simulink model "simulator_prototype_remade_v1"  (R2021b)
(part 7 of 14)

t3709 = ct{1850};
t371 = ct{1851};
t3713 = ct{1852};
t3715 = ct{1853};
t3716 = ct{1854};
t3717 = ct{1855};
t372 = ct{1856};
t3720 = ct{1857};
t3721 = ct{1858};
t3723 = ct{1859};
t3724 = ct{1860};
t3725 = ct{1861};
t3726 = ct{1862};
t3728 = ct{1863};
t3729 = ct{1864};
t373 = ct{1865};
t3730 = ct{1866};
t3732 = ct{1867};
t3733 = ct{1868};
t3734 = ct{1869};
t3735 = ct{1870};
t3736 = ct{1871};
t3737 = ct{1872};
t3738 = ct{1873};
t374 = ct{1874};
t3743 = ct{1875};
t3744 = ct{1876};
t3745 = ct{1877};
t3746 = ct{1878};
t3747 = ct{1879};
t3750 = ct{1880};
t3752 = ct{1881};
t3756 = ct{1882};
t3757 = ct{1883};
t3758 = ct{1884};
t3766 = ct{1885};
t3768 = ct{1886};
t3769 = ct{1887};
t377 = ct{1888};
t3774 = ct{1889};
t3776 = ct{1890};
t3778 = ct{1891};
t378 = ct{1892};
t3780 = ct{1893};
t3783 = ct{1894};
t3784 = ct{1895};
t3785 = ct{1896};
t3786 = ct{1897};
t3787 = ct{1898};
t3789 = ct{1899};
t379 = ct{1900};
t3792 = ct{1901};
t3795 = ct{1902};
t3798 = ct{1903};
t380 = ct{1904};
t3800 = ct{1905};
t3803 = ct{1906};
t3804 = ct{1907};
t3805 = ct{1908};
t3806 = ct{1909};
t3810 = ct{1910};
t3811 = ct{1911};
t3813 = ct{1912};
t3814 = ct{1913};
t3815 = ct{1914};
t3816 = ct{1915};
t3817 = ct{1916};
t3819 = ct{1917};
t382 = ct{1918};
t3820 = ct{1919};
t3821 = ct{1920};
t3822 = ct{1921};
t3823 = ct{1922};
t3824 = ct{1923};
t3825 = ct{1924};
t3826 = ct{1925};
t3827 = ct{1926};
t3831 = ct{1927};
t3834 = ct{1928};
t3835 = ct{1929};
t3839 = ct{1930};
t384 = ct{1931};
t3843 = ct{1932};
t3849 = ct{1933};
t3850 = ct{1934};
t3851 = ct{1935};
t3852 = ct{1936};
t3853 = ct{1937};
t3855 = ct{1938};
t3857 = ct{1939};
t3858 = ct{1940};
t386 = ct{1941};
t3866 = ct{1942};
t3867 = ct{1943};
t3869 = ct{1944};
t387 = ct{1945};
t3870 = ct{1946};
t3877 = ct{1947};
t388 = ct{1948};
t3885 = ct{1949};
t3889 = ct{1950};
t3890 = ct{1951};
t3891 = ct{1952};
t3892 = ct{1953};
t3899 = ct{1954};
t391 = ct{1955};
t3912 = ct{1956};
t3913 = ct{1957};
t3915 = ct{1958};
t3917 = ct{1959};
t392 = ct{1960};
t3929 = ct{1961};
t3930 = ct{1962};
t3941 = ct{1963};
t3946 = ct{1964};
t3949 = ct{1965};
t395 = ct{1966};
t3950 = ct{1967};
t3951 = ct{1968};
t3952 = ct{1969};
t3953 = ct{1970};
t3958 = ct{1971};
t3959 = ct{1972};
t396 = ct{1973};
t3966 = ct{1974};
t3970 = ct{1975};
t3980 = ct{1976};
t3981 = ct{1977};
t3982 = ct{1978};
t3984 = ct{1979};
t3990 = ct{1980};
t4 = ct{1981};
t400 = ct{1982};
t4004 = ct{1983};
t4005 = ct{1984};
t4006 = ct{1985};
t401 = ct{1986};
t4010 = ct{1987};
t4011 = ct{1988};
t4014 = ct{1989};
t4015 = ct{1990};
t4016 = ct{1991};
t4017 = ct{1992};
t4018 = ct{1993};
t4019 = ct{1994};
t402 = ct{1995};
t4020 = ct{1996};
t4021 = ct{1997};
t4022 = ct{1998};
t4023 = ct{1999};
t4024 = ct{2000};
t4025 = ct{2001};
t4026 = ct{2002};
t4027 = ct{2003};
t4028 = ct{2004};
t4029 = ct{2005};
t403 = ct{2006};
t4036 = ct{2007};
t4039 = ct{2008};
t4040 = ct{2009};
t4041 = ct{2010};
t4042 = ct{2011};
t4045 = ct{2012};
t4046 = ct{2013};
t4047 = ct{2014};
t4048 = ct{2015};
t4051 = ct{2016};
t4053 = ct{2017};
t4054 = ct{2018};
t406 = ct{2019};
t4062 = ct{2020};
t4063 = ct{2021};
t4064 = ct{2022};
t4065 = ct{2023};
t4068 = ct{2024};
t4069 = ct{2025};
t4070 = ct{2026};
t4071 = ct{2027};
t4073 = ct{2028};
t4074 = ct{2029};
t4075 = ct{2030};
t4089 = ct{2031};
t4099 = ct{2032};
t410 = ct{2033};
t4103 = ct{2034};
t4105 = ct{2035};
t411 = ct{2036};
t4113 = ct{2037};
t4114 = ct{2038};
t4116 = ct{2039};
t4118 = ct{2040};
t4119 = ct{2041};
t412 = ct{2042};
t4123 = ct{2043};
t4124 = ct{2044};
t4125 = ct{2045};
t413 = ct{2046};
t4132 = ct{2047};
t414 = ct{2048};
t4140 = ct{2049};
t4142 = ct{2050};
t4143 = ct{2051};
t4144 = ct{2052};
t4145 = ct{2053};
t415 = ct{2054};
t4150 = ct{2055};
t4152 = ct{2056};
t4153 = ct{2057};
t416 = ct{2058};
t4162 = ct{2059};
t4164 = ct{2060};
t4165 = ct{2061};
t4166 = ct{2062};
t4169 = ct{2063};
t417 = ct{2064};
t4171 = ct{2065};
t4173 = ct{2066};
t4174 = ct{2067};
t4177 = ct{2068};
t4178 = ct{2069};
t4179 = ct{2070};
t418 = ct{2071};
t4180 = ct{2072};
t4181 = ct{2073};
t4183 = ct{2074};
t4184 = ct{2075};
t4185 = ct{2076};
t4186 = ct{2077};
t4188 = ct{2078};
t4190 = ct{2079};
t4195 = ct{2080};
t4196 = ct{2081};
t4197 = ct{2082};
t420 = ct{2083};
t4201 = ct{2084};
t4202 = ct{2085};
t4205 = ct{2086};
t4206 = ct{2087};
t4207 = ct{2088};
t4208 = ct{2089};
t4209 = ct{2090};
t4210 = ct{2091};
t4211 = ct{2092};
t4215 = ct{2093};
t4217 = ct{2094};
t4218 = ct{2095};
t4219 = ct{2096};
t422 = ct{2097};
t4220 = ct{2098};
t4221 = ct{2099};
t4223 = ct{2100};
t4224 = ct{2101};
t4225 = ct{2102};
t4226 = ct{2103};
t4228 = ct{2104};
t4229 = ct{2105};
t423 = ct{2106};
t4230 = ct{2107};
t4231 = ct{2108};
t4232 = ct{2109};
t4233 = ct{2110};
t4234 = ct{2111};
t4235 = ct{2112};
t424 = ct{2113};
t4241 = ct{2114};
t4242 = ct{2115};
t4243 = ct{2116};
t4244 = ct{2117};
t4245 = ct{2118};
t4246 = ct{2119};
t4247 = ct{2120};
t4248 = ct{2121};
t4249 = ct{2122};
t425 = ct{2123};
t4250 = ct{2124};
t4251 = ct{2125};
t4253 = ct{2126};
t4254 = ct{2127};
t4255 = ct{2128};
t4256 = ct{2129};
t4257 = ct{2130};
t4258 = ct{2131};
t4259 = ct{2132};
t4260 = ct{2133};
t4261 = ct{2134};
t4262 = ct{2135};
t4263 = ct{2136};
t427 = ct{2137};
t4273 = ct{2138};
t4274 = ct{2139};
t4275 = ct{2140};
t4276 = ct{2141};
t4278 = ct{2142};
t4279 = ct{2143};
t428 = ct{2144};
t4280 = ct{2145};
t4281 = ct{2146};
t4282 = ct{2147};
t4283 = ct{2148};
t4284 = ct{2149};
t4285 = ct{2150};
t4286 = ct{2151};
t4287 = ct{2152};
t4289 = ct{2153};
t429 = ct{2154};
t4290 = ct{2155};
t4291 = ct{2156};
t4292 = ct{2157};
t4293 = ct{2158};
t4295 = ct{2159};
t4296 = ct{2160};
t4297 = ct{2161};
t4298 = ct{2162};
t4299 = ct{2163};
t4300 = ct{2164};
t4301 = ct{2165};
t4302 = ct{2166};
t4303 = ct{2167};
t4304 = ct{2168};
t4305 = ct{2169};
t4306 = ct{2170};
t4308 = ct{2171};
t431 = ct{2172};
t4310 = ct{2173};
t4315 = ct{2174};
t4316 = ct{2175};
t4317 = ct{2176};
t4318 = ct{2177};
t432 = ct{2178};
t4321 = ct{2179};
t4323 = ct{2180};
t4324 = ct{2181};
t4325 = ct{2182};
t4326 = ct{2183};
t4327 = ct{2184};
t4328 = ct{2185};
t4329 = ct{2186};
t433 = ct{2187};
t4330 = ct{2188};
t4331 = ct{2189};
t4332 = ct{2190};
t4333 = ct{2191};
t4334 = ct{2192};
t4335 = ct{2193};
t4336 = ct{2194};
t4337 = ct{2195};
t4338 = ct{2196};
t4339 = ct{2197};
t434 = ct{2198};
t4340 = ct{2199};
t4342 = ct{2200};
t4344 = ct{2201};
t4345 = ct{2202};
t4346 = ct{2203};
t4347 = ct{2204};
t4348 = ct{2205};
t4349 = ct{2206};
t435 = ct{2207};
t4350 = ct{2208};
t4354 = ct{2209};
t4356 = ct{2210};
t4357 = ct{2211};
t436 = ct{2212};
t4362 = ct{2213};
t4363 = ct{2214};
t4365 = ct{2215};
t4366 = ct{2216};
t4368 = ct{2217};
t4369 = ct{2218};
t437 = ct{2219};
t4370 = ct{2220};
t4371 = ct{2221};
t4372 = ct{2222};
t4373 = ct{2223};
t4374 = ct{2224};
t4375 = ct{2225};
t4376 = ct{2226};
t4377 = ct{2227};
t4379 = ct{2228};
t438 = ct{2229};
t4380 = ct{2230};
t4382 = ct{2231};
t4383 = ct{2232};
t4384 = ct{2233};
t4385 = ct{2234};
t4386 = ct{2235};
t4387 = ct{2236};
t4388 = ct{2237};
t4389 = ct{2238};
t439 = ct{2239};
t4391 = ct{2240};
t4392 = ct{2241};
t4394 = ct{2242};
t4395 = ct{2243};
t4396 = ct{2244};
t4397 = ct{2245};
t4398 = ct{2246};
t4399 = ct{2247};
t44 = ct{2248};
t440 = ct{2249};
t4400 = ct{2250};
t4401 = ct{2251};
t4402 = ct{2252};
t4403 = ct{2253};
t4404 = ct{2254};
t4405 = ct{2255};
t4406 = ct{2256};
t4407 = ct{2257};
t4408 = ct{2258};
t4409 = ct{2259};
t441 = ct{2260};
t4410 = ct{2261};
t4411 = ct{2262};
t4412 = ct{2263};
t4413 = ct{2264};
t4414 = ct{2265};
t4415 = ct{2266};
t4416 = ct{2267};
t4417 = ct{2268};
t4418 = ct{2269};
t4419 = ct{2270};
t442 = ct{2271};
t4420 = ct{2272};
t4421 = ct{2273};
t4422 = ct{2274};
t4423 = ct{2275};
t4424 = ct{2276};
t4425 = ct{2277};
t4426 = ct{2278};
t4427 = ct{2279};
t4428 = ct{2280};
t4429 = ct{2281};
t4430 = ct{2282};
t4431 = ct{2283};
t4432 = ct{2284};
t4433 = ct{2285};
t4434 = ct{2286};
t4435 = ct{2287};
t4436 = ct{2288};
t4437 = ct{2289};
t4438 = ct{2290};
t4439 = ct{2291};
t444 = ct{2292};
t4440 = ct{2293};
t4442 = ct{2294};
t4444 = ct{2295};
t4445 = ct{2296};
t4446 = ct{2297};
t4447 = ct{2298};
t4448 = ct{2299};
t4449 = ct{2300};
t445 = ct{2301};
t4450 = ct{2302};
t4451 = ct{2303};
t4453 = ct{2304};
t4454 = ct{2305};
t4455 = ct{2306};
t4460 = ct{2307};
t4461 = ct{2308};
t4462 = ct{2309};
t4463 = ct{2310};
t4464 = ct{2311};
t4465 = ct{2312};
t4466 = ct{2313};
t4467 = ct{2314};
t4468 = ct{2315};
t4469 = ct{2316};
t4470 = ct{2317};
t4471 = ct{2318};
t4473 = ct{2319};
t4474 = ct{2320};
t4475 = ct{2321};
t4476 = ct{2322};
t4477 = ct{2323};
t4478 = ct{2324};
t4479 = ct{2325};
t448 = ct{2326};
t4481 = ct{2327};
t4482 = ct{2328};
t4483 = ct{2329};
t4484 = ct{2330};
t4485 = ct{2331};
t4486 = ct{2332};
t4487 = ct{2333};
t4488 = ct{2334};
t4489 = ct{2335};
t449 = ct{2336};
t4490 = ct{2337};
t4493 = ct{2338};
t4494 = ct{2339};
t4495 = ct{2340};
t4496 = ct{2341};
t4497 = ct{2342};
t4498 = ct{2343};
t4499 = ct{2344};
t45 = ct{2345};
t450 = ct{2346};
t4500 = ct{2347};
t4501 = ct{2348};
t4502 = ct{2349};
t4503 = ct{2350};
t4504 = ct{2351};
t4505 = ct{2352};
t4506 = ct{2353};
t4507 = ct{2354};
t4508 = ct{2355};
t4509 = ct{2356};
t4510 = ct{2357};
t4512 = ct{2358};
t4513 = ct{2359};
t4514 = ct{2360};
t4515 = ct{2361};
t4516 = ct{2362};
t4518 = ct{2363};
t4519 = ct{2364};
t452 = ct{2365};
t4520 = ct{2366};
t4521 = ct{2367};
t4522 = ct{2368};
t4523 = ct{2369};
t4524 = ct{2370};
t4525 = ct{2371};
t4526 = ct{2372};
t4527 = ct{2373};
t4529 = ct{2374};
t453 = ct{2375};
t4530 = ct{2376};
t4531 = ct{2377};
t4532 = ct{2378};
t4534 = ct{2379};
t4535 = ct{2380};
t4537 = ct{2381};
t4538 = ct{2382};
t4539 = ct{2383};
t454 = ct{2384};
t4541 = ct{2385};
t4543 = ct{2386};
t4544 = ct{2387};
t4545 = ct{2388};
t4546 = ct{2389};
t4547 = ct{2390};
t4549 = ct{2391};
t4550 = ct{2392};
t4551 = ct{2393};
t4552 = ct{2394};
t4553 = ct{2395};
t4554 = ct{2396};
t4556 = ct{2397};
t4557 = ct{2398};
t4558 = ct{2399};
t4559 = ct{2400};
t4560 = ct{2401};
t4564 = ct{2402};
t4565 = ct{2403};
t4566 = ct{2404};
t4567 = ct{2405};
t4568 = ct{2406};
t4569 = ct{2407};
t457 = ct{2408};
t4570 = ct{2409};
t4572 = ct{2410};
t4573 = ct{2411};
t4575 = ct{2412};
t4576 = ct{2413};
t4577 = ct{2414};
t4578 = ct{2415};
t458 = ct{2416};
t4580 = ct{2417};
t4581 = ct{2418};
t4582 = ct{2419};
t4584 = ct{2420};
t4586 = ct{2421};
t4587 = ct{2422};
t4588 = ct{2423};
t4589 = ct{2424};
t459 = ct{2425};
t4590 = ct{2426};
t4591 = ct{2427};
t4592 = ct{2428};
t4593 = ct{2429};
t4594 = ct{2430};
t4595 = ct{2431};
t4596 = ct{2432};
t4597 = ct{2433};
t4598 = ct{2434};
t4599 = ct{2435};
t46 = ct{2436};
t460 = ct{2437};
t4600 = ct{2438};
t4601 = ct{2439};
t4602 = ct{2440};
t4603 = ct{2441};
t4604 = ct{2442};
t4605 = ct{2443};
t4606 = ct{2444};
t4607 = ct{2445};
t4608 = ct{2446};
t4609 = ct{2447};
t461 = ct{2448};
t4610 = ct{2449};
t4612 = ct{2450};
t4613 = ct{2451};
t4614 = ct{2452};
t4615 = ct{2453};
t4616 = ct{2454};
t4617 = ct{2455};
t4618 = ct{2456};
t4619 = ct{2457};
t462 = ct{2458};
t4620 = ct{2459};
t4621 = ct{2460};
t4622 = ct{2461};
t4623 = ct{2462};
t4624 = ct{2463};
t4625 = ct{2464};
t4626 = ct{2465};
t4627 = ct{2466};
t4629 = ct{2467};
t463 = ct{2468};
t4631 = ct{2469};
t4632 = ct{2470};
t4633 = ct{2471};
t4634 = ct{2472};
t4635 = ct{2473};
t4636 = ct{2474};
t4637 = ct{2475};
t4638 = ct{2476};
t4639 = ct{2477};
t464 = ct{2478};
t4640 = ct{2479};
t4643 = ct{2480};
t4644 = ct{2481};
t4645 = ct{2482};
t4646 = ct{2483};
t4647 = ct{2484};
t4649 = ct{2485};
t465 = ct{2486};
t4650 = ct{2487};
t4652 = ct{2488};
t4653 = ct{2489};
t4654 = ct{2490};
t4655 = ct{2491};
t4656 = ct{2492};
t4657 = ct{2493};
t4659 = ct{2494};
t466 = ct{2495};
t4660 = ct{2496};
t4661 = ct{2497};
t4662 = ct{2498};
t4663 = ct{2499};
t4664 = ct{2500};
t4665 = ct{2501};
t4666 = ct{2502};
t4667 = ct{2503};
t4668 = ct{2504};
t4669 = ct{2505};
t4670 = ct{2506};
t4671 = ct{2507};
t4672 = ct{2508};
t4673 = ct{2509};
t4674 = ct{2510};
t4675 = ct{2511};
t4676 = ct{2512};
t4677 = ct{2513};
t4678 = ct{2514};
t4679 = ct{2515};
t468 = ct{2516};
t4680 = ct{2517};
t4681 = ct{2518};
t4682 = ct{2519};
t4683 = ct{2520};
t4684 = ct{2521};
t4685 = ct{2522};
t4686 = ct{2523};
t4687 = ct{2524};
t4689 = ct{2525};
t469 = ct{2526};
t4692 = ct{2527};
t4693 = ct{2528};
t4694 = ct{2529};
t4695 = ct{2530};
t4696 = ct{2531};
t4697 = ct{2532};
t4698 = ct{2533};
t4699 = ct{2534};
t47 = ct{2535};
t470 = ct{2536};
t4700 = ct{2537};
t4702 = ct{2538};
t4703 = ct{2539};
t4704 = ct{2540};
t4707 = ct{2541};
t4708 = ct{2542};
t4709 = ct{2543};
t471 = ct{2544};
t4710 = ct{2545};
t4711 = ct{2546};
t4712 = ct{2547};
t4713 = ct{2548};
t4714 = ct{2549};
t4715 = ct{2550};
t4716 = ct{2551};
t4717 = ct{2552};
t4718 = ct{2553};
t4719 = ct{2554};
t472 = ct{2555};
t4720 = ct{2556};
t4721 = ct{2557};
t4722 = ct{2558};
t4723 = ct{2559};
t4724 = ct{2560};
t4725 = ct{2561};
t4726 = ct{2562};
t4727 = ct{2563};
t4728 = ct{2564};
t4729 = ct{2565};
t4730 = ct{2566};
t4731 = ct{2567};
t4732 = ct{2568};
t4733 = ct{2569};
t4734 = ct{2570};
t4736 = ct{2571};
t4737 = ct{2572};
t4738 = ct{2573};
t4739 = ct{2574};
t4740 = ct{2575};
t4742 = ct{2576};
t4745 = ct{2577};
t4746 = ct{2578};
t4747 = ct{2579};
t4748 = ct{2580};
t475 = ct{2581};
t4750 = ct{2582};
t4751 = ct{2583};
t4753 = ct{2584};
t4754 = ct{2585};
t4755 = ct{2586};
t4756 = ct{2587};
t4757 = ct{2588};
t4762 = ct{2589};
t4763 = ct{2590};
t4765 = ct{2591};
t4768 = ct{2592};
t477 = ct{2593};
t4771 = ct{2594};
t4772 = ct{2595};
t4773 = ct{2596};
t4774 = ct{2597};
t4775 = ct{2598};
t4776 = ct{2599};
t4779 = ct{2600};
t4780 = ct{2601};
t4781 = ct{2602};
t4782 = ct{2603};
t4783 = ct{2604};
t4784 = ct{2605};
t4785 = ct{2606};
t4786 = ct{2607};
t4787 = ct{2608};
t4788 = ct{2609};
t4789 = ct{2610};
t479 = ct{2611};
t4790 = ct{2612};
t4791 = ct{2613};
t4792 = ct{2614};
t4793 = ct{2615};
t4794 = ct{2616};
t4795 = ct{2617};
t4797 = ct{2618};
t4799 = ct{2619};
t480 = ct{2620};
t4800 = ct{2621};
t4801 = ct{2622};
t4802 = ct{2623};
t4803 = ct{2624};
t4805 = ct{2625};
t4806 = ct{2626};
t4809 = ct{2627};
t481 = ct{2628};
t4810 = ct{2629};
t4811 = ct{2630};
t4812 = ct{2631};
t4813 = ct{2632};
t4814 = ct{2633};
t4818 = ct{2634};
t4819 = ct{2635};
t482 = ct{2636};
t4820 = ct{2637};
t4821 = ct{2638};
t4824 = ct{2639};
t4825 = ct{2640};
t4826 = ct{2641};
t4827 = ct{2642};
t4829 = ct{2643};
t483 = ct{2644};
t4831 = ct{2645};
t4833 = ct{2646};
t4834 = ct{2647};
t4835 = ct{2648};
t4837 = ct{2649};
t484 = ct{2650};
t4840 = ct{2651};
t4841 = ct{2652};
t4842 = ct{2653};
t4845 = ct{2654};
t4846 = ct{2655};
t4847 = ct{2656};
t4848 = ct{2657};
t485 = ct{2658};
t4851 = ct{2659};
t4853 = ct{2660};
t4856 = ct{2661};
t4857 = ct{2662};
t486 = ct{2663};
t4862 = ct{2664};
t4863 = ct{2665};
t4864 = ct{2666};
t4865 = ct{2667};
t4866 = ct{2668};
t4867 = ct{2669};
t4868 = ct{2670};
t4869 = ct{2671};
t4870 = ct{2672};
t4872 = ct{2673};
t4873 = ct{2674};
t4874 = ct{2675};
t4875 = ct{2676};
t4876 = ct{2677};
t4877 = ct{2678};
t488 = ct{2679};
t4880 = ct{2680};
t4884 = ct{2681};
t4888 = ct{2682};
t489 = ct{2683};
t4893 = ct{2684};
t4895 = ct{2685};
t4903 = ct{2686};
t4904 = ct{2687};
t4907 = ct{2688};
t4908 = ct{2689};
t491 = ct{2690};
t4911 = ct{2691};
t4913 = ct{2692};
t4914 = ct{2693};
t4919 = ct{2694};
t492 = ct{2695};
t4920 = ct{2696};
t4922 = ct{2697};
t4924 = ct{2698};
t4925 = ct{2699};
t4927 = ct{2700};
t4928 = ct{2701};
t4929 = ct{2702};
t493 = ct{2703};
t4931 = ct{2704};
t4933 = ct{2705};
t4934 = ct{2706};
t4935 = ct{2707};
t4936 = ct{2708};
t494 = ct{2709};
t4942 = ct{2710};
t4943 = ct{2711};
t4944 = ct{2712};
t4946 = ct{2713};
t4948 = ct{2714};
t4949 = ct{2715};
t4950 = ct{2716};
t4951 = ct{2717};
t4952 = ct{2718};
t4953 = ct{2719};
t4957 = ct{2720};
t496 = ct{2721};
t4963 = ct{2722};
t4964 = ct{2723};
t4969 = ct{2724};
t497 = ct{2725};
t4970 = ct{2726};
t4973 = ct{2727};
t4974 = ct{2728};
t4975 = ct{2729};
t4976 = ct{2730};
t4978 = ct{2731};
t4979 = ct{2732};
t498 = ct{2733};
t4981 = ct{2734};
t4982 = ct{2735};
t4983 = ct{2736};
t4987 = ct{2737};
t4988 = ct{2738};
t4989 = ct{2739};
t499 = ct{2740};
t4990 = ct{2741};
t4991 = ct{2742};
t4992 = ct{2743};
t4993 = ct{2744};
t4994 = ct{2745};
t4995 = ct{2746};
t4996 = ct{2747};
t5 = ct{2748};
t50 = ct{2749};
t500 = ct{2750};
t5000 = ct{2751};
t5001 = ct{2752};
t5002 = ct{2753};
t5003 = ct{2754};
t5005 = ct{2755};
t5006 = ct{2756};
t5007 = ct{2757};
t5008 = ct{2758};
t5009 = ct{2759};
t501 = ct{2760};
t5010 = ct{2761};
t5014 = ct{2762};
t5015 = ct{2763};
t5016 = ct{2764};
t5017 = ct{2765};
t5018 = ct{2766};
t5019 = ct{2767};
t502 = ct{2768};
t5020 = ct{2769};
t5021 = ct{2770};
t5022 = ct{2771};
t5023 = ct{2772};
t5024 = ct{2773};
t5026 = ct{2774};
t5027 = ct{2775};
t5029 = ct{2776};
t503 = ct{2777};
t5030 = ct{2778};
t5031 = ct{2779};
t5032 = ct{2780};
t5035 = ct{2781};
t5036 = ct{2782};
t5039 = ct{2783};
t504 = ct{2784};
t5041 = ct{2785};
t5045 = ct{2786};
t5048 = ct{2787};
t505 = ct{2788};
t5051 = ct{2789};
t5054 = ct{2790};
t5055 = ct{2791};
t5056 = ct{2792};
t5058 = ct{2793};
t5059 = ct{2794};
t506 = ct{2795};
t5061 = ct{2796};
t5063 = ct{2797};
t5064 = ct{2798};
t5065 = ct{2799};
t5066 = ct{2800};
t5067 = ct{2801};
t507 = ct{2802};
t5073 = ct{2803};
t5074 = ct{2804};
t5075 = ct{2805};
t5076 = ct{2806};
t5077 = ct{2807};
t5078 = ct{2808};
t508 = ct{2809};
t5080 = ct{2810};
t5081 = ct{2811};
t5083 = ct{2812};
t5084 = ct{2813};
t5085 = ct{2814};
t5088 = ct{2815};
t5089 = ct{2816};
t509 = ct{2817};
t5090 = ct{2818};
t5091 = ct{2819};
t5093 = ct{2820};
t5095 = ct{2821};
t5097 = ct{2822};
t5098 = ct{2823};
t5099 = ct{2824};
t510 = ct{2825};
t5100 = ct{2826};
t5101 = ct{2827};
t5102 = ct{2828};
t5107 = ct{2829};
t5109 = ct{2830};
t511 = ct{2831};
t5110 = ct{2832};
t5112 = ct{2833};
t5113 = ct{2834};
t5114 = ct{2835};
t5119 = ct{2836};
t512 = ct{2837};
t5120 = ct{2838};
t5121 = ct{2839};
t5123 = ct{2840};
t5125 = ct{2841};
t513 = ct{2842};
t5131 = ct{2843};
t5132 = ct{2844};
t5136 = ct{2845};
t5138 = ct{2846};
t5139 = ct{2847};
t514 = ct{2848};
t5140 = ct{2849};
t5143 = ct{2850};
t5146 = ct{2851};
t5147 = ct{2852};
t5148 = ct{2853};
t5150 = ct{2854};
t5151 = ct{2855};
t5152 = ct{2856};
t5153 = ct{2857};
t5154 = ct{2858};
t5157 = ct{2859};
t5158 = ct{2860};
t516 = ct{2861};
t5164 = ct{2862};
t5166 = ct{2863};
t517 = ct{2864};
t5171 = ct{2865};
t5172 = ct{2866};
t5174 = ct{2867};
t5175 = ct{2868};
t518 = ct{2869};
t5180 = ct{2870};
t5181 = ct{2871};
t5183 = ct{2872};
t5184 = ct{2873};
t5185 = ct{2874};
t5187 = ct{2875};
t5189 = ct{2876};
t5191 = ct{2877};
t5195 = ct{2878};
t5199 = ct{2879};
t520 = ct{2880};
t5200 = ct{2881};
t5201 = ct{2882};
t5202 = ct{2883};
t5203 = ct{2884};
t5204 = ct{2885};
t5205 = ct{2886};
t5206 = ct{2887};
t5207 = ct{2888};
t5209 = ct{2889};
t521 = ct{2890};
t5210 = ct{2891};
t5211 = ct{2892};
t5215 = ct{2893};
t5216 = ct{2894};
t5217 = ct{2895};
t5218 = ct{2896};
t5219 = ct{2897};
t522 = ct{2898};
t5222 = ct{2899};
t5223 = ct{2900};
t5224 = ct{2901};
t5227 = ct{2902};
t5229 = ct{2903};
t523 = ct{2904};
t5233 = ct{2905};
t5236 = ct{2906};
t5237 = ct{2907};
t5238 = ct{2908};
t5239 = ct{2909};
t524 = ct{2910};
t5240 = ct{2911};
t5242 = ct{2912};
t5244 = ct{2913};
t5247 = ct{2914};
t5248 = ct{2915};
t5249 = ct{2916};
t525 = ct{2917};
t5251 = ct{2918};
t5252 = ct{2919};
t5255 = ct{2920};
t5257 = ct{2921};
t5258 = ct{2922};
t526 = ct{2923};
t5261 = ct{2924};
t5262 = ct{2925};
t5265 = ct{2926};
t5268 = ct{2927};
t5269 = ct{2928};
t527 = ct{2929};
t5270 = ct{2930};
t5272 = ct{2931};
t5279 = ct{2932};
t528 = ct{2933};
t5280 = ct{2934};
t5285 = ct{2935};
t5288 = ct{2936};
t529 = ct{2937};
t5292 = ct{2938};
t5293 = ct{2939};
t5294 = ct{2940};
t5295 = ct{2941};
t5297 = ct{2942};
t53 = ct{2943};
t530 = ct{2944};
t5302 = ct{2945};
t5306 = ct{2946};
t531 = ct{2947};
t5318 = ct{2948};
t532 = ct{2949};
t5320 = ct{2950};
t5321 = ct{2951};
t5324 = ct{2952};
t5327 = ct{2953};
t533 = ct{2954};
t5331 = ct{2955};
t5332 = ct{2956};
t5339 = ct{2957};
t534 = ct{2958};
t5344 = ct{2959};
t5346 = ct{2960};
t5347 = ct{2961};
t5348 = ct{2962};
t5349 = ct{2963};
t535 = ct{2964};
t5351 = ct{2965};
t5355 = ct{2966};
t5356 = ct{2967};
t5358 = ct{2968};
t536 = ct{2969};
t5361 = ct{2970};
t5364 = ct{2971};
t5365 = ct{2972};
t5367 = ct{2973};
t5368 = ct{2974};
t537 = ct{2975};
t5372 = ct{2976};
t5373 = ct{2977};
t5375 = ct{2978};
t5378 = ct{2979};
t538 = ct{2980};
t5383 = ct{2981};
t5387 = ct{2982};
t5389 = ct{2983};
t539 = ct{2984};
t5390 = ct{2985};
t5391 = ct{2986};
t5392 = ct{2987};
t5393 = ct{2988};
t5394 = ct{2989};
t5395 = ct{2990};
t540 = ct{2991};
t5402 = ct{2992};
t5404 = ct{2993};
t5409 = ct{2994};
t5416 = ct{2995};
t5420 = ct{2996};
t543 = ct{2997};
t5433 = ct{2998};
t5435 = ct{2999};
t5436 = ct{3000};
t544 = ct{3001};
t5440 = ct{3002};
t5441 = ct{3003};
t5442 = ct{3004};
t5443 = ct{3005};
t5444 = ct{3006};
t5445 = ct{3007};
t5446 = ct{3008};
t5448 = ct{3009};
t545 = ct{3010};
t5450 = ct{3011};
t5451 = ct{3012};
t5453 = ct{3013};
t5454 = ct{3014};
t5457 = ct{3015};
t5459 = ct{3016};
t546 = ct{3017};
t5463 = ct{3018};
t5464 = ct{3019};
t5465 = ct{3020};
t5466 = ct{3021};
t547 = ct{3022};
t5473 = ct{3023};
t5475 = ct{3024};
t5479 = ct{3025};
t548 = ct{3026};
t5480 = ct{3027};
t5481 = ct{3028};
t5482 = ct{3029};
t5483 = ct{3030};
t5484 = ct{3031};
t5485 = ct{3032};
t5486 = ct{3033};
t5487 = ct{3034};
t5488 = ct{3035};
t5489 = ct{3036};
t549 = ct{3037};
t5490 = ct{3038};
t5491 = ct{3039};
t5492 = ct{3040};
t5493 = ct{3041};
t5494 = ct{3042};
t5496 = ct{3043};
t5498 = ct{3044};
t5499 = ct{3045};
t5501 = ct{3046};
t5507 = ct{3047};
t551 = ct{3048};
t5512 = ct{3049};
t5516 = ct{3050};
t5517 = ct{3051};
t5519 = ct{3052};
t552 = ct{3053};
t5521 = ct{3054};
t5522 = ct{3055};
t5526 = ct{3056};
t5527 = ct{3057};
t553 = ct{3058};
t5534 = ct{3059};
t554 = ct{3060};
t5540 = ct{3061};
t5546 = ct{3062};
t5549 = ct{3063};
t555 = ct{3064};
t5552 = ct{3065};
t5555 = ct{3066};
t5559 = ct{3067};
t556 = ct{3068};
t5561 = ct{3069};
t5562 = ct{3070};
t5563 = ct{3071};
t5565 = ct{3072};
t5566 = ct{3073};
t5569 = ct{3074};
t557 = ct{3075};
t5573 = ct{3076};
t5578 = ct{3077};
t558 = ct{3078};
t5580 = ct{3079};
t5581 = ct{3080};
t5583 = ct{3081};
t5584 = ct{3082};
t5589 = ct{3083};
t559 = ct{3084};
t5590 = ct{3085};
t5593 = ct{3086};
t5594 = ct{3087};
t5596 = ct{3088};
t5597 = ct{3089};
t560 = ct{3090};
t5600 = ct{3091};
t5603 = ct{3092};
t5604 = ct{3093};
t5606 = ct{3094};
t5607 = ct{3095};
t561 = ct{3096};
t5611 = ct{3097};
t5612 = ct{3098};
t5618 = ct{3099};
t562 = ct{3100};
t5629 = ct{3101};
t563 = ct{3102};
t5633 = ct{3103};
t5634 = ct{3104};
t5635 = ct{3105};
t564 = ct{3106};
t5656 = ct{3107};
t5660 = ct{3108};
t5667 = ct{3109};
t5668 = ct{3110};
t567 = ct{3111};
t5673 = ct{3112};
t5678 = ct{3113};
t568 = ct{3114};
t5688 = ct{3115};
t569 = ct{3116};
t57 = ct{3117};
t570 = ct{3118};
t571 = ct{3119};
t572 = ct{3120};
t573 = ct{3121};
t574 = ct{3122};
t5741 = ct{3123};
t5743 = ct{3124};
t576 = ct{3125};
t577 = ct{3126};
t5777 = ct{3127};
t5779 = ct{3128};
t578 = ct{3129};
t5780 = ct{3130};
t5782 = ct{3131};
t579 = ct{3132};
t58 = ct{3133};
t580 = ct{3134};
t581 = ct{3135};
t5818 = ct{3136};
t5819 = ct{3137};
t582 = ct{3138};
t5823 = ct{3139};
t5826 = ct{3140};
t583 = ct{3141};
t584 = ct{3142};
t586 = ct{3143};
t587 = ct{3144};
t5886 = ct{3145};
t5887 = ct{3146};
t589 = ct{3147};
t5894 = ct{3148};
t59 = ct{3149};
t590 = ct{3150};
t591 = ct{3151};
t592 = ct{3152};
t593 = ct{3153};
t594 = ct{3154};
t595 = ct{3155};
t596 = ct{3156};
t597 = ct{3157};
t6 = ct{3158};
t60 = ct{3159};
t600 = ct{3160};
t602 = ct{3161};
t603 = ct{3162};
t604 = ct{3163};
t605 = ct{3164};
t609 = ct{3165};
t610 = ct{3166};
t611 = ct{3167};
t612 = ct{3168};
t613 = ct{3169};
t614 = ct{3170};
t615 = ct{3171};
t616 = ct{3172};
t618 = ct{3173};
t619 = ct{3174};
t620 = ct{3175};
t621 = ct{3176};
t622 = ct{3177};
t623 = ct{3178};
t624 = ct{3179};
t625 = ct{3180};
t626 = ct{3181};
t627 = ct{3182};
t628 = ct{3183};
t629 = ct{3184};
t63 = ct{3185};
t630 = ct{3186};
t631 = ct{3187};
t632 = ct{3188};
t633 = ct{3189};
t634 = ct{3190};
t635 = ct{3191};
t636 = ct{3192};
t637 = ct{3193};
t638 = ct{3194};
t639 = ct{3195};
t640 = ct{3196};
t641 = ct{3197};
t642 = ct{3198};
t643 = ct{3199};
t645 = ct{3200};
t646 = ct{3201};
t647 = ct{3202};
t648 = ct{3203};
t649 = ct{3204};
t650 = ct{3205};
t653 = ct{3206};
t654 = ct{3207};
t655 = ct{3208};
t656 = ct{3209};
t657 = ct{3210};
t658 = ct{3211};
t660 = ct{3212};
t662 = ct{3213};
t663 = ct{3214};
t664 = ct{3215};
t665 = ct{3216};
t667 = ct{3217};
t668 = ct{3218};
t669 = ct{3219};
t673 = ct{3220};
t674 = ct{3221};
t675 = ct{3222};
t676 = ct{3223};
t679 = ct{3224};
t680 = ct{3225};
t681 = ct{3226};
t682 = ct{3227};
t683 = ct{3228};
t684 = ct{3229};
t685 = ct{3230};
t686 = ct{3231};
t687 = ct{3232};
t688 = ct{3233};
t689 = ct{3234};
t691 = ct{3235};
t692 = ct{3236};
t693 = ct{3237};
t694 = ct{3238};
t695 = ct{3239};
t696 = ct{3240};
t697 = ct{3241};
t698 = ct{3242};
t7 = ct{3243};
t700 = ct{3244};
t702 = ct{3245};
t703 = ct{3246};
t704 = ct{3247};
t705 = ct{3248};
t706 = ct{3249};
t708 = ct{3250};
t71 = ct{3251};
t710 = ct{3252};
t711 = ct{3253};
t712 = ct{3254};
t713 = ct{3255};
t7148 = ct{3256};
t715 = ct{3257};
t716 = ct{3258};
t72 = ct{3259};
t724 = ct{3260};
t728 = ct{3261};
t73 = ct{3262};
t731 = ct{3263};
t733 = ct{3264};
t734 = ct{3265};
t735 = ct{3266};
t736 = ct{3267};
t738 = ct{3268};
t739 = ct{3269};
t74 = ct{3270};
t740 = ct{3271};
t741 = ct{3272};
t742 = ct{3273};
t743 = ct{3274};
t744 = ct{3275};
t746 = ct{3276};
t747 = ct{3277};
t748 = ct{3278};
t749 = ct{3279};
t75 = ct{3280};
t750 = ct{3281};
t751 = ct{3282};
t752 = ct{3283};
t753 = ct{3284};
t754 = ct{3285};
t755 = ct{3286};
t756 = ct{3287};
t757 = ct{3288};
t758 = ct{3289};
t759 = ct{3290};
t76 = ct{3291};
t760 = ct{3292};
t762 = ct{3293};
t763 = ct{3294};
t764 = ct{3295};
t765 = ct{3296};
t766 = ct{3297};
t767 = ct{3298};
t768 = ct{3299};
t769 = ct{3300};
t77 = ct{3301};
t772 = ct{3302};
t773 = ct{3303};
t774 = ct{3304};
t775 = ct{3305};
t776 = ct{3306};
t777 = ct{3307};
t778 = ct{3308};
t779 = ct{3309};
t780 = ct{3310};
t781 = ct{3311};
t782 = ct{3312};
t784 = ct{3313};
t785 = ct{3314};
t786 = ct{3315};
t792 = ct{3316};
t794 = ct{3317};
t795 = ct{3318};
t796 = ct{3319};
t797 = ct{3320};
t798 = ct{3321};
t799 = ct{3322};
t8 = ct{3323};
t80 = ct{3324};
t801 = ct{3325};
t802 = ct{3326};
t804 = ct{3327};
t805 = ct{3328};
t806 = ct{3329};
t808 = ct{3330};
t81 = ct{3331};
t814 = ct{3332};
t815 = ct{3333};
t817 = ct{3334};
t82 = ct{3335};
t820 = ct{3336};
t822 = ct{3337};
t823 = ct{3338};
t824 = ct{3339};
t825 = ct{3340};
t826 = ct{3341};
t827 = ct{3342};
t829 = ct{3343};
t83 = ct{3344};
t830 = ct{3345};
t831 = ct{3346};
t832 = ct{3347};
t833 = ct{3348};
t834 = ct{3349};
t835 = ct{3350};
t836 = ct{3351};
t837 = ct{3352};
t838 = ct{3353};
t84 = ct{3354};
t840 = ct{3355};
t841 = ct{3356};
t842 = ct{3357};
t843 = ct{3358};
t844 = ct{3359};
t845 = ct{3360};
t846 = ct{3361};
t847 = ct{3362};
t852 = ct{3363};
t853 = ct{3364};
t856 = ct{3365};
t858 = ct{3366};
t859 = ct{3367};
t86 = ct{3368};
t861 = ct{3369};
t863 = ct{3370};
t865 = ct{3371};
t866 = ct{3372};
t867 = ct{3373};
t868 = ct{3374};
t869 = ct{3375};
t870 = ct{3376};
t874 = ct{3377};
t875 = ct{3378};
t876 = ct{3379};
t877 = ct{3380};
t878 = ct{3381};
t880 = ct{3382};
t881 = ct{3383};
t882 = ct{3384};
t884 = ct{3385};
t885 = ct{3386};
t888 = ct{3387};
t891 = ct{3388};
t895 = ct{3389};
t899 = ct{3390};
t9 = ct{3391};
t90 = ct{3392};
t900 = ct{3393};
t902 = ct{3394};
t903 = ct{3395};
t906 = ct{3396};
t909 = ct{3397};
t91 = ct{3398};
t910 = ct{3399};
t911 = ct{3400};
t914 = ct{3401};
t916 = ct{3402};
t917 = ct{3403};
t920 = ct{3404};
t921 = ct{3405};
t922 = ct{3406};
t923 = ct{3407};
t925 = ct{3408};
t926 = ct{3409};
t927 = ct{3410};
t928 = ct{3411};
t929 = ct{3412};
t930 = ct{3413};
t934 = ct{3414};
t935 = ct{3415};
t937 = ct{3416};
t940 = ct{3417};
t941 = ct{3418};
t942 = ct{3419};
t943 = ct{3420};
t944 = ct{3421};
t945 = ct{3422};
t946 = ct{3423};
t947 = ct{3424};
t949 = ct{3425};
t95 = ct{3426};
t950 = ct{3427};
t951 = ct{3428};
t952 = ct{3429};
t953 = ct{3430};
t954 = ct{3431};
t955 = ct{3432};
t957 = ct{3433};
t958 = ct{3434};
t961 = ct{3435};
t962 = ct{3436};
t963 = ct{3437};
t964 = ct{3438};
t965 = ct{3439};
t968 = ct{3440};
t97 = ct{3441};
t970 = ct{3442};
t971 = ct{3443};
t972 = ct{3444};
t973 = ct{3445};
t974 = ct{3446};
t975 = ct{3447};
t976 = ct{3448};
t977 = ct{3449};
t982 = ct{3450};
t983 = ct{3451};
t984 = ct{3452};
t986 = ct{3453};
t987 = ct{3454};
t988 = ct{3455};
t989 = ct{3456};
t99 = ct{3457};
t991 = ct{3458};
t993 = ct{3459};
t994 = ct{3460};
t995 = ct{3461};
t999 = ct{3462};
t1723 = -t1649;
t1741 = -t1665;
t1747 = t202.*6.45106415957158e-10;
t1753 = t7.*t199.*3.023531158253378e-8;
t1754 = t5.*t9.*t199.*4.188279553614573e-7;
t1765 = t5.*t199.*(-2.227142959217101e-7);
t1766 = t5.*t199.*(-1.11357147960855e-7);
t1768 = t8.*t9.*t201.*4.454285918434201e-7;
t1777 = t5.*t9.*t201.*1.274380648825446e-6;
t1781 = -t1706;
t1790 = t8.*t19.*t201.*8.376559107229145e-7;
t1794 = t7.*t9.*t200.*1.378434177095879e-6;
t1805 = t7.*t8.*t199.*1.435017073119793e-6;
t1815 = -t1719;
t1845 = t19.*t199.*6.371903244127231e-7;
t1846 = t19.*t199.*1.274380648825446e-6;
t1848 = t18.*t1551;
t1853 = -t1743;
t1856 = t17.*t1557;
t1861 = t19.*t202.*6.371903244127231e-7;
t1885 = -t1773;
t1886 = -t1775;
t1891 = -t1782;
t1900 = -t1792;
t1902 = t5.*t7.*t9.*t200.*2.817872251232979e-6;
t1905 = -t1802;
t1917 = t199.*3.179500557904044e-7;
t1918 = t199.*6.359001115808088e-7;
t1927 = t5.*t200.*1.608000198040319e-13;
t1928 = -t1825;
t1934 = t202.*3.179500557904044e-7;
t1942 = t199.*3.173049493744472e-7;
t1947 = t18.*t1590;
t1951 = -t1854;
t1952 = t7.*t200.*4.340272528010248e-9;
t1953 = -t1862;
t1954 = t23.*t1590;
t1975 = t18.*t1665;
t1982 = t18.*t1671;
t1983 = t7.*t19.*t200.*4.287013106293682e-6;
t1985 = t18.*t1673;
t1986 = t5.*t7.*t8.*t199.*1.378434177095879e-6;
t1987 = -t1880;
t1989 = t9.*t201.*t306;
t1991 = t18.*t1615;
t2011 = -t1904;
t2015 = t17.*t1624;
t2018 = t18.*t1627;
t2026 = t5.*t200.*8.040000990201593e-14;
t2027 = t5.*t201.*8.040000990201593e-14;
t2035 = t18.*t1630;
t2043 = t8.*t24.*t199.*6.371903244127231e-7;
t2045 = t23.*t1630;
t2049 = t9.*t202.*8.040000990201593e-14;
t2050 = t18.*t1642;
t2075 = t5.*t7.*t200.*7.492102979241942e-7;
t2090 = -t1973;
t2123 = t8.*t9.*t199.*3.216000396080637e-13;
t2127 = -t2021;
t2134 = t8.*t19.*t199.*(-6.371903244127231e-7);
t2137 = -t2041;
t2138 = -t2044;
t2143 = -t2047;
t2146 = -t2055;
t2152 = -t2080;
t2160 = t8.*t201.*1.508157382287566e-7;
t2161 = t8.*t201.*3.016314764575132e-7;
t2164 = t7.*t200.*2.139166280618831e-6;
t2165 = t18.*t1759;
t2181 = t5.*t7.*t8.*t9.*t199.*2.143506553146841e-6;
t2193 = t5.*t7.*t199.*5.4093083807222e-13;
t2197 = -t2139;
t2198 = -t2141;
t2199 = -t2140;
t2202 = t7.*t8.*t19.*t199.*1.408936125616489e-6;
t2211 = t18.*t1822;
t2213 = t7.*t8.*t9.*t199.*7.492102979241942e-7;
t2215 = t18.*t1825;
t2216 = t22.*t1823;
t2222 = t18.*t1837;
t2224 = -t2150;
t2230 = -t2088;
t2238 = -t2162;
t2241 = -t2163;
t2247 = -t2167;
t2248 = -t2168;
t2253 = -t2177;
t2258 = -t2192;
t2259 = t9.*t200.*1.054342951111095e-13;
t2260 = t9.*t200.*2.10868590222219e-13;
t2261 = t9.*t201.*1.054342951111095e-13;
t2262 = t5.*t202.*1.054342951111095e-13;
t2263 = -t2195;
t2268 = -t2210;
t2288 = -t2250;
t2289 = t5.*t8.*t199.*4.217371804444381e-13;
t2290 = -t2252;
t2293 = t5.*t201.*4.300660646822946e-14;
t2296 = t9.*t201.*4.300660646822946e-14;
t2301 = t8.*t201.*5.773966567786041e-7;
t2303 = t7.*t8.*t199.*5.073437414621283e-7;
t2313 = t17.*t2147;
t2315 = t22.*t2147;
t2319 = -t2287;
t2320 = t7.*t9.*t199.*7.093613755211269e-13;
t2326 = t199.*t544;
t2327 = -t2292;
t2345 = -t2309;
t2346 = -t2314;
t2367 = -t2335;
t2383 = t199.*t572;
t2386 = -t2351;
t2393 = t17.*t2255;
t2398 = t22.*t2255;
t2404 = -t2368;
t2408 = -t2381;
t2416 = t199.*t595;
t2420 = -t2390;
t2424 = -t2395;
t2426 = -t2397;
t2448 = -t2423;
t2465 = t8.*t199.*7.452372645815517e-7;
t2479 = -t2471;
t2490 = -t2480;
t2494 = -t2482;
t2534 = -t2509;
t2542 = -t2524;
t2547 = -t2532;
t2594 = -t2580;
t2613 = t6.*t202.*5.463144604697158e-2;
t2614 = t9.*t2582;
t2620 = t2.*t199.*1.324388487819695e-2;
t2621 = t5.*t2585;
t2622 = t2.*t200.*1.324388487819695e-2;
t2623 = t2.*t201.*1.324388487819695e-2;
t2624 = t9.*t2585;
t2625 = t5.*t2586;
t2626 = t5.*t2587;
t2628 = t2.*t202.*1.324388487819695e-2;
t2629 = t6.*t201.*1.324388487819695e-2;
t2630 = t9.*t2586;
t2631 = t9.*t2587;
t2632 = t6.*t202.*1.324388487819695e-2;
t2642 = t5.*t2580;
t2643 = t2.*t201.*5.463144604697158e-2;
t2644 = t6.*t199.*5.463144604697158e-2;
t2645 = t9.*t2580;
t2646 = t5.*t2581;
t2647 = t2.*t202.*5.463144604697158e-2;
t2648 = t6.*t200.*5.463144604697158e-2;
t2649 = t6.*t201.*5.463144604697158e-2;
t2650 = t9.*t2581;
t2651 = t5.*t2582;
t2657 = t199.*8.76226105503051e-2;
t2658 = t5.*t2600;
t2660 = t200.*8.76226105503051e-2;
t2661 = t201.*8.76226105503051e-2;
t2662 = t9.*t2600;
t2663 = t5.*t2601;
t2664 = t202.*8.76226105503051e-2;
t2665 = t9.*t2601;
t2689 = t2.*t199.*3.46332667728404e-6;
t2729 = t2.*t5.*t200.*(-1.324388487819695e-2);
t2736 = -t2703;
t2737 = -t2702;
t2738 = t6.*t9.*t202.*(-1.324388487819695e-2);
t2740 = t199.*1.182954431201322e-5;
t2745 = t5.*t200.*4.081996247155408e-7;
t2746 = t2.*t5.*t202.*(-5.463144604697158e-2);
t2747 = t5.*t6.*t200.*(-5.463144604697158e-2);
t2750 = t6.*t199.*1.428633261714363e-5;
t2753 = t2.*t9.*t200.*1.73166333864202e-6;
t2754 = t2.*t9.*t200.*3.46332667728404e-6;
t2755 = t2.*t5.*t202.*1.73166333864202e-6;
t2756 = t2.*t5.*t202.*3.46332667728404e-6;
t2757 = t5.*t6.*t200.*1.73166333864202e-6;
t2758 = t5.*t6.*t200.*3.46332667728404e-6;
t2763 = t5.*t200.*(-8.76226105503051e-2);
t2765 = -t2733;
t2766 = -t2734;
t2767 = -t2739;
t2772 = t199.*6.433028743309294e-4;
t2778 = t2.*t5.*t199.*1.73166333864202e-6;
t2780 = t2.*t199.*1.882396747564322e-6;
t2785 = t6.*t199.*7.764946411068142e-6;
t2790 = t9.*t200.*2.218657717048192e-7;
t2793 = t5.*t199.*5.914772156006612e-6;
t2795 = t200.*6.003953432070899e-6;
t2796 = t200.*1.20079068641418e-5;
t2797 = t200.*4.200697734379648e-9;
t2798 = t200.*8.401395468759295e-9;
t2799 = -t2768;
t2800 = t9.*t200.*5.914772156006612e-6;
t2801 = t9.*t200.*1.182954431201322e-5;
t2802 = t5.*t202.*5.914772156006612e-6;
t2803 = t5.*t202.*1.182954431201322e-5;
t2805 = -t2773;
t2807 = t199.*6.429626140715183e-6;
t2809 = -t2776;
t2810 = t2.*t5.*t200.*7.143166308571814e-6;
t2811 = t2.*t5.*t200.*1.428633261714363e-5;
t2812 = t5.*t6.*t199.*7.143166308571814e-6;
t2814 = t199.*5.475413853010983e-6;
t2816 = t6.*t9.*t200.*7.143166308571814e-6;
t2817 = t6.*t9.*t200.*1.428633261714363e-5;
t2818 = t5.*t6.*t202.*7.143166308571814e-6;
t2819 = t5.*t6.*t202.*1.428633261714363e-5;
t2822 = t2.*t5.*t199.*(-3.46332667728404e-6);
t2823 = -t2782;
t2824 = -t2781;
t2825 = t2.*t9.*t202.*9.41198373782161e-7;
t2826 = t2.*t9.*t202.*1.882396747564322e-6;
t2827 = t6.*t9.*t200.*9.41198373782161e-7;
t2828 = t6.*t9.*t200.*1.882396747564322e-6;
t2832 = -t2787;
t2833 = -t2786;
t2834 = -t2789;
t2835 = -t2788;
t2837 = t7.*t199.*7.725649335384969e-9;
t2838 = t7.*t199.*1.545129867076994e-8;
t2839 = t5.*t199.*(-1.182954431201322e-5);
t2841 = t5.*t200.*6.433028743309294e-4;
t2843 = t9.*t200.*6.433028743309294e-4;
t2846 = -t2808;
t2852 = t5.*t6.*t199.*(-1.428633261714363e-5);
t2857 = t2.*t9.*t199.*9.41198373782161e-7;
t2859 = t2.*t5.*t200.*9.41198373782161e-7;
t2860 = t2.*t5.*t200.*1.882396747564322e-6;
t2865 = t200.*3.221288775573066e-7;
t2867 = -t2821;
t2870 = t2.*t9.*t200.*3.882473205534071e-6;
t2871 = t2.*t9.*t200.*7.764946411068142e-6;
t2872 = t6.*t9.*t199.*3.882473205534071e-6;
t2874 = t5.*t6.*t200.*3.882473205534071e-6;
t2875 = t5.*t6.*t200.*7.764946411068142e-6;
t2876 = t2.*t199.*2.733068497907686e-6;
t2877 = t6.*t9.*t202.*3.882473205534071e-6;
t2878 = t6.*t9.*t202.*7.764946411068142e-6;
t2882 = t2.*t202.*2.733068497907686e-6;
t2883 = t6.*t200.*2.733068497907686e-6;
t2885 = -t2840;
t2891 = t5.*t200.*6.429626140715183e-6;
t2893 = -t2847;
t2894 = t9.*t202.*6.429626140715183e-6;
t2895 = -t2848;
t2896 = -t2849;
t2897 = -t2853;
t2904 = t2.*t9.*t199.*(-1.882396747564322e-6);
t2907 = -t2862;
t2910 = -t2866;
t2911 = -t2868;
t2914 = t6.*t9.*t199.*(-7.764946411068142e-6);
t2918 = t2.*t199.*1.366534248953843e-6;
t2919 = -t2879;
t2921 = t2.*t202.*1.366534248953843e-6;
t2922 = t6.*t200.*1.366534248953843e-6;
t2931 = t9.*t199.*(-6.429626140715183e-6);
t2932 = t9.*t199.*3.214813070357591e-6;
t2934 = t5.*t200.*3.214813070357591e-6;
t2941 = t9.*t202.*3.214813070357591e-6;
t2942 = -t2898;
t2944 = -t2899;
t2946 = -t2901;
t2947 = -t2902;
t2954 = t2.*t200.*5.636997208875202e-6;
t2955 = t2.*t200.*1.12739944177504e-5;
t2956 = t6.*t199.*5.636997208875202e-6;
t2957 = t6.*t199.*1.12739944177504e-5;
t2958 = t6.*t202.*5.636997208875202e-6;
t2959 = t6.*t202.*1.12739944177504e-5;
t2965 = t202.*7.405322476003771e-6;
t2972 = -t2926;
t2973 = t199.*4.66761554949828e-6;
t2974 = t199.*9.33523109899656e-6;
t2977 = t202.*4.66761554949828e-6;
t2978 = t202.*9.33523109899656e-6;
t2994 = -t2943;
t2995 = -t2948;
t3001 = -t2960;
t3002 = -t2961;
t3005 = -t2963;
t3008 = -t2964;
t3009 = t8.*t2926;
t3018 = -t2976;
t3022 = -t2982;
t3037 = t18.*t2898;
t3040 = t8.*t17.*t2820;
t3041 = t8.*t2962;
t3042 = t8.*t2963;
t3044 = t8.*t22.*t2820;
t3048 = -t3003;
t3049 = -t3004;
t3050 = t8.*t2968;
t3054 = t8.*t2975;
t3059 = t3.*t4.*t7.*t2820;
t3064 = -t3023;
t3067 = -t3027;
t3068 = -t3028;
t3074 = -t3038;
t3076 = -t3039;
t3081 = -t3045;
t3084 = t8.*t3024;
t3086 = -t3062;
t3088 = -t3063;
t3089 = t18.*t2926;
t3096 = -t3075;
t3097 = -t3078;
t3100 = t17.*t18.*t2820;
t3101 = t17.*t18.*t2821;
t3102 = t2.*t5.*t200.*3.634948345122482e-13;
t3106 = t17.*t18.*t2784;
t3107 = t2.*t9.*t200.*3.634948345122482e-13;
t3110 = -t3087;
t3114 = -t3091;
t3117 = -t3093;
t3118 = -t3094;
t3121 = -t3099;
t3122 = t18.*t3004;
t3128 = -t3105;
t3134 = t2151./8.112963841460668e+31;
t3135 = t5.*t6.*t200.*1.499427745155113e-12;
t3136 = t2088./8.112963841460668e+31;
t3137 = t18.*t3024;
t3138 = t6.*t9.*t200.*1.499427745155113e-12;
t3141 = t5.*t200.*1.241574547458694e-12;
t3144 = t9.*t200.*1.241574547458694e-12;
t3153 = -t3123;
t3154 = -t3130;
t3169 = -t3145;
t3175 = -t3151;
t3176 = -t3152;
t3179 = t8.*t3132;
t3185 = -t3165;
t3188 = -t3173;
t3189 = t199.*4.143543013549434e-7;
t3192 = -t3177;
t3193 = -t3178;
t3195 = t8.*t3160;
t3196 = -t3186;
t3198 = -t3190;
t3200 = t2.*t200.*1.7577726911557e-6;
t3201 = t2.*t200.*3.5155453823114e-6;
t3202 = t2.*t201.*1.7577726911557e-6;
t3203 = t2.*t201.*3.5155453823114e-6;
t3204 = t6.*t199.*1.7577726911557e-6;
t3205 = t6.*t199.*3.5155453823114e-6;
t3209 = t2.*t199.*7.250868217512499e-6;
t3210 = t2.*t199.*1.4501736435025e-5;
t3213 = t6.*t200.*7.250868217512499e-6;
t3214 = t6.*t200.*1.4501736435025e-5;
t3215 = t6.*t201.*7.250868217512499e-6;
t3216 = t6.*t201.*1.4501736435025e-5;
t3217 = -t3197;
t3226 = t200.*1.200790562256725e-5;
t3227 = t201.*1.200790562256725e-5;
t3229 = -t3206;
t3232 = -t3207;
t3233 = t8.*t3197;
t3235 = t201.*1.200790624335452e-5;
t3247 = t200.*6.003952811283625e-6;
t3249 = t201.*6.003952811283625e-6;
t3267 = -t3241;
t3269 = -t3250;
t3270 = -t3253;
t3271 = -t3254;
t3322 = -t3291;
t3323 = -t3292;
t3332 = t5.*t3277;
t3336 = t9.*t3277;
t3337 = t8.*t3278;
t3340 = t9.*t3280;
t3341 = t5.*t3260;
t3344 = t9.*t3260;
t3349 = t5.*t3296;
t3351 = t9.*t3296;
t3352 = t8.*t3298;
t3353 = t9.*t3299;
t3354 = t8.*t3303;
t3355 = t9.*t3304;
t3356 = t5.*t3307;
t3357 = t9.*t3307;
t3358 = t8.*t3308;
t3359 = t9.*t3310;
t3360 = t8.*t3313;
t3361 = t9.*t3315;
t3385 = t4.*t3339;
t3386 = t8.*t3338;
t3388 = t8.*t3339;
t3428 = t18.*t3339;
t3429 = t23.*t3339;
t3448 = t8.*t3387;
t3460 = -t3423;
t3461 = -t3427;
t3478 = t8.*t3406;
t3482 = t4.*t3412;
t3484 = t8.*t3412;
t3526 = t8.*t3480;
t3537 = t18.*t3412;
t3540 = t23.*t3412;
t3561 = t2.*t201.*1.769880715106441e-6;
t3565 = t2.*t202.*1.769880715106441e-6;
t3566 = t6.*t201.*1.769880715106441e-6;
t3570 = -t3545;
t3588 = t2.*t199.*1.769880715106441e-6;
t3594 = t5.*t200.*2.086042441322004e-7;
t3595 = t5.*t201.*2.086042441322004e-7;
t3598 = -t3567;
t3600 = t9.*t202.*2.086042441322004e-7;
t3623 = t2.*t201.*7.30081420113316e-6;
t3624 = t6.*t199.*7.30081420113316e-6;
t3626 = t6.*t9.*t202.*1.769880715106441e-6;
t3632 = t6.*t201.*7.30081420113316e-6;
t3640 = t6.*t202.*7.30081420113316e-6;
t3664 = -t3608;
t3669 = -t3614;
t3670 = -t3615;
t3671 = t2.*t9.*t200.*1.769880715106441e-6;
t3674 = t5.*t6.*t200.*1.769880715106441e-6;
t3677 = -t3620;
t3678 = -t3619;
t3679 = t2.*t9.*t202.*(-1.769880715106441e-6);
t3685 = t6.*t9.*t202.*8.849403575532204e-7;
t3692 = t199.*6.367841787827598e-4;
t3698 = t201.*6.367841787827598e-4;
t3703 = t202.*6.367841787827598e-4;
t3711 = t25.*t3527;
t3712 = t25.*t3528;
t3718 = t26.*t3527;
t3719 = t26.*t3528;
t3727 = t199.*1.170967356229242e-5;
t3731 = t201.*1.170967356229242e-5;
t3739 = t9.*t200.*1.133811468776912e-7;
t3740 = t9.*t201.*1.133811468776912e-7;
t3741 = t5.*t202.*1.133811468776912e-7;
t3742 = t202.*1.170967356229242e-5;
t3753 = t2.*t9.*t200.*8.849403575532204e-7;
t3754 = t2.*t9.*t201.*(-1.769880715106441e-6);
t3755 = t2.*t9.*t201.*8.849403575532204e-7;
t3759 = t2.*t9.*t202.*3.65040710056658e-6;
t3760 = t2.*t9.*t202.*7.30081420113316e-6;
t3761 = t6.*t9.*t200.*3.65040710056658e-6;
t3762 = t6.*t9.*t200.*7.30081420113316e-6;
t3763 = t6.*t9.*t201.*3.65040710056658e-6;
t3772 = -t3688;
t3775 = t2.*t199.*9.619703863182361e-7;
t3777 = -t3693;
t3779 = t2.*t201.*9.619703863182361e-7;
t3781 = t2.*t202.*9.619703863182361e-7;
t3782 = t6.*t201.*9.619703863182361e-7;
t3788 = t25.*t3550;
t3790 = t199.*5.419930569269819e-6;
t3791 = t26.*t3550;
t3793 = t201.*5.419930569269819e-6;
t3794 = -t3721;
t3796 = -t3723;
t3797 = t202.*5.419930569269819e-6;
t3801 = t2.*t201.*3.96815841743287e-6;
t3802 = t6.*t199.*3.96815841743287e-6;
t3812 = t6.*t201.*3.96815841743287e-6;
t3818 = t6.*t202.*3.96815841743287e-6;
t3828 = t2.*t5.*t200.*7.30081420113316e-6;
t3833 = t6.*t9.*t201.*(-7.30081420113316e-6);
t3836 = t6.*t9.*t202.*(-7.30081420113316e-6);
t3837 = t5.*t200.*6.367841787827598e-4;
t3840 = t9.*t200.*6.367841787827598e-4;
t3845 = -t3776;
t3854 = t8.*t3721;
t3856 = t199.*6.364473664374288e-6;
t3860 = t200.*1.646190906295504e-7;
t3861 = t201.*1.646190906295504e-7;
t3862 = t8.*t3724;
t3863 = t5.*t199.*5.85483678114621e-6;
t3865 = t201.*6.364473664374288e-6;
t3868 = t202.*6.364473664374288e-6;
t3871 = t9.*t200.*5.85483678114621e-6;
t3872 = t9.*t200.*1.170967356229242e-5;
t3873 = t9.*t201.*5.85483678114621e-6;
t3875 = t5.*t202.*5.85483678114621e-6;
t3881 = -t3804;
t3882 = -t3803;
t3883 = -t3805;
t3884 = -t3806;
t3886 = t200.*1.18862287368685e-5;
t3887 = t201.*1.18862287368685e-5;
t3888 = -t3817;
t3893 = t202.*1.18862287368685e-5;
t3894 = -t3826;
t3895 = -t3827;
t3897 = t2.*t5.*t201.*(-7.30081420113316e-6);
t3901 = t2.*t5.*t200.*4.809851931591181e-7;
t3902 = t2.*t5.*t200.*9.619703863182361e-7;
t3903 = t2.*t5.*t201.*4.809851931591181e-7;
t3908 = t6.*t9.*t200.*9.619703863182361e-7;
t3910 = t5.*t6.*t202.*4.809851931591181e-7;
t3911 = t5.*t6.*t202.*9.619703863182361e-7;
t3914 = t9.*t202.*(-6.367841787827598e-4);
t3916 = t2.*t199.*1.396693317797299e-6;
t3918 = -t3855;
t3921 = -t3858;
t3922 = -t3857;
C_dq = ft_10({dq1,dq2,dq3,dq4,dq5,dq6,t1004,t1006,t1008,t101,t1013,t1016,t1017,t1019,t102,t1020,t1021,t1023,t1024,t1025,t1026,t1028,t1030,t1032,t1034,t1036,t1038,t1039,t1040,t1042,t1043,t1044,t1045,t1046,t1047,t1048,t1049,t1050,t1051,t1054,t1055,t1056,t1057,t1059,t1061,t1065,t1066,t1068,t1069,t1070,t1072,t1073,t1075,t1076,t1077,t1081,t1083,t1084,t1085,t1087,t1089,t1091,t1092,t1093,t1095,t1098,t1099,t110,t1101,t1102,t1105,t1106,t1107,t1108,t1109,t111,t1113,t1115,t1116,t1119,t112,t1122,t1125,t1126,t1127,t1128,t113,t1130,t1131,t1133,t1134,t1135,t1138,t1139,t114,t1141,t1144,t1145,t1146,t1147,t1148,t1149,t115,t1150,t1152,t1153,t1155,t1158,t1159,t116,t1162,t1163,t1165,t1167,t1169,t1170,t1171,t1173,t1174,t1175,t1177,t1178,t1179,t1180,t1181,t1182,t1183,t1184,t1185,t1186,t1188,t1189,t1190,t1191,t1192,t1193,t1194,t1196,t1197,t1198,t1199,t120,t1200,t1202,t1203,t1204,t1205,t1206,t1207,t121,t1210,t1211,t1215,t1219,t1221,t1222,t1224,t1225,t1227,t1228,t1233,t1235,t1236,t1237,t1239,t124,t1240,t1241,t1244,t1245,t125,t1250,t1251,t1253,t1254,t1256,t1257,t1258,t1259,t126,t1261,t1262,t1263,t1264,t1265,t1266,t1267,t1268,t1269,t1271,t1272,t1273,t1274,t1277,t1278,t128,t1280,t1282,t1285,t1286,t1288,t129,t1290,t1293,t1294,t1295,t1296,t1298,t1300,t1301,t1302,t1306,t1307,t1308,t1309,t131,t1311,t1312,t1313,t1315,t1316,t1317,t1318,t1319,t132,t1322,t1323,t1324,t1325,t1326,t1328,t1329,t133,t1330,t1331,t1333,t1334,t1337,t1338,t1340,t1341,t1342,t1343,t1344,t1345,t1346,t1348,t1351,t1352,t1353,t1354,t1355,t1356,t1360,t1362,t1365,t1366,t1367,t1369,t1370,t1371,t1372,t1374,t1375,t1377,t1378,t1379,t1380,t1383,t1384,t1385,t1386,t1388,t1389,t139,t1391,t1392,t1393,t1394,t1397,t1398,t140,t1401,t1402,t1403,t1404,t1406,t1407,t1408,t1409,t141,t1410,t1411,t1413,t1414,t1415,t1416,t1417,t1419,t142,t1422,t1423,t1426,t1427,t1428,t1429,t1430,t1431,t1432,t1433,t1436,t144,t1440,t1441,t1442,t1443,t1445,t1446,t1447,t1448,t1449,t1451,t1452,t1453,t1454,t1455,t1456,t1457,t1458,t1459,t1460,t1463,t1464,t1465,t1467,t1470,t1471,t1474,t1476,t1478,t1479,t148,t1480,t1481,t1482,t1483,t1486,t1487,t1488,t1489,t1490,t1491,t1492,t1493,t1494,t1495,t1496,t1498,t1499,t15,t150,t1500,t1501,t1503,t1505,t1506,t1507,t1508,t1509,t151,t1510,t1511,t1512,t1513,t1515,t1517,t1520,t1521,t1522,t1523,t1524,t1526,t1527,t1529,t153,t1530,t1531,t1532,t1533,t1534,t1535,t1536,t1537,t1538,t1539,t154,t1540,t1541,t1542,t1548,t1549,t1550,t1551,t1553,t1558,t156,t1560,t1561,t1562,t1564,t1566,t1567,t1568,t157,t1570,t1571,t1572,t1574,t1575,t1576,t1577,t1578,t1579,t158,t1580,t1581,t1582,t1583,t1584,t1585,t1586,t1587,t1589,t1590,t1591,t1592,t1593,t1594,t1595,t1596,t1597,t1598,t1599,t16,t1601,t1602,t1605,t1606,t1607,t1609,t161,t1610,t1611,t1612,t1613,t1614,t1615,t1616,t1617,t1618,t1619,t1620,t1621,t1622,t1625,t1626,t1627,t163,t1630,t1631,t1632,t1633,t1635,t1636,t1637,t1638,t1639,t1641,t1642,t1643,t1644,t1645,t1646,t1647,t1648,t165,t1651,t1652,t1653,t1657,t1658,t1659,t166,t1660,t1661,t1662,t1663,t1666,t1667,t1669,t1670,t1671,t1672,t1673,t1674,t1675,t1676,t1681,t1682,t1683,t1686,t1687,t1689,t1691,t1692,t1696,t1697,t1698,t1699,t17,t170,t1700,t1701,t1702,t1703,t1704,t1705,t1706,t1709,t171,t1710,t1711,t1712,t1713,t1715,t1716,t1718,t1719,t1720,t1721,t1722,t1723,t1724,t1726,t1728,t1729,t1731,t1733,t1734,t1735,t1736,t1737,t1738,t1739,t1740,t1741,t1745,t1746,t1747,t1748,t1749,t1752,t1753,t1754,t1755,t1756,t1757,t1758,t1759,t1760,t1761,t1763,t1764,t1765,t1766,t1767,t1768,t1769,t177,t1770,t1771,t1772,t1774,t1775,t1776,t1777,t1779,t1780,t1781,t1783,t1784,t1785,t1786,t1787,t1788,t1789,t1790,t1791,t1792,t1793,t1794,t1795,t1797,t1798,t1799,t18,t1800,t1801,t1804,t1805,t1806,t1807,t1808,t1809,t1810,t1811,t1812,t1813,t1814,t1815,t1816,t1817,t1820,t1822,t1823,t1824,t1827,t1828,t1829,t183,t1830,t1831,t1832,t1833,t1834,t1835,t1836,t1837,t1838,t1839,t1844,t1845,t1846,t1847,t1848,t1849,t185,t1850,t1851,t1853,t1855,t1856,t1857,t1858,t1859,t1861,t1864,t1865,t1866,t1867,t1871,t1873,t1877,t1879,t1881,t1882,t1884,t1885,t1886,t1887,t1889,t1891,t1892,t1893,t1896,t19,t190,t1900,t1902,t1903,t1905,t1906,t1907,t1908,t1909,t191,t1910,t1911,t1912,t1913,t1914,t1915,t1916,t1917,t1918,t1919,t1920,t1921,t1925,t1926,t1927,t1928,t1930,t1934,t1935,t1936,t1937,t1938,t1939,t1942,t1943,t1944,t1946,t1947,t1950,t1951,t1952,t1953,t1954,t1955,t196,t1961,t1966,t1967,t1968,t1969,t197,t1970,t1971,t1975,t1976,t1977,t1978,t1979,t1980,t1981,t1983,t1984,t1985,t1986,t1987,t1988,t1989,t199,t1991,t1992,t1993,t1994,t1995,t1996,t1997,t1998,t1999,t2,t20,t200,t2000,t2001,t2002,t2003,t2004,t2005,t2006,t2008,t201,t2011,t2014,t2015,t2016,t2017,t2018,t2019,t202,t2020,t2023,t2024,t2026,t2027,t2028,t2029,t203,t2033,t2035,t2036,t2037,t2038,t204,t2040,t2042,t2043,t2045,t2047,t2049,t205,t2050,t2051,t2052,t2053,t2054,t2056,t2057,t2058,t2059,t206,t2060,t2061,t2062,t2065,t2066,t2067,t2068,t2069,t207,t2070,t2071,t2072,t2073,t2074,t2075,t2076,t2077,t2078,t2079,t208,t2081,t2082,t2083,t2084,t2085,t2086,t2087,t2088,t2089,t209,t2090,t2091,t2092,t2093,t2094,t2095,t2096,t2097,t2098,t2099,t21,t210,t2100,t2101,t2104,t2105,t2106,t2107,t2108,t2109,t211,t2110,t2111,t2113,t2114,t2115,t2116,t2117,t2118,t2119,t212,t2121,t2123,t2125,t2127,t2128,t2129,t213,t2130,t2131,t2132,t2133,t2134,t2135,t2136,t2137,t2138,t2142,t2143,t2144,t2146,t2148,t2149,t2150,t2151,t2152,t2154,t2155,t2156,t2157,t2158,t2159,t2160,t2161,t2164,t2165,t2166,t2169,t2170,t2171,t2172,t2174,t2175,t2176,t2177,t2178,t2180,t2181,t2182,t2184,t2185,t2186,t2187,t2189,t2190,t2191,t2192,t2193,t2194,t2196,t2197,t2198,t2199,t22,t2200,t2201,t2202,t2203,t2204,t2208,t2209,t2211,t2212,t2213,t2214,t2215,t2216,t2217,t2218,t2219,t2220,t2221,t2223,t2224,t2225,t2227,t2228,t2229,t2230,t2231,t2232,t2236,t2237,t2238,t2239,t224,t2240,t2241,t2243,t2246,t2247,t2248,t2249,t225,t2251,t2253,t2254,t2256,t2257,t2258,t2259,t2260,t2261,t2262,t2263,t2264,t2265,t2266,t2267,t2268,t2269,t227,t2270,t2271,t2272,t2273,t2274,t2276,t2277,t2278,t2279,t228,t2280,t2281,t2282,t2283,t2284,t2285,t2286,t2288,t2289,t2290,t2291,t2293,t2295,t2296,t23,t230,t2301,t2302,t2303,t2304,t2305,t2306,t2307,t2308,t231,t2310,t2311,t2312,t2313,t2314,t2315,t2316,t2317,t2318,t2319,t2320,t2321,t2322,t2323,t2324,t2326,t2327,t233,t2331,t2333,t2334,t2336,t2337,t2338,t2339,t234,t2340,t2341,t2342,t2344,t2345,t2346,t2347,t2348,t235,t2350,t2355,t2357,t2358,t2359,t236,t2361,t2362,t2363,t2364,t2365,t2366,t2367,t2369,t2370,t2371,t2372,t2373,t2374,t2375,t2376,t2377,t2378,t2379,t2382,t2383,t2384,t2385,t2386,t2387,t2388,t2389,t2390,t2391,t2392,t2393,t2394,t2395,t2396,t2397,t2398,t24,t240,t2400,t2401,t2402,t2403,t2404,t2405,t2406,t2407,t2408,t2410,t2416,t2417,t2420,t2421,t2422,t2424,t2425,t2426,t2427,t2428,t2429,t243,t2430,t2431,t2434,t2435,t2437,t2438,t2439,t244,t2440,t2441,t2443,t2444,t2445,t2446,t2448,t2449,t2452,t2453,t2454,t2455,t2456,t2457,t2458,t2459,t2460,t2461,t2463,t2464,t2465,t2466,t2467,t2469,t2470,t2472,t2474,t2477,t2478,t2479,t2481,t2483,t2484,t2485,t2486,t2487,t2489,t249,t2490,t2494,t2495,t2497,t2500,t2502,t2503,t2505,t2507,t2508,t2510,t2511,t2512,t2513,t2517,t2518,t2519,t2520,t2521,t2522,t2523,t2524,t2525,t2526,t2527,t2530,t2531,t2533,t2534,t2535,t2536,t2537,t2539,t2540,t2541,t2542,t2543,t2544,t2545,t2546,t2547,t2548,t2549,t2550,t2552,t2553,t2554,t2555,t2556,t2560,t2562,t2563,t2564,t2565,t2566,t2567,t2568,t2569,t257,t2570,t2571,t2574,t2575,t2576,t2577,t2578,t2579,t258,t2581,t2582,t2585,t2586,t2587,t2588,t2589,t2590,t2594,t2595,t2597,t2598,t2599,t2600,t2601,t2602,t2603,t2604,t2606,t2607,t2608,t2611,t2612,t2613,t2614,t2615,t2616,t2617,t2620,t2622,t2623,t2624,t2625,t2626,t2627,t2628,t2629,t263,t2630,t2631,t2632,t2633,t2634,t2636,t2639,t2640,t2641,t2643,t2644,t2647,t2648,t2649,t2650,t2651,t2654,t2655,t2656,t2657,t2659,t266,t2660,t2661,t2662,t2663,t2664,t2665,t2666,t2668,t2669,t2671,t2673,t2675,t2676,t2677,t2678,t2680,t2681,t2682,t2684,t2685,t2686,t2688,t2689,t2692,t2693,t2694,t2695,t2699,t270,t2705,t2706,t2707,t2708,t2719,t2720,t2721,t2722,t2723,t2724,t2725,t2726,t2729,t273,t2736,t2737,t2738,t274,t2740,t2741,t2742,t2743,t2744,t2745,t2746,t2747,t2748,t2749,t275,t2750,t2752,t2753,t2754,t2755,t2756,t2757,t2758,t2759,t276,t2760,t2761,t2762,t2763,t2764,t2765,t2766,t2767,t2769,t277,t2770,t2771,t2772,t2774,t2775,t2778,t278,t2780,t2783,t2784,t2785,t2790,t2791,t2792,t2793,t2795,t2796,t2797,t2798,t2799,t280,t2800,t2801,t2802,t2803,t2805,t2806,t2807,t2809,t2810,t2811,t2812,t2814,t2815,t2816,t2817,t2818,t2819,t2820,t2822,t2823,t2824,t2825,t2826,t2827,t2828,t2829,t2830,t2831,t2832,t2833,t2834,t2835,t2837,t2838,t2839,t284,t2841,t2842,t2843,t2844,t2845,t2846,t2852,t2854,t2857,t2859,t2860,t2861,t2863,t2864,t2865,t2867,t2868,t2869,t287,t2870,t2871,t2872,t2874,t2875,t2876,t2877,t2878,t2882,t2883,t2884,t2885,t2886,t2888,t2891,t2892,t2893,t2894,t2895,t2896,t2897,t29,t290,t2900,t2903,t2904,t2907,t2908,t291,t2910,t2911,t2914,t2918,t2919,t292,t2920,t2921,t2922,t2923,t2925,t2928,t2929,t2930,t2931,t2932,t2934,t2937,t294,t2940,t2941,t2942,t2944,t2945,t2946,t2947,t2949,t2950,t2951,t2952,t2954,t2955,t2956,t2957,t2958,t2959,t2962,t2965,t2966,t2967,t2968,t2969,t297,t2970,t2971,t2972,t2973,t2974,t2975,t2977,t2978,t2980,t2983,t2984,t2985,t2986,t2988,t2989,t299,t2991,t2992,t2993,t2994,t2995,t2996,t2997,t3,t30,t300,t3001,t3002,t3003,t3005,t3007,t3008,t3010,t3011,t3013,t3014,t3018,t3019,t302,t3020,t3021,t3022,t3024,t3025,t3027,t3029,t303,t3030,t3031,t3032,t3033,t3034,t3035,t3036,t3037,t3038,t304,t3041,t3043,t3044,t3046,t3047,t3048,t3049,t305,t3050,t3051,t3052,t3053,t3054,t3055,t3056,t3057,t3059,t306,t3060,t3061,t3062,t3064,t3065,t3066,t3067,t3068,t3069,t3070,t3071,t3072,t3073,t3074,t3076,t3077,t3079,t3080,t3081,t3082,t3083,t3084,t3085,t3086,t3088,t3089,t309,t3090,t3092,t3094,t3095,t3096,t3097,t3098,t3099,t310,t3100,t3102,t3103,t3104,t3105,t3106,t3107,t3108,t3109,t311,t3110,t3112,t3113,t3114,t3117,t3118,t3119,t3120,t3121,t3122,t3123,t3124,t3126,t3127,t3128,t313,t3130,t3131,t3132,t3133,t3134,t3135,t3136,t3138,t3139,t314,t3140,t3141,t3142,t3143,t3144,t3146,t3148,t3149,t315,t3150,t3152,t3153,t3154,t3156,t3157,t3158,t316,t3160,t3163,t3167,t3169,t3170,t3171,t3172,t3174,t3175,t3176,t3178,t3179,t318,t3180,t3182,t3183,t3184,t3185,t3186,t3187,t3188,t3189,t319,t3190,t3191,t3192,t3193,t3194,t3195,t3196,t3198,t3199,t320,t3200,t3201,t3202,t3203,t3204,t3205,t3207,t3208,t3209,t3210,t3213,t3214,t3215,t3216,t3217,t3219,t322,t3226,t3227,t3228,t3229,t3230,t3232,t3234,t3235,t3236,t324,t3240,t3242,t3243,t3245,t3247,t3249,t325,t3250,t3251,t3252,t3254,t3256,t3257,t3265,t3267,t3269,t3270,t3271,t3272,t3273,t3274,t3275,t3276,t3277,t3278,t3279,t328,t3280,t3282,t3283,t3284,t3285,t3286,t3287,t3288,t3289,t3290,t3291,t3292,t3293,t3295,t3296,t3297,t3298,t3299,t3301,t3302,t3303,t3306,t3307,t3308,t3309,t3310,t3312,t3313,t3314,t3317,t3318,t3320,t3321,t3322,t3323,t3324,t3325,t3326,t3327,t3328,t3329,t333,t3331,t3332,t3333,t3334,t3335,t3336,t3337,t3338,t3339,t3340,t3341,t3342,t3343,t3346,t3347,t3349,t3350,t3351,t3352,t3353,t3354,t3356,t3357,t3358,t3359,t336,t3360,t3362,t3363,t3364,t3365,t3366,t3367,t3368,t3369,t337,t3371,t3372,t3373,t3374,t3375,t3376,t3377,t3378,t3380,t3381,t3382,t3383,t3384,t3386,t3387,t3388,t3390,t3391,t3392,t3393,t3394,t3395,t3396,t3397,t3398,t3399,t34,t340,t3400,t3402,t3403,t3404,t3405,t3407,t3408,t3409,t3410,t3411,t3412,t3413,t3416,t3417,t3418,t3420,t3421,t3422,t3423,t3424,t3425,t3426,t3427,t3429,t3430,t3431,t3432,t3433,t3434,t3435,t3436,t3437,t3439,t344,t3440,t3441,t3442,t3443,t3444,t3445,t3446,t3447,t3448,t3449,t3450,t3453,t3454,t3455,t3456,t3457,t3458,t346,t3460,t3461,t3462,t3463,t3464,t3465,t3466,t3467,t3468,t3469,t347,t3470,t3471,t3472,t3473,t3474,t3475,t3476,t3479,t348,t3480,t3481,t3483,t3484,t3485,t3487,t3488,t3489,t349,t3490,t3491,t3492,t3493,t3494,t3496,t3497,t3498,t3499,t350,t3500,t3501,t3502,t3503,t3504,t3505,t3506,t3507,t3509,t3510,t3511,t3513,t3514,t3515,t3516,t3517,t3518,t352,t3521,t3522,t3523,t3526,t3529,t353,t3530,t3531,t3532,t3533,t3535,t3536,t3538,t3539,t3540,t3542,t3543,t3544,t3546,t3547,t3549,t3551,t3552,t3554,t3556,t3557,t3559,t356,t3560,t3561,t3562,t3563,t3564,t3565,t3566,t3568,t3569,t357,t3570,t3571,t3572,t3573,t3574,t3577,t3578,t358,t3582,t3583,t3584,t3585,t3586,t3587,t3588,t3589,t359,t3590,t3592,t3593,t3594,t3595,t3596,t3597,t3598,t3599,t3600,t3602,t3603,t3604,t3605,t3606,t3607,t3609,t361,t3610,t3611,t3612,t3616,t3617,t3618,t362,t3623,t3624,t3625,t3626,t3630,t3631,t3632,t3633,t3634,t3635,t3636,t3637,t3638,t3640,t3642,t3644,t3648,t365,t3652,t3653,t3654,t3655,t3656,t3657,t3658,t3659,t3660,t3662,t3663,t3664,t3666,t3667,t3668,t3669,t3670,t3671,t3674,t3676,t3677,t3678,t3679,t368,t3681,t3682,t3685,t3687,t369,t3690,t3691,t3692,t3693,t3694,t3695,t3696,t3697,t3698,t3699,t3700,t3701,t3702,t3703,t3704,t3705,t3706,t3707,t3708,t3709,t371,t3711,t3712,t3713,t3715,t3716,t3717,t3718,t3719,t372,t3720,t3724,t3725,t3726,t3727,t3728,t3729,t373,t3730,t3731,t3732,t3733,t3734,t3735,t3736,t3737,t3738,t3739,t374,t3740,t3741,t3742,t3743,t3744,t3745,t3746,t3747,t3750,t3752,t3753,t3754,t3755,t3756,t3757,t3758,t3759,t3760,t3761,t3762,t3763,t3766,t3768,t3769,t377,t3772,t3774,t3775,t3777,t3778,t3779,t378,t3780,t3781,t3782,t3783,t3784,t3785,t3786,t3787,t3788,t3789,t379,t3790,t3791,t3792,t3793,t3794,t3795,t3796,t3797,t3798,t380,t3800,t3801,t3802,t3810,t3811,t3812,t3813,t3814,t3815,t3816,t3817,t3818,t3819,t382,t3820,t3821,t3822,t3823,t3824,t3825,t3826,t3827,t3828,t3831,t3833,t3834,t3835,t3836,t3837,t3839,t384,t3840,t3843,t3845,t3849,t3850,t3851,t3852,t3853,t3855,t3856,t386,t3860,t3861,t3862,t3863,t3865,t3866,t3867,t3868,t3869,t387,t3870,t3871,t3872,t3873,t3875,t3877,t388,t3881,t3882,t3883,t3884,t3885,t3886,t3887,t3888,t3889,t3890,t3891,t3892,t3893,t3894,t3895,t3897,t3899,t3901,t3902,t3903,t3908,t391,t3910,t3911,t3912,t3913,t3914,t3915,t3916,t3917,t3918,t392,t3921,t3922,t3929,t3930,t3941,t3946,t3949,t395,t3950,t3951,t3952,t3953,t3958,t3959,t396,t3966,t3970,t3980,t3981,t3982,t3984,t3990,t4,t400,t4004,t4005,t4006,t401,t4010,t4011,t4014,t4015,t4016,t4017,t4018,t4019,t402,t4020,t4021,t4022,t4023,t4024,t4025,t4026,t4027,t4028,t4029,t403,t4036,t4039,t4040,t4041,t4042,t4045,t4046,t4047,t4048,t4051,t4053,t4054,t406,t4062,t4063,t4064,t4065,t4068,t4069,t4070,t4071,t4073,t4074,t4075,t4089,t4099,t410,t4103,t4105,t411,t4113,t4114,t4116,t4118,t4119,t412,t4123,t4124,t4125,t413,t4132,t414,t4140,t4142,t4143,t4144,t4145,t415,t4150,t4152,t4153,t416,t4162,t4164,t4165,t4166,t4169,t417,t4171,t4173,t4174,t4177,t4178,t4179,t418,t4180,t4181,t4183,t4184,t4185,t4186,t4188,t4190,t4195,t4196,t4197,t420,t4201,t4202,t4205,t4206,t4207,t4208,t4209,t4210,t4211,t4215,t4217,t4218,t4219,t422,t4220,t4221,t4223,t4224,t4225,t4226,t4228,t4229,t423,t4230,t4231,t4232,t4233,t4234,t4235,t424,t4241,t4242,t4243,t4244,t4245,t4246,t4247,t4248,t4249,t425,t4250,t4251,t4253,t4254,t4255,t4256,t4257,t4258,t4259,t4260,t4261,t4262,t4263,t427,t4273,t4274,t4275,t4276,t4278,t4279,t428,t4280,t4281,t4282,t4283,t4284,t4285,t4286,t4287,t4289,t429,t4290,t4291,t4292,t4293,t4295,t4296,t4297,t4298,t4299,t4300,t4301,t4302,t4303,t4304,t4305,t4306,t4308,t431,t4310,t4315,t4316,t4317,t4318,t432,t4321,t4323,t4324,t4325,t4326,t4327,t4328,t4329,t433,t4330,t4331,t4332,t4333,t4334,t4335,t4336,t4337,t4338,t4339,t434,t4340,t4342,t4344,t4345,t4346,t4347,t4348,t4349,t435,t4350,t4354,t4356,t4357,t436,t4362,t4363,t4365,t4366,t4368,t4369,t437,t4370,t4371,t4372,t4373,t4374,t4375,t4376,t4377,t4379,t438,t4380,t4382,t4383,t4384,t4385,t4386,t4387,t4388,t4389,t439,t4391,t4392,t4394,t4395,t4396,t4397,t4398,t4399,t44,t440,t4400,t4401,t4402,t4403,t4404,t4405,t4406,t4407,t4408,t4409,t441,t4410,t4411,t4412,t4413,t4414,t4415,t4416,t4417,t4418,t4419,t442,t4420,t4421,t4422,t4423,t4424,t4425,t4426,t4427,t4428,t4429,t4430,t4431,t4432,t4433,t4434,t4435,t4436,t4437,t4438,t4439,t444,t4440,t4442,t4444,t4445,t4446,t4447,t4448,t4449,t445,t4450,t4451,t4453,t4454,t4455,t4460,t4461,t4462,t4463,t4464,t4465,t4466,t4467,t4468,t4469,t4470,t4471,t4473,t4474,t4475,t4476,t4477,t4478,t4479,t448,t4481,t4482,t4483,t4484,t4485,t4486,t4487,t4488,t4489,t449,t4490,t4493,t4494,t4495,t4496,t4497,t4498,t4499,t45,t450,t4500,t4501,t4502,t4503,t4504,t4505,t4506,t4507,t4508,t4509,t4510,t4512,t4513,t4514,t4515,t4516,t4518,t4519,t452,t4520,t4521,t4522,t4523,t4524,t4525,t4526,t4527,t4529,t453,t4530,t4531,t4532,t4534,t4535,t4537,t4538,t4539,t454,t4541,t4543,t4544,t4545,t4546,t4547,t4549,t4550,t4551,t4552,t4553,t4554,t4556,t4557,t4558,t4559,t4560,t4564,t4565,t4566,t4567,t4568,t4569,t457,t4570,t4572,t4573,t4575,t4576,t4577,t4578,t458,t4580,t4581,t4582,t4584,t4586,t4587,t4588,t4589,t459,t4590,t4591,t4592,t4593,t4594,t4595,t4596,t4597,t4598,t4599,t46,t460,t4600,t4601,t4602,t4603,t4604,t4605,t4606,t4607,t4608,t4609,t461,t4610,t4612,t4613,t4614,t4615,t4616,t4617,t4618,t4619,t462,t4620,t4621,t4622,t4623,t4624,t4625,t4626,t4627,t4629,t463,t4631,t4632,t4633,t4634,t4635,t4636,t4637,t4638,t4639,t464,t4640,t4643,t4644,t4645,t4646,t4647,t4649,t465,t4650,t4652,t4653,t4654,t4655,t4656,t4657,t4659,t466,t4660,t4661,t4662,t4663,t4664,t4665,t4666,t4667,t4668,t4669,t4670,t4671,t4672,t4673,t4674,t4675,t4676,t4677,t4678,t4679,t468,t4680,t4681,t4682,t4683,t4684,t4685,t4686,t4687,t4689,t469,t4692,t4693,t4694,t4695,t4696,t4697,t4698,t4699,t47,t470,t4700,t4702,t4703,t4704,t4707,t4708,t4709,t471,t4710,t4711,t4712,t4713,t4714,t4715,t4716,t4717,t4718,t4719,t472,t4720,t4721,t4722,t4723,t4724,t4725,t4726,t4727,t4728,t4729,t4730,t4731,t4732,t4733,t4734,t4736,t4737,t4738,t4739,t4740,t4742,t4745,t4746,t4747,t4748,t475,t4750,t4751,t4753,t4754,t4755,t4756,t4757,t4762,t4763,t4765,t4768,t477,t4771,t4772,t4773,t4774,t4775,t4776,t4779,t4780,t4781,t4782,t4783,t4784,t4785,t4786,t4787,t4788,t4789,t479,t4790,t4791,t4792,t4793,t4794,t4795,t4797,t4799,t480,t4800,t4801,t4802,t4803,t4805,t4806,t4809,t481,t4810,t4811,t4812,t4813,t4814,t4818,t4819,t482,t4820,t4821,t4824,t4825,t4826,t4827,t4829,t483,t4831,t4833,t4834,t4835,t4837,t484,t4840,t4841,t4842,t4845,t4846,t4847,t4848,t485,t4851,t4853,t4856,t4857,t486,t4862,t4863,t4864,t4865,t4866,t4867,t4868,t4869,t4870,t4872,t4873,t4874,t4875,t4876,t4877,t488,t4880,t4884,t4888,t489,t4893,t4895,t4903,t4904,t4907,t4908,t491,t4911,t4913,t4914,t4919,t492,t4920,t4922,t4924,t4925,t4927,t4928,t4929,t493,t4931,t4933,t4934,t4935,t4936,t494,t4942,t4943,t4944,t4946,t4948,t4949,t4950,t4951,t4952,t4953,t4957,t496,t4963,t4964,t4969,t497,t4970,t4973,t4974,t4975,t4976,t4978,t4979,t498,t4981,t4982,t4983,t4987,t4988,t4989,t499,t4990,t4991,t4992,t4993,t4994,t4995,t4996,t5,t50,t500,t5000,t5001,t5002,t5003,t5005,t5006,t5007,t5008,t5009,t501,t5010,t5014,t5015,t5016,t5017,t5018,t5019,t502,t5020,t5021,t5022,t5023,t5024,t5026,t5027,t5029,t503,t5030,t5031,t5032,t5035,t5036,t5039,t504,t5041,t5045,t5048,t505,t5051,t5054,t5055,t5056,t5058,t5059,t506,t5061,t5063,t5064,t5065,t5066,t5067,t507,t5073,t5074,t5075,t5076,t5077,t5078,t508,t5080,t5081,t5083,t5084,t5085,t5088,t5089,t509,t5090,t5091,t5093,t5095,t5097,t5098,t5099,t510,t5100,t5101,t5102,t5107,t5109,t511,t5110,t5112,t5113,t5114,t5119,t512,t5120,t5121,t5123,t5125,t513,t5131,t5132,t5136,t5138,t5139,t514,t5140,t5143,t5146,t5147,t5148,t5150,t5151,t5152,t5153,t5154,t5157,t5158,t516,t5164,t5166,t517,t5171,t5172,t5174,t5175,t518,t5180,t5181,t5183,t5184,t5185,t5187,t5189,t5191,t5195,t5199,t520,t5200,t5201,t5202,t5203,t5204,t5205,t5206,t5207,t5209,t521,t5210,t5211,t5215,t5216,t5217,t5218,t5219,t522,t5222,t5223,t5224,t5227,t5229,t523,t5233,t5236,t5237,t5238,t5239,t524,t5240,t5242,t5244,t5247,t5248,t5249,t525,t5251,t5252,t5255,t5257,t5258,t526,t5261,t5262,t5265,t5268,t5269,t527,t5270,t5272,t5279,t528,t5280,t5285,t5288,t529,t5292,t5293,t5294,t5295,t5297,t53,t530,t5302,t5306,t531,t5318,t532,t5320,t5321,t5324,t5327,t533,t5331,t5332,t5339,t534,t5344,t5346,t5347,t5348,t5349,t535,t5351,t5355,t5356,t5358,t536,t5361,t5364,t5365,t5367,t5368,t537,t5372,t5373,t5375,t5378,t538,t5383,t5387,t5389,t539,t5390,t5391,t5392,t5393,t5394,t5395,t540,t5402,t5404,t5409,t5416,t5420,t543,t5433,t5435,t5436,t544,t5440,t5441,t5442,t5443,t5444,t5445,t5446,t5448,t545,t5450,t5451,t5453,t5454,t5457,t5459,t546,t5463,t5464,t5465,t5466,t547,t5473,t5475,t5479,t548,t5480,t5481,t5482,t5483,t5484,t5485,t5486,t5487,t5488,t5489,t549,t5490,t5491,t5492,t5493,t5494,t5496,t5498,t5499,t5501,t5507,t551,t5512,t5516,t5517,t5519,t552,t5521,t5522,t5526,t5527,t553,t5534,t554,t5540,t5546,t5549,t555,t5552,t5555,t5559,t556,t5561,t5562,t5563,t5565,t5566,t5569,t557,t5573,t5578,t558,t5580,t5581,t5583,t5584,t5589,t559,t5590,t5593,t5594,t5596,t5597,t560,t5600,t5603,t5604,t5606,t5607,t561,t5611,t5612,t5618,t562,t5629,t563,t5633,t5634,t5635,t564,t5656,t5660,t5667,t5668,t567,t5673,t5678,t568,t5688,t569,t57,t570,t571,t572,t573,t574,t5741,t5743,t576,t577,t5777,t5779,t578,t5780,t5782,t579,t58,t580,t581,t5818,t5819,t582,t5823,t5826,t583,t584,t586,t587,t5886,t5887,t589,t5894,t59,t590,t591,t592,t593,t594,t595,t596,t597,t6,t60,t600,t602,t603,t604,t605,t609,t610,t611,t612,t613,t614,t615,t616,t618,t619,t620,t621,t622,t623,t624,t625,t626,t627,t628,t629,t63,t630,t631,t632,t633,t634,t635,t636,t637,t638,t639,t640,t641,t642,t643,t645,t646,t647,t648,t649,t650,t653,t654,t655,t656,t657,t658,t660,t662,t663,t664,t665,t667,t668,t669,t673,t674,t675,t676,t679,t680,t681,t682,t683,t684,t685,t686,t687,t688,t689,t691,t692,t693,t694,t695,t696,t697,t698,t7,t700,t702,t703,t704,t705,t706,t708,t71,t710,t711,t712,t713,t7148,t715,t716,t72,t724,t728,t73,t731,t733,t734,t735,t736,t738,t739,t74,t740,t741,t742,t743,t744,t746,t747,t748,t749,t75,t750,t751,t752,t753,t754,t755,t756,t757,t758,t759,t76,t760,t762,t763,t764,t765,t766,t767,t768,t769,t77,t772,t773,t774,t775,t776,t777,t778,t779,t780,t781,t782,t784,t785,t786,t792,t794,t795,t796,t797,t798,t799,t8,t80,t801,t802,t804,t805,t806,t808,t81,t814,t815,t817,t82,t820,t822,t823,t824,t825,t826,t827,t829,t83,t830,t831,t832,t833,t834,t835,t836,t837,t838,t84,t840,t841,t842,t843,t844,t845,t846,t847,t852,t853,t856,t858,t859,t86,t861,t863,t865,t866,t867,t868,t869,t870,t874,t875,t876,t877,t878,t880,t881,t882,t884,t885,t888,t891,t895,t899,t9,t90,t900,t902,t903,t906,t909,t91,t910,t911,t914,t916,t917,t920,t921,t922,t923,t925,t926,t927,t928,t929,t930,t934,t935,t937,t940,t941,t942,t943,t944,t945,t946,t947,t949,t95,t950,t951,t952,t953,t954,t955,t957,t958,t961,t962,t963,t964,t965,t968,t97,t970,t971,t972,t973,t974,t975,t976,t977,t982,t983,t984,t986,t987,t988,t989,t99,t991,t993,t994,t995,t999});
end
function C_dq = ft_10(ct)
dq1 = ct{1};
dq2 = ct{2};
dq3 = ct{3};
dq4 = ct{4};
dq5 = ct{5};
dq6 = ct{6};
t1004 = ct{7};
t1006 = ct{8};
t1008 = ct{9};
t101 = ct{10};
t1013 = ct{11};
t1016 = ct{12};
t1017 = ct{13};
t1019 = ct{14};
t102 = ct{15};
t1020 = ct{16};
t1021 = ct{17};
t1023 = ct{18};
t1024 = ct{19};
t1025 = ct{20};
t1026 = ct{21};
t1028 = ct{22};
t1030 = ct{23};
t1032 = ct{24};
t1034 = ct{25};
t1036 = ct{26};
t1038 = ct{27};
t1039 = ct{28};
t1040 = ct{29};
t1042 = ct{30};
t1043 = ct{31};
t1044 = ct{32};
t1045 = ct{33};
t1046 = ct{34};
t1047 = ct{35};
t1048 = ct{36};
t1049 = ct{37};
t1050 = ct{38};
t1051 = ct{39};
t1054 = ct{40};
t1055 = ct{41};
t1056 = ct{42};
t1057 = ct{43};
t1059 = ct{44};
t1061 = ct{45};
t1065 = ct{46};
t1066 = ct{47};
t1068 = ct{48};
t1069 = ct{49};
t1070 = ct{50};
t1072 = ct{51};
t1073 = ct{52};
t1075 = ct{53};
t1076 = ct{54};
t1077 = ct{55};
t1081 = ct{56};
t1083 = ct{57};
t1084 = ct{58};
t1085 = ct{59};
t1087 = ct{60};
t1089 = ct{61};
t1091 = ct{62};
t1092 = ct{63};
t1093 = ct{64};
t1095 = ct{65};
t1098 = ct{66};
t1099 = ct{67};
t110 = ct{68};
t1101 = ct{69};
t1102 = ct{70};
t1105 = ct{71};
t1106 = ct{72};
t1107 = ct{73};
t1108 = ct{74};
t1109 = ct{75};
t111 = ct{76};
t1113 = ct{77};
t1115 = ct{78};
t1116 = ct{79};
t1119 = ct{80};
t112 = ct{81};
t1122 = ct{82};
t1125 = ct{83};
t1126 = ct{84};
t1127 = ct{85};
t1128 = ct{86};
t113 = ct{87};
t1130 = ct{88};
t1131 = ct{89};
t1133 = ct{90};
t1134 = ct{91};
t1135 = ct{92};
t1138 = ct{93};
t1139 = ct{94};
t114 = ct{95};
t1141 = ct{96};
t1144 = ct{97};
t1145 = ct{98};
t1146 = ct{99};
t1147 = ct{100};
t1148 = ct{101};
t1149 = ct{102};
t115 = ct{103};
t1150 = ct{104};
t1152 = ct{105};
t1153 = ct{106};
t1155 = ct{107};
t1158 = ct{108};
t1159 = ct{109};
t116 = ct{110};
t1162 = ct{111};
t1163 = ct{112};
t1165 = ct{113};
t1167 = ct{114};
t1169 = ct{115};
t1170 = ct{116};
t1171 = ct{117};
t1173 = ct{118};
t1174 = ct{119};
t1175 = ct{120};
t1177 = ct{121};
t1178 = ct{122};
t1179 = ct{123};
t1180 = ct{124};
t1181 = ct{125};
t1182 = ct{126};
t1183 = ct{127};
t1184 = ct{128};
t1185 = ct{129};
t1186 = ct{130};
t1188 = ct{131};
t1189 = ct{132};
t1190 = ct{133};
t1191 = ct{134};
t1192 = ct{135};
t1193 = ct{136};
t1194 = ct{137};
t1196 = ct{138};
t1197 = ct{139};
t1198 = ct{140};
t1199 = ct{141};
t120 = ct{142};
t1200 = ct{143};
t1202 = ct{144};
t1203 = ct{145};
t1204 = ct{146};
t1205 = ct{147};
t1206 = ct{148};
t1207 = ct{149};
t121 = ct{150};
t1210 = ct{151};
t1211 = ct{152};
t1215 = ct{153};
t1219 = ct{154};
t1221 = ct{155};
t1222 = ct{156};
t1224 = ct{157};
t1225 = ct{158};
t1227 = ct{159};
t1228 = ct{160};
t1233 = ct{161};
t1235 = ct{162};
t1236 = ct{163};
t1237 = ct{164};
t1239 = ct{165};
t124 = ct{166};
t1240 = ct{167};
t1241 = ct{168};
t1244 = ct{169};
t1245 = ct{170};
t125 = ct{171};
t1250 = ct{172};
t1251 = ct{173};
t1253 = ct{174};
t1254 = ct{175};
t1256 = ct{176};
t1257 = ct{177};
t1258 = ct{178};
t1259 = ct{179};
t126 = ct{180};
t1261 = ct{181};
t1262 = ct{182};
t1263 = ct{183};
t1264 = ct{184};
t1265 = ct{185};
t1266 = ct{186};
t1267 = ct{187};
t1268 = ct{188};
t1269 = ct{189};
t1271 = ct{190};
t1272 = ct{191};
t1273 = ct{192};
t1274 = ct{193};
t1277 = ct{194};
t1278 = ct{195};
t128 = ct{196};
t1280 = ct{197};
t1282 = ct{198};
t1285 = ct{199};
t1286 = ct{200};
t1288 = ct{201};
t129 = ct{202};
t1290 = ct{203};
t1293 = ct{204};
t1294 = ct{205};
t1295 = ct{206};
t1296 = ct{207};
t1298 = ct{208};
t1300 = ct{209};
t1301 = ct{210};
t1302 = ct{211};
t1306 = ct{212};
t1307 = ct{213};
t1308 = ct{214};
t1309 = ct{215};
t131 = ct{216};
t1311 = ct{217};
t1312 = ct{218};
t1313 = ct{219};
t1315 = ct{220};
t1316 = ct{221};
t1317 = ct{222};
t1318 = ct{223};
t1319 = ct{224};
t132 = ct{225};
t1322 = ct{226};
t1323 = ct{227};
t1324 = ct{228};
t1325 = ct{229};
t1326 = ct{230};
t1328 = ct{231};
t1329 = ct{232};
t133 = ct{233};
t1330 = ct{234};
t1331 = ct{235};
t1333 = ct{236};
t1334 = ct{237};
t1337 = ct{238};
t1338 = ct{239};
t1340 = ct{240};
t1341 = ct{241};
t1342 = ct{242};
t1343 = ct{243};
t1344 = ct{244};
t1345 = ct{245};
t1346 = ct{246};
t1348 = ct{247};
t1351 = ct{248};
t1352 = ct{249};
t1353 = ct{250};
t1354 = ct{251};
t1355 = ct{252};
t1356 = ct{253};
t1360 = ct{254};
t1362 = ct{255};
t1365 = ct{256};
t1366 = ct{257};
t1367 = ct{258};
t1369 = ct{259};
t1370 = ct{260};
t1371 = ct{261};
t1372 = ct{262};
t1374 = ct{263};
t1375 = ct{264};
t1377 = ct{265};
t1378 = ct{266};
t1379 = ct{267};
t1380 = ct{268};
t1383 = ct{269};
t1384 = ct{270};
t1385 = ct{271};
t1386 = ct{272};
t1388 = ct{273};
t1389 = ct{274};
t139 = ct{275};
t1391 = ct{276};
t1392 = ct{277};
t1393 = ct{278};
t1394 = ct{279};
t1397 = ct{280};
t1398 = ct{281};
t140 = ct{282};
t1401 = ct{283};
t1402 = ct{284};
t1403 = ct{285};
t1404 = ct{286};
t1406 = ct{287};
t1407 = ct{288};
t1408 = ct{289};
t1409 = ct{290};
t141 = ct{291};
t1410 = ct{292};
t1411 = ct{293};
t1413 = ct{294};
t1414 = ct{295};
t1415 = ct{296};
t1416 = ct{297};
t1417 = ct{298};
t1419 = ct{299};
t142 = ct{300};
t1422 = ct{301};
t1423 = ct{302};
t1426 = ct{303};
t1427 = ct{304};
t1428 = ct{305};
t1429 = ct{306};
t1430 = ct{307};
t1431 = ct{308};
t1432 = ct{309};
t1433 = ct{310};
t1436 = ct{311};
t144 = ct{312};
t1440 = ct{313};
t1441 = ct{314};
t1442 = ct{315};
t1443 = ct{316};
t1445 = ct{317};
t1446 = ct{318};
t1447 = ct{319};
t1448 = ct{320};
t1449 = ct{321};
t1451 = ct{322};
t1452 = ct{323};
t1453 = ct{324};
t1454 = ct{325};
t1455 = ct{326};
t1456 = ct{327};
t1457 = ct{328};
t1458 = ct{329};
t1459 = ct{330};
t1460 = ct{331};
t1463 = ct{332};
t1464 = ct{333};
t1465 = ct{334};
t1467 = ct{335};
t1470 = ct{336};
t1471 = ct{337};
t1474 = ct{338};
t1476 = ct{339};
t1478 = ct{340};
t1479 = ct{341};
t148 = ct{342};
t1480 = ct{343};
t1481 = ct{344};
t1482 = ct{345};
t1483 = ct{346};
t1486 = ct{347};
t1487 = ct{348};
t1488 = ct{349};
t1489 = ct{350};
t1490 = ct{351};
t1491 = ct{352};
t1492 = ct{353};
t1493 = ct{354};
t1494 = ct{355};
t1495 = ct{356};
t1496 = ct{357};
t1498 = ct{358};
t1499 = ct{359};
t15 = ct{360};
t150 = ct{361};
t1500 = ct{362};
t1501 = ct{363};
t1503 = ct{364};
t1505 = ct{365};
t1506 = ct{366};
t1507 = ct{367};
t1508 = ct{368};
t1509 = ct{369};
t151 = ct{370};
t1510 = ct{371};
t1511 = ct{372};
t1512 = ct{373};
t1513 = ct{374};
t1515 = ct{375};
t1517 = ct{376};
t1520 = ct{377};
t1521 = ct{378};
t1522 = ct{379};
t1523 = ct{380};
t1524 = ct{381};
t1526 = ct{382};
t1527 = ct{383};
t1529 = ct{384};
t153 = ct{385};
t1530 = ct{386};
t1531 = ct{387};
t1532 = ct{388};
t1533 = ct{389};
t1534 = ct{390};
t1535 = ct{391};
t1536 = ct{392};
t1537 = ct{393};
t1538 = ct{394};
t1539 = ct{395};
t154 = ct{396};
t1540 = ct{397};
t1541 = ct{398};
t1542 = ct{399};
t1548 = ct{400};
t1549 = ct{401};
t1550 = ct{402};
t1551 = ct{403};
t1553 = ct{404};
t1558 = ct{405};
t156 = ct{406};
t1560 = ct{407};
t1561 = ct{408};
t1562 = ct{409};
t1564 = ct{410};
t1566 = ct{411};
t1567 = ct{412};
t1568 = ct{413};
t157 = ct{414};
t1570 = ct{415};
t1571 = ct{416};
t1572 = ct{417};
t1574 = ct{418};
t1575 = ct{419};
t1576 = ct{420};
t1577 = ct{421};
t1578 = ct{422};
t1579 = ct{423};
t158 = ct{424};
t1580 = ct{425};
t1581 = ct{426};
t1582 = ct{427};
t1583 = ct{428};
t1584 = ct{429};
t1585 = ct{430};
t1586 = ct{431};
t1587 = ct{432};
t1589 = ct{433};
t1590 = ct{434};
t1591 = ct{435};
t1592 = ct{436};
t1593 = ct{437};
t1594 = ct{438};
t1595 = ct{439};
t1596 = ct{440};
t1597 = ct{441};
t1598 = ct{442};
t1599 = ct{443};
t16 = ct{444};
t1601 = ct{445};
t1602 = ct{446};
t1605 = ct{447};
t1606 = ct{448};
t1607 = ct{449};
t1609 = ct{450};
t161 = ct{451};
t1610 = ct{452};
t1611 = ct{453};
t1612 = ct{454};
t1613 = ct{455};
t1614 = ct{456};
t1615 = ct{457};
t1616 = ct{458};
t1617 = ct{459};
t1618 = ct{460};
t1619 = ct{461};
t1620 = ct{462};
t1621 = ct{463};
t1622 = ct{464};
t1625 = ct{465};
t1626 = ct{466};
t1627 = ct{467};
t163 = ct{468};
t1630 = ct{469};
t1631 = ct{470};
t1632 = ct{471};
t1633 = ct{472};
t1635 = ct{473};
t1636 = ct{474};
t1637 = ct{475};
t1638 = ct{476};
t1639 = ct{477};
t1641 = ct{478};
t1642 = ct{479};
t1643 = ct{480};
t1644 = ct{481};
t1645 = ct{482};
t1646 = ct{483};
t1647 = ct{484};
t1648 = ct{485};
t165 = ct{486};
t1651 = ct{487};
t1652 = ct{488};
t1653 = ct{489};
t1657 = ct{490};
t1658 = ct{491};
t1659 = ct{492};
t166 = ct{493};
t1660 = ct{494};
t1661 = ct{495};
t1662 = ct{496};
t1663 = ct{497};
t1666 = ct{498};
t1667 = ct{499};
t1669 = ct{500};
t1670 = ct{501};
t1671 = ct{502};
t1672 = ct{503};
t1673 = ct{504};
t1674 = ct{505};
t1675 = ct{506};
t1676 = ct{507};
t1681 = ct{508};
t1682 = ct{509};
t1683 = ct{510};
t1686 = ct{511};
t1687 = ct{512};
t1689 = ct{513};
t1691 = ct{514};
t1692 = ct{515};
t1696 = ct{516};
t1697 = ct{517};
t1698 = ct{518};
t1699 = ct{519};
t17 = ct{520};
t170 = ct{521};
t1700 = ct{522};
t1701 = ct{523};
t1702 = ct{524};
t1703 = ct{525};
t1704 = ct{526};
t1705 = ct{527};
t1706 = ct{528};
t1709 = ct{529};
t171 = ct{530};
t1710 = ct{531};
t1711 = ct{532};
t1712 = ct{533};
t1713 = ct{534};
t1715 = ct{535};
t1716 = ct{536};
t1718 = ct{537};
t1719 = ct{538};
t1720 = ct{539};
t1721 = ct{540};
t1722 = ct{541};
t1723 = ct{542};
t1724 = ct{543};
t1726 = ct{544};
t1728 = ct{545};
t1729 = ct{546};
t1731 = ct{547};
t1733 = ct{548};
t1734 = ct{549};
t1735 = ct{550};
t1736 = ct{551};
t1737 = ct{552};
t1738 = ct{553};
t1739 = ct{554};
t1740 = ct{555};
t1741 = ct{556};
t1745 = ct{557};
t1746 = ct{558};
t1747 = ct{559};
t1748 = ct{560};
t1749 = ct{561};
t1752 = ct{562};
t1753 = ct{563};
t1754 = ct{564};
t1755 = ct{565};
t1756 = ct{566};
t1757 = ct{567};
t1758 = ct{568};
t1759 = ct{569};
t1760 = ct{570};
t1761 = ct{571};
t1763 = ct{572};
t1764 = ct{573};
t1765 = ct{574};
t1766 = ct{575};
t1767 = ct{576};
t1768 = ct{577};
t1769 = ct{578};
t177 = ct{579};
t1770 = ct{580};
t1771 = ct{581};
t1772 = ct{582};
t1774 = ct{583};
t1775 = ct{584};
t1776 = ct{585};
t1777 = ct{586};
t1779 = ct{587};
t1780 = ct{588};
t1781 = ct{589};
t1783 = ct{590};
t1784 = ct{591};
t1785 = ct{592};
t1786 = ct{593};
t1787 = ct{594};
t1788 = ct{595};
t1789 = ct{596};
t1790 = ct{597};
t1791 = ct{598};
t1792 = ct{599};
t1793 = ct{600};
t1794 = ct{601};
t1795 = ct{602};
t1797 = ct{603};
t1798 = ct{604};
t1799 = ct{605};
t18 = ct{606};
t1800 = ct{607};
t1801 = ct{608};
t1804 = ct{609};
t1805 = ct{610};
t1806 = ct{611};
t1807 = ct{612};
t1808 = ct{613};
t1809 = ct{614};
t1810 = ct{615};
t1811 = ct{616};
t1812 = ct{617};
t1813 = ct{618};
t1814 = ct{619};
t1815 = ct{620};
t1816 = ct{621};
t1817 = ct{622};
t1820 = ct{623};
t1822 = ct{624};
t1823 = ct{625};
t1824 = ct{626};
t1827 = ct{627};
t1828 = ct{628};
t1829 = ct{629};
t183 = ct{630};
t1830 = ct{631};
t1831 = ct{632};
t1832 = ct{633};
t1833 = ct{634};
t1834 = ct{635};
t1835 = ct{636};
t1836 = ct{637};
t1837 = ct{638};
t1838 = ct{639};
t1839 = ct{640};
t1844 = ct{641};
t1845 = ct{642};
t1846 = ct{643};
t1847 = ct{644};
t1848 = ct{645};
t1849 = ct{646};
t185 = ct{647};
t1850 = ct{648};
t1851 = ct{649};
t1853 = ct{650};
t1855 = ct{651};
t1856 = ct{652};
t1857 = ct{653};
t1858 = ct{654};
t1859 = ct{655};
t1861 = ct{656};
t1864 = ct{657};
t1865 = ct{658};
t1866 = ct{659};
t1867 = ct{660};
t1871 = ct{661};
t1873 = ct{662};
t1877 = ct{663};
t1879 = ct{664};
t1881 = ct{665};
t1882 = ct{666};
t1884 = ct{667};
t1885 = ct{668};
t1886 = ct{669};
t1887 = ct{670};
t1889 = ct{671};
t1891 = ct{672};
t1892 = ct{673};
t1893 = ct{674};
t1896 = ct{675};
t19 = ct{676};
t190 = ct{677};
t1900 = ct{678};
t1902 = ct{679};
t1903 = ct{680};
t1905 = ct{681};
t1906 = ct{682};
t1907 = ct{683};
t1908 = ct{684};
t1909 = ct{685};
t191 = ct{686};
t1910 = ct{687};
t1911 = ct{688};
t1912 = ct{689};
t1913 = ct{690};
t1914 = ct{691};
t1915 = ct{692};
t1916 = ct{693};
t1917 = ct{694};
t1918 = ct{695};
t1919 = ct{696};
t1920 = ct{697};
t1921 = ct{698};
t1925 = ct{699};
t1926 = ct{700};
t1927 = ct{701};
t1928 = ct{702};
t1930 = ct{703};
t1934 = ct{704};
t1935 = ct{705};
t1936 = ct{706};
t1937 = ct{707};
t1938 = ct{708};
t1939 = ct{709};
t1942 = ct{710};
t1943 = ct{711};
t1944 = ct{712};
t1946 = ct{713};
t1947 = ct{714};
t1950 = ct{715};
t1951 = ct{716};
t1952 = ct{717};
t1953 = ct{718};
t1954 = ct{719};
t1955 = ct{720};
t196 = ct{721};
t1961 = ct{722};
t1966 = ct{723};
t1967 = ct{724};
t1968 = ct{725};
t1969 = ct{726};
t197 = ct{727};
t1970 = ct{728};
t1971 = ct{729};
t1975 = ct{730};
t1976 = ct{731};
t1977 = ct{732};
t1978 = ct{733};
t1979 = ct{734};
t1980 = ct{735};
t1981 = ct{736};
t1983 = ct{737};
t1984 = ct{738};
t1985 = ct{739};
t1986 = ct{740};
t1987 = ct{741};
t1988 = ct{742};
t1989 = ct{743};
t199 = ct{744};
t1991 = ct{745};
t1992 = ct{746};
t1993 = ct{747};
t1994 = ct{748};
t1995 = ct{749};
t1996 = ct{750};
t1997 = ct{751};
t1998 = ct{752};
t1999 = ct{753};
t2 = ct{754};
t20 = ct{755};
t200 = ct{756};
t2000 = ct{757};
t2001 = ct{758};
t2002 = ct{759};
t2003 = ct{760};
t2004 = ct{761};
t2005 = ct{762};
t2006 = ct{763};
t2008 = ct{764};
t201 = ct{765};
t2011 = ct{766};
t2014 = ct{767};
t2015 = ct{768};
t2016 = ct{769};
t2017 = ct{770};
t2018 = ct{771};
t2019 = ct{772};
t202 = ct{773};
t2020 = ct{774};
t2023 = ct{775};
t2024 = ct{776};
t2026 = ct{777};
t2027 = ct{778};
t2028 = ct{779};
t2029 = ct{780};
t203 = ct{781};
t2033 = ct{782};
t2035 = ct{783};
t2036 = ct{784};
t2037 = ct{785};
t2038 = ct{786};
t204 = ct{787};
t2040 = ct{788};
t2042 = ct{789};
t2043 = ct{790};
t2045 = ct{791};
t2047 = ct{792};
t2049 = ct{793};
t205 = ct{794};
t2050 = ct{795};
t2051 = ct{796};
t2052 = ct{797};
t2053 = ct{798};
t2054 = ct{799};
t2056 = ct{800};
t2057 = ct{801};
t2058 = ct{802};
t2059 = ct{803};
t206 = ct{804};
t2060 = ct{805};
t2061 = ct{806};
t2062 = ct{807};
t2065 = ct{808};
t2066 = ct{809};
t2067 = ct{810};
t2068 = ct{811};
t2069 = ct{812};
t207 = ct{813};
t2070 = ct{814};
t2071 = ct{815};
t2072 = ct{816};
t2073 = ct{817};
t2074 = ct{818};
t2075 = ct{819};
t2076 = ct{820};
t2077 = ct{821};
t2078 = ct{822};
t2079 = ct{823};
t208 = ct{824};
t2081 = ct{825};
t2082 = ct{826};
t2083 = ct{827};
t2084 = ct{828};
t2085 = ct{829};
t2086 = ct{830};
t2087 = ct{831};
t2088 = ct{832};
t2089 = ct{833};
t209 = ct{834};
t2090 = ct{835};
t2091 = ct{836};
t2092 = ct{837};
t2093 = ct{838};
t2094 = ct{839};
t2095 = ct{840};
t2096 = ct{841};
t2097 = ct{842};
t2098 = ct{843};
t2099 = ct{844};
t21 = ct{845};
t210 = ct{846};
t2100 = ct{847};
t2101 = ct{848};
t2104 = ct{849};
t2105 = ct{850};
t2106 = ct{851};
t2107 = ct{852};
t2108 = ct{853};
t2109 = ct{854};
t211 = ct{855};
t2110 = ct{856};
t2111 = ct{857};
t2113 = ct{858};
t2114 = ct{859};
t2115 = ct{860};
t2116 = ct{861};
t2117 = ct{862};
t2118 = ct{863};
t2119 = ct{864};
t212 = ct{865};
t2121 = ct{866};
t2123 = ct{867};
t2125 = ct{868};
t2127 = ct{869};
t2128 = ct{870};
t2129 = ct{871};
t213 = ct{872};
t2130 = ct{873};
t2131 = ct{874};
t2132 = ct{875};
t2133 = ct{876};
t2134 = ct{877};
t2135 = ct{878};
t2136 = ct{879};
t2137 = ct{880};
t2138 = ct{881};
t2142 = ct{882};
t2143 = ct{883};
t2144 = ct{884};
t2146 = ct{885};
t2148 = ct{886};
t2149 = ct{887};
t2150 = ct{888};
t2151 = ct{889};
t2152 = ct{890};
t2154 = ct{891};
t2155 = ct{892};
t2156 = ct{893};
t2157 = ct{894};
t2158 = ct{895};
t2159 = ct{896};
t2160 = ct{897};
t2161 = ct{898};
t2164 = ct{899};
t2165 = ct{900};
t2166 = ct{901};
t2169 = ct{902};
t2170 = ct{903};
t2171 = ct{904};
t2172 = ct{905};
t2174 = ct{906};
t2175 = ct{907};
t2176 = ct{908};
t2177 = ct{909};
t2178 = ct{910};
t2180 = ct{911};
t2181 = ct{912};
t2182 = ct{913};
t2184 = ct{914};
t2185 = ct{915};
t2186 = ct{916};
t2187 = ct{917};
t2189 = ct{918};
t2190 = ct{919};
t2191 = ct{920};
t2192 = ct{921};
t2193 = ct{922};
t2194 = ct{923};
t2196 = ct{924};
t2197 = ct{925};
t2198 = ct{926};
t2199 = ct{927};
t22 = ct{928};
t2200 = ct{929};
t2201 = ct{930};
t2202 = ct{931};
t2203 = ct{932};
t2204 = ct{933};
t2208 = ct{934};
t2209 = ct{935};
t2211 = ct{936};
t2212 = ct{937};
t2213 = ct{938};
t2214 = ct{939};
t2215 = ct{940};
t2216 = ct{941};
t2217 = ct{942};
t2218 = ct{943};
t2219 = ct{944};
t2220 = ct{945};
t2221 = ct{946};
t2223 = ct{947};
t2224 = ct{948};
t2225 = ct{949};
t2227 = ct{950};
t2228 = ct{951};
t2229 = ct{952};
t2230 = ct{953};
t2231 = ct{954};
t2232 = ct{955};
t2236 = ct{956};
t2237 = ct{957};
t2238 = ct{958};
t2239 = ct{959};
t224 = ct{960};
t2240 = ct{961};
t2241 = ct{962};
t2243 = ct{963};
t2246 = ct{964};
t2247 = ct{965};
t2248 = ct{966};
t2249 = ct{967};
t225 = ct{968};
t2251 = ct{969};
t2253 = ct{970};
t2254 = ct{971};
t2256 = ct{972};
t2257 = ct{973};
t2258 = ct{974};
t2259 = ct{975};
t2260 = ct{976};
t2261 = ct{977};
t2262 = ct{978};
t2263 = ct{979};
t2264 = ct{980};
t2265 = ct{981};
t2266 = ct{982};
t2267 = ct{983};
t2268 = ct{984};
t2269 = ct{985};
t227 = ct{986};
t2270 = ct{987};
t2271 = ct{988};
t2272 = ct{989};
t2273 = ct{990};
t2274 = ct{991};
t2276 = ct{992};
t2277 = ct{993};
t2278 = ct{994};
t2279 = ct{995};
t228 = ct{996};
t2280 = ct{997};
t2281 = ct{998};
t2282 = ct{999};
t2283 = ct{1000};
t2284 = ct{1001};
t2285 = ct{1002};
t2286 = ct{1003};
t2288 = ct{1004};
t2289 = ct{1005};
t2290 = ct{1006};
t2291 = ct{1007};
t2293 = ct{1008};
t2295 = ct{1009};
t2296 = ct{1010};
t23 = ct{1011};
t230 = ct{1012};
t2301 = ct{1013};
t2302 = ct{1014};
t2303 = ct{1015};
t2304 = ct{1016};
t2305 = ct{1017};
t2306 = ct{1018};
t2307 = ct{1019};
t2308 = ct{1020};
t231 = ct{1021};
t2310 = ct{1022};
t2311 = ct{1023};
t2312 = ct{1024};
t2313 = ct{1025};
t2314 = ct{1026};
t2315 = ct{1027};
t2316 = ct{1028};
t2317 = ct{1029};
t2318 = ct{1030};
t2319 = ct{1031};
t2320 = ct{1032};
t2321 = ct{1033};
t2322 = ct{1034};
t2323 = ct{1035};
t2324 = ct{1036};
t2326 = ct{1037};
t2327 = ct{1038};
t233 = ct{1039};
t2331 = ct{1040};
t2333 = ct{1041};
t2334 = ct{1042};
t2336 = ct{1043};
t2337 = ct{1044};
t2338 = ct{1045};
t2339 = ct{1046};
t234 = ct{1047};
t2340 = ct{1048};
t2341 = ct{1049};
t2342 = ct{1050};
t2344 = ct{1051};
t2345 = ct{1052};
t2346 = ct{1053};
t2347 = ct{1054};
t2348 = ct{1055};
t235 = ct{1056};
t2350 = ct{1057};
t2355 = ct{1058};
t2357 = ct{1059};
t2358 = ct{1060};
t2359 = ct{1061};
t236 = ct{1062};
t2361 = ct{1063};
t2362 = ct{1064};
t2363 = ct{1065};
t2364 = ct{1066};
t2365 = ct{1067};
t2366 = ct{1068};
t2367 = ct{1069};
t2369 = ct{1070};
t2370 = ct{1071};
t2371 = ct{1072};
t2372 = ct{1073};
t2373 = ct{1074};
t2374 = ct{1075};
t2375 = ct{1076};
t2376 = ct{1077};
t2377 = ct{1078};
t2378 = ct{1079};
t2379 = ct{1080};
t2382 = ct{1081};
t2383 = ct{1082};
t2384 = ct{1083};
t2385 = ct{1084};
t2386 = ct{1085};
t2387 = ct{1086};
t2388 = ct{1087};
t2389 = ct{1088};
t2390 = ct{1089};
t2391 = ct{1090};
t2392 = ct{1091};
t2393 = ct{1092};
t2394 = ct{1093};
t2395 = ct{1094};
t2396 = ct{1095};
t2397 = ct{1096};
t2398 = ct{1097};
t24 = ct{1098};
t240 = ct{1099};
t2400 = ct{1100};
t2401 = ct{1101};
t2402 = ct{1102};
t2403 = ct{1103};
t2404 = ct{1104};
t2405 = ct{1105};
t2406 = ct{1106};
t2407 = ct{1107};
t2408 = ct{1108};
t2410 = ct{1109};
t2416 = ct{1110};
t2417 = ct{1111};
t2420 = ct{1112};
t2421 = ct{1113};
t2422 = ct{1114};
t2424 = ct{1115};
t2425 = ct{1116};
t2426 = ct{1117};
t2427 = ct{1118};
t2428 = ct{1119};
t2429 = ct{1120};
t243 = ct{1121};
t2430 = ct{1122};
t2431 = ct{1123};
t2434 = ct{1124};
t2435 = ct{1125};
t2437 = ct{1126};
t2438 = ct{1127};
t2439 = ct{1128};
t244 = ct{1129};
t2440 = ct{1130};
t2441 = ct{1131};
t2443 = ct{1132};
t2444 = ct{1133};
t2445 = ct{1134};
t2446 = ct{1135};
t2448 = ct{1136};
t2449 = ct{1137};
t2452 = ct{1138};
t2453 = ct{1139};
t2454 = ct{1140};
t2455 = ct{1141};
t2456 = ct{1142};
t2457 = ct{1143};
t2458 = ct{1144};
t2459 = ct{1145};
t2460 = ct{1146};
t2461 = ct{1147};
t2463 = ct{1148};
t2464 = ct{1149};
t2465 = ct{1150};
t2466 = ct{1151};
t2467 = ct{1152};
t2469 = ct{1153};
t2470 = ct{1154};
t2472 = ct{1155};
t2474 = ct{1156};
t2477 = ct{1157};
t2478 = ct{1158};
t2479 = ct{1159};
t2481 = ct{1160};
t2483 = ct{1161};
t2484 = ct{1162};
t2485 = ct{1163};
t2486 = ct{1164};
t2487 = ct{1165};
t2489 = ct{1166};
t249 = ct{1167};
t2490 = ct{1168};
t2494 = ct{1169};
t2495 = ct{1170};
t2497 = ct{1171};
t2500 = ct{1172};
t2502 = ct{1173};
t2503 = ct{1174};
t2505 = ct{1175};
t2507 = ct{1176};
t2508 = ct{1177};
t2510 = ct{1178};
t2511 = ct{1179};
t2512 = ct{1180};
t2513 = ct{1181};
t2517 = ct{1182};
t2518 = ct{1183};
t2519 = ct{1184};
t2520 = ct{1185};
t2521 = ct{1186};
t2522 = ct{1187};
t2523 = ct{1188};
t2524 = ct{1189};
t2525 = ct{1190};
t2526 = ct{1191};
t2527 = ct{1192};
t2530 = ct{1193};
t2531 = ct{1194};
t2533 = ct{1195};
t2534 = ct{1196};
t2535 = ct{1197};
t2536 = ct{1198};
t2537 = ct{1199};
t2539 = ct{1200};
t2540 = ct{1201};
t2541 = ct{1202};
t2542 = ct{1203};
t2543 = ct{1204};
t2544 = ct{1205};
t2545 = ct{1206};
t2546 = ct{1207};
t2547 = ct{1208};
t2548 = ct{1209};
t2549 = ct{1210};
t2550 = ct{1211};
t2552 = ct{1212};
t2553 = ct{1213};
t2554 = ct{1214};
t2555 = ct{1215};
t2556 = ct{1216};
t2560 = ct{1217};
t2562 = ct{1218};
t2563 = ct{1219};
t2564 = ct{1220};
t2565 = ct{1221};
t2566 = ct{1222};
t2567 = ct{1223};
t2568 = ct{1224};
t2569 = ct{1225};
t257 = ct{1226};
t2570 = ct{1227};
t2571 = ct{1228};
t2574 = ct{1229};
t2575 = ct{1230};
t2576 = ct{1231};
t2577 = ct{1232};
t2578 = ct{1233};
t2579 = ct{1234};
t258 = ct{1235};
t2581 = ct{1236};
t2582 = ct{1237};
t2585 = ct{1238};
t2586 = ct{1239};
t2587 = ct{1240};
t2588 = ct{1241};
t2589 = ct{1242};
t2590 = ct{1243};
t2594 = ct{1244};
t2595 = ct{1245};
t2597 = ct{1246};
t2598 = ct{1247};
t2599 = ct{1248};
t2600 = ct{1249};
t2601 = ct{1250};
t2602 = ct{1251};
t2603 = ct{1252};
t2604 = ct{1253};
t2606 = ct{1254};
t2607 = ct{1255};
t2608 = ct{1256};
t2611 = ct{1257};
t2612 = ct{1258};
t2613 = ct{1259};
t2614 = ct{1260};
t2615 = ct{1261};
t2616 = ct{1262};
t2617 = ct{1263};
t2620 = ct{1264};
t2622 = ct{1265};
t2623 = ct{1266};
t2624 = ct{1267};
t2625 = ct{1268};
t2626 = ct{1269};
t2627 = ct{1270};
t2628 = ct{1271};
t2629 = ct{1272};
t263 = ct{1273};
t2630 = ct{1274};
t2631 = ct{1275};
t2632 = ct{1276};
t2633 = ct{1277};
t2634 = ct{1278};
t2636 = ct{1279};
t2639 = ct{1280};
t2640 = ct{1281};
t2641 = ct{1282};
t2643 = ct{1283};
t2644 = ct{1284};
t2647 = ct{1285};
t2648 = ct{1286};
t2649 = ct{1287};
t2650 = ct{1288};
t2651 = ct{1289};
t2654 = ct{1290};
t2655 = ct{1291};
t2656 = ct{1292};
t2657 = ct{1293};
t2659 = ct{1294};
t266 = ct{1295};
t2660 = ct{1296};
t2661 = ct{1297};
t2662 = ct{1298};
t2663 = ct{1299};
t2664 = ct{1300};
t2665 = ct{1301};
t2666 = ct{1302};
t2668 = ct{1303};
t2669 = ct{1304};
t2671 = ct{1305};
t2673 = ct{1306};
t2675 = ct{1307};
t2676 = ct{1308};
t2677 = ct{1309};
t2678 = ct{1310};
t2680 = ct{1311};
t2681 = ct{1312};
t2682 = ct{1313};
t2684 = ct{1314};
t2685 = ct{1315};
t2686 = ct{1316};
t2688 = ct{1317};
t2689 = ct{1318};
t2692 = ct{1319};
t2693 = ct{1320};
t2694 = ct{1321};
t2695 = ct{1322};
t2699 = ct{1323};
t270 = ct{1324};
t2705 = ct{1325};
t2706 = ct{1326};
t2707 = ct{1327};
t2708 = ct{1328};
t2719 = ct{1329};
t2720 = ct{1330};
t2721 = ct{1331};
t2722 = ct{1332};
t2723 = ct{1333};
t2724 = ct{1334};
t2725 = ct{1335};
t2726 = ct{1336};
t2729 = ct{1337};
t273 = ct{1338};
t2736 = ct{1339};
t2737 = ct{1340};
t2738 = ct{1341};
t274 = ct{1342};
t2740 = ct{1343};
t2741 = ct{1344};
t2742 = ct{1345};
t2743 = ct{1346};
t2744 = ct{1347};
t2745 = ct{1348};
t2746 = ct{1349};
t2747 = ct{1350};
t2748 = ct{1351};
t2749 = ct{1352};
t275 = ct{1353};
t2750 = ct{1354};
t2752 = ct{1355};
t2753 = ct{1356};
t2754 = ct{1357};
t2755 = ct{1358};
t2756 = ct{1359};
t2757 = ct{1360};
t2758 = ct{1361};
t2759 = ct{1362};
t276 = ct{1363};
t2760 = ct{1364};
t2761 = ct{1365};
t2762 = ct{1366};
t2763 = ct{1367};
t2764 = ct{1368};
t2765 = ct{1369};
t2766 = ct{1370};
t2767 = ct{1371};
t2769 = ct{1372};
t277 = ct{1373};
t2770 = ct{1374};
t2771 = ct{1375};
t2772 = ct{1376};
t2774 = ct{1377};
t2775 = ct{1378};
t2778 = ct{1379};
t278 = ct{1380};
t2780 = ct{1381};
t2783 = ct{1382};
t2784 = ct{1383};
t2785 = ct{1384};
t2790 = ct{1385};
t2791 = ct{1386};
t2792 = ct{1387};
t2793 = ct{1388};
t2795 = ct{1389};
t2796 = ct{1390};
t2797 = ct{1391};
t2798 = ct{1392};
t2799 = ct{1393};
t280 = ct{1394};
t2800 = ct{1395};
t2801 = ct{1396};
t2802 = ct{1397};
t2803 = ct{1398};
t2805 = ct{1399};
t2806 = ct{1400};
t2807 = ct{1401};
t2809 = ct{1402};
t2810 = ct{1403};
t2811 = ct{1404};
t2812 = ct{1405};
t2814 = ct{1406};
t2815 = ct{1407};
t2816 = ct{1408};
t2817 = ct{1409};
t2818 = ct{1410};
t2819 = ct{1411};
t2820 = ct{1412};
t2822 = ct{1413};
t2823 = ct{1414};
t2824 = ct{1415};
t2825 = ct{1416};
t2826 = ct{1417};
t2827 = ct{1418};
t2828 = ct{1419};
t2829 = ct{1420};
t2830 = ct{1421};
t2831 = ct{1422};
t2832 = ct{1423};
t2833 = ct{1424};
t2834 = ct{1425};
t2835 = ct{1426};
t2837 = ct{1427};
t2838 = ct{1428};
t2839 = ct{1429};
t284 = ct{1430};
t2841 = ct{1431};
t2842 = ct{1432};
t2843 = ct{1433};
t2844 = ct{1434};
t2845 = ct{1435};
t2846 = ct{1436};
t2852 = ct{1437};
t2854 = ct{1438};
t2857 = ct{1439};
t2859 = ct{1440};
t2860 = ct{1441};
t2861 = ct{1442};
t2863 = ct{1443};
t2864 = ct{1444};
t2865 = ct{1445};
t2867 = ct{1446};
t2868 = ct{1447};
t2869 = ct{1448};
t287 = ct{1449};
t2870 = ct{1450};
t2871 = ct{1451};
t2872 = ct{1452};
t2874 = ct{1453};
t2875 = ct{1454};
t2876 = ct{1455};
t2877 = ct{1456};
t2878 = ct{1457};
t2882 = ct{1458};
t2883 = ct{1459};
t2884 = ct{1460};
t2885 = ct{1461};
t2886 = ct{1462};
t2888 = ct{1463};
t2891 = ct{1464};
t2892 = ct{1465};
t2893 = ct{1466};
t2894 = ct{1467};
t2895 = ct{1468};
t2896 = ct{1469};
t2897 = ct{1470};
t29 = ct{1471};
t290 = ct{1472};
t2900 = ct{1473};
t2903 = ct{1474};
t2904 = ct{1475};
t2907 = ct{1476};
t2908 = ct{1477};
t291 = ct{1478};
t2910 = ct{1479};
t2911 = ct{1480};
t2914 = ct{1481};
t2918 = ct{1482};
t2919 = ct{1483};
t292 = ct{1484};
t2920 = ct{1485};
t2921 = ct{1486};
t2922 = ct{1487};
t2923 = ct{1488};
t2925 = ct{1489};
t2928 = ct{1490};
t2929 = ct{1491};
t2930 = ct{1492};
t2931 = ct{1493};
t2932 = ct{1494};
t2934 = ct{1495};
t2937 = ct{1496};
t294 = ct{1497};
t2940 = ct{1498};
t2941 = ct{1499};
t2942 = ct{1500};
t2944 = ct{1501};
t2945 = ct{1502};
t2946 = ct{1503};
t2947 = ct{1504};
t2949 = ct{1505};
t2950 = ct{1506};
t2951 = ct{1507};
t2952 = ct{1508};
t2954 = ct{1509};
t2955 = ct{1510};
t2956 = ct{1511};
t2957 = ct{1512};
t2958 = ct{1513};
t2959 = ct{1514};
t2962 = ct{1515};
t2965 = ct{1516};
t2966 = ct{1517};
t2967 = ct{1518};
t2968 = ct{1519};
t2969 = ct{1520};
t297 = ct{1521};
t2970 = ct{1522};
t2971 = ct{1523};
t2972 = ct{1524};
t2973 = ct{1525};
t2974 = ct{1526};
t2975 = ct{1527};
t2977 = ct{1528};
t2978 = ct{1529};
t2980 = ct{1530};
t2983 = ct{1531};
t2984 = ct{1532};
t2985 = ct{1533};
t2986 = ct{1534};
t2988 = ct{1535};
t2989 = ct{1536};
t299 = ct{1537};
t2991 = ct{1538};
t2992 = ct{1539};
t2993 = ct{1540};
t2994 = ct{1541};
t2995 = ct{1542};
t2996 = ct{1543};
t2997 = ct{1544};
t3 = ct{1545};
t30 = ct{1546};
t300 = ct{1547};
t3001 = ct{1548};
t3002 = ct{1549};
t3003 = ct{1550};
t3005 = ct{1551};
t3007 = ct{1552};
t3008 = ct{1553};
t3010 = ct{1554};
t3011 = ct{1555};
t3013 = ct{1556};
t3014 = ct{1557};
t3018 = ct{1558};
t3019 = ct{1559};
t302 = ct{1560};
t3020 = ct{1561};
t3021 = ct{1562};
t3022 = ct{1563};
t3024 = ct{1564};
t3025 = ct{1565};
t3027 = ct{1566};
t3029 = ct{1567};
t303 = ct{1568};
t3030 = ct{1569};
t3031 = ct{1570};
t3032 = ct{1571};
t3033 = ct{1572};
t3034 = ct{1573};
t3035 = ct{1574};
t3036 = ct{1575};
t3037 = ct{1576};
t3038 = ct{1577};
t304 = ct{1578};
t3041 = ct{1579};
t3043 = ct{1580};
t3044 = ct{1581};
t3046 = ct{1582};
t3047 = ct{1583};
t3048 = ct{1584};
t3049 = ct{1585};
t305 = ct{1586};
t3050 = ct{1587};
t3051 = ct{1588};
t3052 = ct{1589};
t3053 = ct{1590};
t3054 = ct{1591};
t3055 = ct{1592};
t3056 = ct{1593};
t3057 = ct{1594};
t3059 = ct{1595};
t306 = ct{1596};
t3060 = ct{1597};
t3061 = ct{1598};
t3062 = ct{1599};
t3064 = ct{1600};
t3065 = ct{1601};
t3066 = ct{1602};
t3067 = ct{1603};
t3068 = ct{1604};
t3069 = ct{1605};
t3070 = ct{1606};
t3071 = ct{1607};
t3072 = ct{1608};
t3073 = ct{1609};
t3074 = ct{1610};
t3076 = ct{1611};
t3077 = ct{1612};
t3079 = ct{1613};
t3080 = ct{1614};
t3081 = ct{1615};
t3082 = ct{1616};
t3083 = ct{1617};
t3084 = ct{1618};
t3085 = ct{1619};
t3086 = ct{1620};
t3088 = ct{1621};
t3089 = ct{1622};
t309 = ct{1623};
t3090 = ct{1624};
t3092 = ct{1625};
t3094 = ct{1626};
t3095 = ct{1627};
t3096 = ct{1628};
t3097 = ct{1629};
t3098 = ct{1630};
t3099 = ct{1631};
t310 = ct{1632};
t3100 = ct{1633};
t3102 = ct{1634};
t3103 = ct{1635};
t3104 = ct{1636};
t3105 = ct{1637};
t3106 = ct{1638};
t3107 = ct{1639};
t3108 = ct{1640};
t3109 = ct{1641};
t311 = ct{1642};
t3110 = ct{1643};
t3112 = ct{1644};
t3113 = ct{1645};
t3114 = ct{1646};
t3117 = ct{1647};
t3118 = ct{1648};
t3119 = ct{1649};
t3120 = ct{1650};
t3121 = ct{1651};
t3122 = ct{1652};
t3123 = ct{1653};
t3124 = ct{1654};
t3126 = ct{1655};
t3127 = ct{1656};
t3128 = ct{1657};
t313 = ct{1658};
t3130 = ct{1659};
t3131 = ct{1660};
t3132 = ct{1661};
t3133 = ct{1662};
t3134 = ct{1663};
t3135 = ct{1664};
t3136 = ct{1665};
t3138 = ct{1666};
t3139 = ct{1667};
t314 = ct{1668};
t3140 = ct{1669};
t3141 = ct{1670};
t3142 = ct{1671};
t3143 = ct{1672};
t3144 = ct{1673};
t3146 = ct{1674};
t3148 = ct{1675};
t3149 = ct{1676};
t315 = ct{1677};
t3150 = ct{1678};
t3152 = ct{1679};
t3153 = ct{1680};
t3154 = ct{1681};
t3156 = ct{1682};
t3157 = ct{1683};
t3158 = ct{1684};
t316 = ct{1685};
t3160 = ct{1686};
t3163 = ct{1687};
t3167 = ct{1688};
t3169 = ct{1689};
t3170 = ct{1690};
t3171 = ct{1691};
t3172 = ct{1692};
t3174 = ct{1693};
t3175 = ct{1694};
t3176 = ct{1695};
t3178 = ct{1696};
t3179 = ct{1697};
t318 = ct{1698};
t3180 = ct{1699};
t3182 = ct{1700};
t3183 = ct{1701};
t3184 = ct{1702};
t3185 = ct{1703};
t3186 = ct{1704};
t3187 = ct{1705};
t3188 = ct{1706};
t3189 = ct{1707};
t319 = ct{1708};
t3190 = ct{1709};
t3191 = ct{1710};
t3192 = ct{1711};
t3193 = ct{1712};
t3194 = ct{1713};
t3195 = ct{1714};
t3196 = ct{1715};
t3198 = ct{1716};
t3199 = ct{1717};
t320 = ct{1718};
t3200 = ct{1719};
t3201 = ct{1720};
t3202 = ct{1721};
t3203 = ct{1722};
t3204 = ct{1723};
t3205 = ct{1724};
t3207 = ct{1725};
t3208 = ct{1726};
t3209 = ct{1727};
t3210 = ct{1728};
t3213 = ct{1729};
t3214 = ct{1730};
t3215 = ct{1731};
t3216 = ct{1732};
t3217 = ct{1733};
t3219 = ct{1734};
t322 = ct{1735};
t3226 = ct{1736};
t3227 = ct{1737};
t3228 = ct{1738};
t3229 = ct{1739};
t3230 = ct{1740};
t3232 = ct{1741};
t3234 = ct{1742};
t3235 = ct{1743};
t3236 = ct{1744};
t324 = ct{1745};
t3240 = ct{1746};
t3242 = ct{1747};
t3243 = ct{1748};
t3245 = ct{1749};
t3247 = ct{1750};
t3249 = ct{1751};
t325 = ct{1752};
t3250 = ct{1753};
t3251 = ct{1754};
t3252 = ct{1755};
t3254 = ct{1756};
t3256 = ct{1757};
t3257 = ct{1758};
t3265 = ct{1759};
t3267 = ct{1760};
t3269 = ct{1761};
t3270 = ct{1762};
t3271 = ct{1763};
t3272 = ct{1764};
t3273 = ct{1765};
t3274 = ct{1766};
t3275 = ct{1767};
t3276 = ct{1768};
t3277 = ct{1769};
t3278 = ct{1770};
t3279 = ct{1771};
t328 = ct{1772};
t3280 = ct{1773};
t3282 = ct{1774};
t3283 = ct{1775};
t3284 = ct{1776};
t3285 = ct{1777};
t3286 = ct{1778};
t3287 = ct{1779};
t3288 = ct{1780};
t3289 = ct{1781};
t3290 = ct{1782};
t3291 = ct{1783};
t3292 = ct{1784};
t3293 = ct{1785};
t3295 = ct{1786};
t3296 = ct{1787};
t3297 = ct{1788};
t3298 = ct{1789};
t3299 = ct{1790};
t3301 = ct{1791};
t3302 = ct{1792};
t3303 = ct{1793};
t3306 = ct{1794};
t3307 = ct{1795};
t3308 = ct{1796};
t3309 = ct{1797};
t3310 = ct{1798};
t3312 = ct{1799};
t3313 = ct{1800};
t3314 = ct{1801};
t3317 = ct{1802};
t3318 = ct{1803};
t3320 = ct{1804};
t3321 = ct{1805};
t3322 = ct{1806};
t3323 = ct{1807};
t3324 = ct{1808};
t3325 = ct{1809};
t3326 = ct{1810};
t3327 = ct{1811};
t3328 = ct{1812};
t3329 = ct{1813};
t333 = ct{1814};
t3331 = ct{1815};
t3332 = ct{1816};
t3333 = ct{1817};
t3334 = ct{1818};
t3335 = ct{1819};
t3336 = ct{1820};
t3337 = ct{1821};
t3338 = ct{1822};
t3339 = ct{1823};
t3340 = ct{1824};
t3341 = ct{1825};
t3342 = ct{1826};
t3343 = ct{1827};
t3346 = ct{1828};
t3347 = ct{1829};
t3349 = ct{1830};
t3350 = ct{1831};
t3351 = ct{1832};
t3352 = ct{1833};
t3353 = ct{1834};
t3354 = ct{1835};
t3356 = ct{1836};
t3357 = ct{1837};
t3358 = ct{1838};
t3359 = ct{1839};
t336 = ct{1840};
t3360 = ct{1841};
t3362 = ct{1842};
t3363 = ct{1843};
t3364 = ct{1844};
t3365 = ct{1845};
t3366 = ct{1846};
t3367 = ct{1847};
t3368 = ct{1848};
t3369 = ct{1849};
t337 = ct{1850};
t3371 = ct{1851};
t3372 = ct{1852};
t3373 = ct{1853};
t3374 = ct{1854};
t3375 = ct{1855};
t3376 = ct{1856};
t3377 = ct{1857};
t3378 = ct{1858};
t3380 = ct{1859};
t3381 = ct{1860};
t3382 = ct{1861};
t3383 = ct{1862};
t3384 = ct{1863};
t3386 = ct{1864};
t3387 = ct{1865};
t3388 = ct{1866};
t3390 = ct{1867};
t3391 = ct{1868};
t3392 = ct{1869};
t3393 = ct{1870};
t3394 = ct{1871};
t3395 = ct{1872};
t3396 = ct{1873};
t3397 = ct{1874};
t3398 = ct{1875};
t3399 = ct{1876};
t34 = ct{1877};
t340 = ct{1878};
t3400 = ct{1879};
t3402 = ct{1880};
t3403 = ct{1881};
t3404 = ct{1882};
t3405 = ct{1883};
t3407 = ct{1884};
t3408 = ct{1885};
t3409 = ct{1886};
t3410 = ct{1887};
t3411 = ct{1888};
t3412 = ct{1889};
t3413 = ct{1890};
t3416 = ct{1891};
t3417 = ct{1892};
t3418 = ct{1893};
t3420 = ct{1894};
t3421 = ct{1895};
t3422 = ct{1896};
t3423 = ct{1897};
t3424 = ct{1898};
t3425 = ct{1899};
t3426 = ct{1900};
t3427 = ct{1901};
t3429 = ct{1902};
t3430 = ct{1903};
t3431 = ct{1904};
t3432 = ct{1905};
t3433 = ct{1906};
t3434 = ct{1907};
t3435 = ct{1908};
t3436 = ct{1909};
t3437 = ct{1910};
t3439 = ct{1911};
t344 = ct{1912};
t3440 = ct{1913};
t3441 = ct{1914};
t3442 = ct{1915};
t3443 = ct{1916};
t3444 = ct{1917};
t3445 = ct{1918};
t3446 = ct{1919};
t3447 = ct{1920};
t3448 = ct{1921};
t3449 = ct{1922};
t3450 = ct{1923};
t3453 = ct{1924};
t3454 = ct{1925};
t3455 = ct{1926};
t3456 = ct{1927};
t3457 = ct{1928};
t3458 = ct{1929};
t346 = ct{1930};
t3460 = ct{1931};
t3461 = ct{1932};
t3462 = ct{1933};
t3463 = ct{1934};
t3464 = ct{1935};
t3465 = ct{1936};
t3466 = ct{1937};
t3467 = ct{1938};
t3468 = ct{1939};
t3469 = ct{1940};
t347 = ct{1941};
t3470 = ct{1942};
t3471 = ct{1943};
t3472 = ct{1944};
t3473 = ct{1945};
t3474 = ct{1946};
t3475 = ct{1947};
t3476 = ct{1948};
t3479 = ct{1949};
t348 = ct{1950};
t3480 = ct{1951};
t3481 = ct{1952};
t3483 = ct{1953};
t3484 = ct{1954};
t3485 = ct{1955};
t3487 = ct{1956};
t3488 = ct{1957};
t3489 = ct{1958};
t349 = ct{1959};
t3490 = ct{1960};
t3491 = ct{1961};
t3492 = ct{1962};
t3493 = ct{1963};
t3494 = ct{1964};
t3496 = ct{1965};
t3497 = ct{1966};
t3498 = ct{1967};
t3499 = ct{1968};
t350 = ct{1969};
t3500 = ct{1970};
t3501 = ct{1971};
t3502 = ct{1972};
t3503 = ct{1973};
t3504 = ct{1974};
t3505 = ct{1975};
t3506 = ct{1976};
t3507 = ct{1977};
t3509 = ct{1978};
t3510 = ct{1979};
t3511 = ct{1980};
t3513 = ct{1981};
t3514 = ct{1982};
t3515 = ct{1983};
t3516 = ct{1984};
t3517 = ct{1985};
t3518 = ct{1986};
t352 = ct{1987};
t3521 = ct{1988};
t3522 = ct{1989};
t3523 = ct{1990};
t3526 = ct{1991};
t3529 = ct{1992};
t353 = ct{1993};
t3530 = ct{1994};
t3531 = ct{1995};
t3532 = ct{1996};
t3533 = ct{1997};
t3535 = ct{1998};
t3536 = ct{1999};
t3538 = ct{2000};
t3539 = ct{2001};
t3540 = ct{2002};
t3542 = ct{2003};
t3543 = ct{2004};
t3544 = ct{2005};
t3546 = ct{2006};
t3547 = ct{2007};
t3549 = ct{2008};
t3551 = ct{2009};
t3552 = ct{2010};
t3554 = ct{2011};
t3556 = ct{2012};
t3557 = ct{2013};
t3559 = ct{2014};
t356 = ct{2015};
t3560 = ct{2016};
t3561 = ct{2017};
t3562 = ct{2018};
t3563 = ct{2019};
t3564 = ct{2020};
t3565 = ct{2021};
t3566 = ct{2022};
t3568 = ct{2023};
t3569 = ct{2024};
t357 = ct{2025};
t3570 = ct{2026};
t3571 = ct{2027};
t3572 = ct{2028};
t3573 = ct{2029};
t3574 = ct{2030};
t3577 = ct{2031};
t3578 = ct{2032};
t358 = ct{2033};
t3582 = ct{2034};
t3583 = ct{2035};
t3584 = ct{2036};
t3585 = ct{2037};
t3586 = ct{2038};
t3587 = ct{2039};
t3588 = ct{2040};
t3589 = ct{2041};
t359 = ct{2042};
t3590 = ct{2043};
t3592 = ct{2044};
t3593 = ct{2045};
t3594 = ct{2046};
t3595 = ct{2047};
t3596 = ct{2048};
t3597 = ct{2049};
t3598 = ct{2050};
t3599 = ct{2051};
t3600 = ct{2052};
t3602 = ct{2053};
t3603 = ct{2054};
t3604 = ct{2055};
t3605 = ct{2056};
t3606 = ct{2057};
t3607 = ct{2058};
t3609 = ct{2059};
t361 = ct{2060};
t3610 = ct{2061};
t3611 = ct{2062};
t3612 = ct{2063};
t3616 = ct{2064};
t3617 = ct{2065};
t3618 = ct{2066};
t362 = ct{2067};
t3623 = ct{2068};
t3624 = ct{2069};
t3625 = ct{2070};
t3626 = ct{2071};
t3630 = ct{2072};
t3631 = ct{2073};
t3632 = ct{2074};
t3633 = ct{2075};
t3634 = ct{2076};
t3635 = ct{2077};
t3636 = ct{2078};
t3637 = ct{2079};
t3638 = ct{2080};
t3640 = ct{2081};
t3642 = ct{2082};
t3644 = ct{2083};
t3648 = ct{2084};
t365 = ct{2085};
t3652 = ct{2086};
t3653 = ct{2087};
t3654 = ct{2088};
t3655 = ct{2089};
t3656 = ct{2090};
t3657 = ct{2091};
t3658 = ct{2092};
t3659 = ct{2093};
t3660 = ct{2094};
t3662 = ct{2095};
t3663 = ct{2096};
t3664 = ct{2097};
t3666 = ct{2098};
t3667 = ct{2099};
t3668 = ct{2100};
t3669 = ct{2101};
t3670 = ct{2102};
t3671 = ct{2103};
t3674 = ct{2104};
t3676 = ct{2105};
t3677 = ct{2106};
t3678 = ct{2107};
t3679 = ct{2108};
t368 = ct{2109};
t3681 = ct{2110};
t3682 = ct{2111};
t3685 = ct{2112};
t3687 = ct{2113};
t369 = ct{2114};
t3690 = ct{2115};
t3691 = ct{2116};
t3692 = ct{2117};
t3693 = ct{2118};
t3694 = ct{2119};
t3695 = ct{2120};
t3696 = ct{2121};
t3697 = ct{2122};
t3698 = ct{2123};
t3699 = ct{2124};
t3700 = ct{2125};
t3701 = ct{2126};
t3702 = ct{2127};
t3703 = ct{2128};
t3704 = ct{2129};
t3705 = ct{2130};
t3706 = ct{2131};
t3707 = ct{2132};
t3708 = ct{2133};
t3709 = ct{2134};
t371 = ct{2135};
t3711 = ct{2136};
t3712 = ct{2137};
t3713 = ct{2138};
t3715 = ct{2139};
t3716 = ct{2140};
t3717 = ct{2141};
t3718 = ct{2142};
t3719 = ct{2143};
t372 = ct{2144};
t3720 = ct{2145};
t3724 = ct{2146};
t3725 = ct{2147};
t3726 = ct{2148};
t3727 = ct{2149};
t3728 = ct{2150};
t3729 = ct{2151};
t373 = ct{2152};
t3730 = ct{2153};
t3731 = ct{2154};
t3732 = ct{2155};
t3733 = ct{2156};
t3734 = ct{2157};
t3735 = ct{2158};
t3736 = ct{2159};
t3737 = ct{2160};
t3738 = ct{2161};
t3739 = ct{2162};
t374 = ct{2163};
t3740 = ct{2164};
t3741 = ct{2165};
t3742 = ct{2166};
t3743 = ct{2167};
t3744 = ct{2168};
t3745 = ct{2169};
t3746 = ct{2170};
t3747 = ct{2171};
t3750 = ct{2172};
t3752 = ct{2173};
t3753 = ct{2174};
t3754 = ct{2175};
t3755 = ct{2176};
t3756 = ct{2177};
t3757 = ct{2178};
t3758 = ct{2179};
t3759 = ct{2180};
t3760 = ct{2181};
t3761 = ct{2182};
t3762 = ct{2183};
t3763 = ct{2184};
t3766 = ct{2185};
t3768 = ct{2186};
t3769 = ct{2187};
t377 = ct{2188};
t3772 = ct{2189};
t3774 = ct{2190};
t3775 = ct{2191};
t3777 = ct{2192};
t3778 = ct{2193};
t3779 = ct{2194};
t378 = ct{2195};
t3780 = ct{2196};
t3781 = ct{2197};
t3782 = ct{2198};
t3783 = ct{2199};
t3784 = ct{2200};
t3785 = ct{2201};
t3786 = ct{2202};
t3787 = ct{2203};
t3788 = ct{2204};
t3789 = ct{2205};
t379 = ct{2206};
t3790 = ct{2207};
t3791 = ct{2208};
t3792 = ct{2209};
t3793 = ct{2210};
t3794 = ct{2211};
t3795 = ct{2212};
t3796 = ct{2213};
t3797 = ct{2214};
t3798 = ct{2215};
t380 = ct{2216};
t3800 = ct{2217};
t3801 = ct{2218};
t3802 = ct{2219};
t3810 = ct{2220};
t3811 = ct{2221};
t3812 = ct{2222};
t3813 = ct{2223};
t3814 = ct{2224};
t3815 = ct{2225};
t3816 = ct{2226};
t3817 = ct{2227};
t3818 = ct{2228};
t3819 = ct{2229};
t382 = ct{2230};
t3820 = ct{2231};
t3821 = ct{2232};
t3822 = ct{2233};
t3823 = ct{2234};
t3824 = ct{2235};
t3825 = ct{2236};
t3826 = ct{2237};
t3827 = ct{2238};
t3828 = ct{2239};
t3831 = ct{2240};
t3833 = ct{2241};
t3834 = ct{2242};
t3835 = ct{2243};
t3836 = ct{2244};
t3837 = ct{2245};
t3839 = ct{2246};
t384 = ct{2247};
t3840 = ct{2248};
t3843 = ct{2249};
t3845 = ct{2250};
t3849 = ct{2251};
t3850 = ct{2252};
t3851 = ct{2253};
t3852 = ct{2254};
t3853 = ct{2255};
t3855 = ct{2256};
t3856 = ct{2257};
t386 = ct{2258};
t3860 = ct{2259};
t3861 = ct{2260};
t3862 = ct{2261};
t3863 = ct{2262};
t3865 = ct{2263};
t3866 = ct{2264};
t3867 = ct{2265};
t3868 = ct{2266};
t3869 = ct{2267};
t387 = ct{2268};
t3870 = ct{2269};
t3871 = ct{2270};
t3872 = ct{2271};
t3873 = ct{2272};
t3875 = ct{2273};
t3877 = ct{2274};
t388 = ct{2275};
t3881 = ct{2276};
t3882 = ct{2277};
t3883 = ct{2278};
t3884 = ct{2279};
t3885 = ct{2280};
t3886 = ct{2281};
t3887 = ct{2282};
t3888 = ct{2283};
t3889 = ct{2284};
t3890 = ct{2285};
t3891 = ct{2286};
t3892 = ct{2287};
t3893 = ct{2288};
t3894 = ct{2289};
t3895 = ct{2290};
t3897 = ct{2291};
t3899 = ct{2292};
t3901 = ct{2293};
t3902 = ct{2294};
t3903 = ct{2295};
t3908 = ct{2296};
t391 = ct{2297};
t3910 = ct{2298};
t3911 = ct{2299};
t3912 = ct{2300};
t3913 = ct{2301};
t3914 = ct{2302};
t3915 = ct{2303};
t3916 = ct{2304};
t3917 = ct{2305};
t3918 = ct{2306};
t392 = ct{2307};
t3921 = ct{2308};
t3922 = ct{2309};
t3929 = ct{2310};
t3930 = ct{2311};
t3941 = ct{2312};
t3946 = ct{2313};
t3949 = ct{2314};
t395 = ct{2315};
t3950 = ct{2316};
t3951 = ct{2317};
t3952 = ct{2318};
t3953 = ct{2319};
t3958 = ct{2320};
t3959 = ct{2321};
t396 = ct{2322};
t3966 = ct{2323};
t3970 = ct{2324};
t3980 = ct{2325};
t3981 = ct{2326};
t3982 = ct{2327};
t3984 = ct{2328};
t3990 = ct{2329};
t4 = ct{2330};
t400 = ct{2331};
t4004 = ct{2332};
t4005 = ct{2333};
t4006 = ct{2334};
t401 = ct{2335};
t4010 = ct{2336};
t4011 = ct{2337};
t4014 = ct{2338};
t4015 = ct{2339};
t4016 = ct{2340};
t4017 = ct{2341};
t4018 = ct{2342};
t4019 = ct{2343};
t402 = ct{2344};
t4020 = ct{2345};
t4021 = ct{2346};
t4022 = ct{2347};
t4023 = ct{2348};
t4024 = ct{2349};
t4025 = ct{2350};
t4026 = ct{2351};
t4027 = ct{2352};
t4028 = ct{2353};
t4029 = ct{2354};
t403 = ct{2355};
t4036 = ct{2356};
t4039 = ct{2357};
t4040 = ct{2358};
t4041 = ct{2359};
t4042 = ct{2360};
t4045 = ct{2361};
t4046 = ct{2362};
t4047 = ct{2363};
t4048 = ct{2364};
t4051 = ct{2365};
t4053 = ct{2366};
t4054 = ct{2367};
t406 = ct{2368};
t4062 = ct{2369};
t4063 = ct{2370};
t4064 = ct{2371};
t4065 = ct{2372};
t4068 = ct{2373};
t4069 = ct{2374};
t4070 = ct{2375};
t4071 = ct{2376};
t4073 = ct{2377};
t4074 = ct{2378};
t4075 = ct{2379};
t4089 = ct{2380};
t4099 = ct{2381};
t410 = ct{2382};
t4103 = ct{2383};
t4105 = ct{2384};
t411 = ct{2385};
t4113 = ct{2386};
t4114 = ct{2387};
t4116 = ct{2388};
t4118 = ct{2389};
t4119 = ct{2390};
t412 = ct{2391};
t4123 = ct{2392};
t4124 = ct{2393};
t4125 = ct{2394};
t413 = ct{2395};
t4132 = ct{2396};
t414 = ct{2397};
t4140 = ct{2398};
t4142 = ct{2399};
t4143 = ct{2400};
t4144 = ct{2401};
t4145 = ct{2402};
t415 = ct{2403};
t4150 = ct{2404};
t4152 = ct{2405};
t4153 = ct{2406};
t416 = ct{2407};
t4162 = ct{2408};
t4164 = ct{2409};
t4165 = ct{2410};
t4166 = ct{2411};
t4169 = ct{2412};
t417 = ct{2413};
t4171 = ct{2414};
t4173 = ct{2415};
t4174 = ct{2416};
t4177 = ct{2417};
t4178 = ct{2418};
t4179 = ct{2419};
t418 = ct{2420};
t4180 = ct{2421};
t4181 = ct{2422};
t4183 = ct{2423};
t4184 = ct{2424};
t4185 = ct{2425};
t4186 = ct{2426};
t4188 = ct{2427};
t4190 = ct{2428};
t4195 = ct{2429};
t4196 = ct{2430};
t4197 = ct{2431};
t420 = ct{2432};
t4201 = ct{2433};
t4202 = ct{2434};
t4205 = ct{2435};
t4206 = ct{2436};
t4207 = ct{2437};
t4208 = ct{2438};
t4209 = ct{2439};
t4210 = ct{2440};
t4211 = ct{2441};
t4215 = ct{2442};
t4217 = ct{2443};
t4218 = ct{2444};
t4219 = ct{2445};
t422 = ct{2446};
t4220 = ct{2447};
t4221 = ct{2448};
t4223 = ct{2449};
t4224 = ct{2450};
t4225 = ct{2451};
t4226 = ct{2452};
t4228 = ct{2453};
t4229 = ct{2454};
t423 = ct{2455};
t4230 = ct{2456};
t4231 = ct{2457};
t4232 = ct{2458};
t4233 = ct{2459};
t4234 = ct{2460};
t4235 = ct{2461};
t424 = ct{2462};
t4241 = ct{2463};
t4242 = ct{2464};
t4243 = ct{2465};
t4244 = ct{2466};
t4245 = ct{2467};
t4246 = ct{2468};
t4247 = ct{2469};
t4248 = ct{2470};
t4249 = ct{2471};
t425 = ct{2472};
t4250 = ct{2473};
t4251 = ct{2474};
t4253 = ct{2475};
t4254 = ct{2476};
t4255 = ct{2477};
t4256 = ct{2478};
t4257 = ct{2479};
t4258 = ct{2480};
t4259 = ct{2481};
t4260 = ct{2482};
t4261 = ct{2483};
t4262 = ct{2484};
t4263 = ct{2485};
t427 = ct{2486};
t4273 = ct{2487};
t4274 = ct{2488};
t4275 = ct{2489};
t4276 = ct{2490};
t4278 = ct{2491};
t4279 = ct{2492};
t428 = ct{2493};
t4280 = ct{2494};
t4281 = ct{2495};
t4282 = ct{2496};
t4283 = ct{2497};
t4284 = ct{2498};
t4285 = ct{2499};
t4286 = ct{2500};
t4287 = ct{2501};
t4289 = ct{2502};
t429 = ct{2503};
t4290 = ct{2504};
t4291 = ct{2505};
t4292 = ct{2506};
t4293 = ct{2507};
t4295 = ct{2508};
t4296 = ct{2509};
t4297 = ct{2510};
t4298 = ct{2511};
t4299 = ct{2512};
t4300 = ct{2513};
t4301 = ct{2514};
t4302 = ct{2515};
t4303 = ct{2516};
t4304 = ct{2517};
t4305 = ct{2518};
t4306 = ct{2519};
t4308 = ct{2520};
t431 = ct{2521};
t4310 = ct{2522};
t4315 = ct{2523};
t4316 = ct{2524};
t4317 = ct{2525};
t4318 = ct{2526};
t432 = ct{2527};
t4321 = ct{2528};
t4323 = ct{2529};
t4324 = ct{2530};
t4325 = ct{2531};
t4326 = ct{2532};
t4327 = ct{2533};
t4328 = ct{2534};
t4329 = ct{2535};
t433 = ct{2536};
t4330 = ct{2537};
t4331 = ct{2538};
t4332 = ct{2539};
t4333 = ct{2540};
t4334 = ct{2541};
t4335 = ct{2542};
t4336 = ct{2543};
t4337 = ct{2544};
t4338 = ct{2545};
t4339 = ct{2546};
t434 = ct{2547};
t4340 = ct{2548};
t4342 = ct{2549};
t4344 = ct{2550};
t4345 = ct{2551};
t4346 = ct{2552};
t4347 = ct{2553};
t4348 = ct{2554};
t4349 = ct{2555};
t435 = ct{2556};
t4350 = ct{2557};
t4354 = ct{2558};
t4356 = ct{2559};
t4357 = ct{2560};
t436 = ct{2561};
t4362 = ct{2562};
t4363 = ct{2563};
t4365 = ct{2564};
t4366 = ct{2565};
t4368 = ct{2566};
t4369 = ct{2567};
t437 = ct{2568};
t4370 = ct{2569};
t4371 = ct{2570};
t4372 = ct{2571};
t4373 = ct{2572};
t4374 = ct{2573};
t4375 = ct{2574};
t4376 = ct{2575};
t4377 = ct{2576};
t4379 = ct{2577};
t438 = ct{2578};
t4380 = ct{2579};
t4382 = ct{2580};
t4383 = ct{2581};
t4384 = ct{2582};
t4385 = ct{2583};
t4386 = ct{2584};
t4387 = ct{2585};
t4388 = ct{2586};
t4389 = ct{2587};
t439 = ct{2588};
t4391 = ct{2589};
t4392 = ct{2590};
t4394 = ct{2591};
t4395 = ct{2592};
t4396 = ct{2593};
t4397 = ct{2594};
t4398 = ct{2595};
t4399 = ct{2596};
t44 = ct{2597};
t440 = ct{2598};
t4400 = ct{2599};
t4401 = ct{2600};
t4402 = ct{2601};
t4403 = ct{2602};
t4404 = ct{2603};
t4405 = ct{2604};
t4406 = ct{2605};
t4407 = ct{2606};
t4408 = ct{2607};
t4409 = ct{2608};
t441 = ct{2609};
t4410 = ct{2610};
t4411 = ct{2611};
t4412 = ct{2612};
t4413 = ct{2613};
t4414 = ct{2614};
t4415 = ct{2615};
t4416 = ct{2616};
t4417 = ct{2617};
t4418 = ct{2618};
t4419 = ct{2619};
t442 = ct{2620};
t4420 = ct{2621};
t4421 = ct{2622};
t4422 = ct{2623};
t4423 = ct{2624};
t4424 = ct{2625};
t4425 = ct{2626};
t4426 = ct{2627};
t4427 = ct{2628};
t4428 = ct{2629};
t4429 = ct{2630};
t4430 = ct{2631};
t4431 = ct{2632};
t4432 = ct{2633};
t4433 = ct{2634};
t4434 = ct{2635};
t4435 = ct{2636};
t4436 = ct{2637};
t4437 = ct{2638};
t4438 = ct{2639};
t4439 = ct{2640};
t444 = ct{2641};
t4440 = ct{2642};
t4442 = ct{2643};
t4444 = ct{2644};
t4445 = ct{2645};
t4446 = ct{2646};
t4447 = ct{2647};
t4448 = ct{2648};
t4449 = ct{2649};
t445 = ct{2650};
t4450 = ct{2651};
t4451 = ct{2652};
t4453 = ct{2653};
t4454 = ct{2654};
t4455 = ct{2655};
t4460 = ct{2656};
t4461 = ct{2657};
t4462 = ct{2658};
t4463 = ct{2659};
t4464 = ct{2660};
t4465 = ct{2661};
t4466 = ct{2662};
t4467 = ct{2663};
t4468 = ct{2664};
t4469 = ct{2665};
t4470 = ct{2666};
t4471 = ct{2667};
t4473 = ct{2668};
t4474 = ct{2669};
t4475 = ct{2670};
t4476 = ct{2671};
t4477 = ct{2672};
t4478 = ct{2673};
t4479 = ct{2674};
t448 = ct{2675};
t4481 = ct{2676};
t4482 = ct{2677};
t4483 = ct{2678};
t4484 = ct{2679};
t4485 = ct{2680};
t4486 = ct{2681};
t4487 = ct{2682};
t4488 = ct{2683};
t4489 = ct{2684};
t449 = ct{2685};
t4490 = ct{2686};
t4493 = ct{2687};
t4494 = ct{2688};
t4495 = ct{2689};
t4496 = ct{2690};
t4497 = ct{2691};
t4498 = ct{2692};
t4499 = ct{2693};
t45 = ct{2694};
t450 = ct{2695};
t4500 = ct{2696};
t4501 = ct{2697};
t4502 = ct{2698};
t4503 = ct{2699};
t4504 = ct{2700};
t4505 = ct{2701};
t4506 = ct{2702};
t4507 = ct{2703};
t4508 = ct{2704};
t4509 = ct{2705};
t4510 = ct{2706};
t4512 = ct{2707};
t4513 = ct{2708};
t4514 = ct{2709};
t4515 = ct{2710};
t4516 = ct{2711};
t4518 = ct{2712};
t4519 = ct{2713};
t452 = ct{2714};
t4520 = ct{2715};
t4521 = ct{2716};
t4522 = ct{2717};
t4523 = ct{2718};
t4524 = ct{2719};
t4525 = ct{2720};
t4526 = ct{2721};
t4527 = ct{2722};
t4529 = ct{2723};
t453 = ct{2724};
t4530 = ct{2725};
t4531 = ct{2726};
t4532 = ct{2727};
t4534 = ct{2728};
t4535 = ct{2729};
t4537 = ct{2730};
t4538 = ct{2731};
t4539 = ct{2732};
t454 = ct{2733};
t4541 = ct{2734};
t4543 = ct{2735};
t4544 = ct{2736};
t4545 = ct{2737};
t4546 = ct{2738};
t4547 = ct{2739};
t4549 = ct{2740};
t4550 = ct{2741};
t4551 = ct{2742};
t4552 = ct{2743};
t4553 = ct{2744};
t4554 = ct{2745};
t4556 = ct{2746};
t4557 = ct{2747};
t4558 = ct{2748};
t4559 = ct{2749};
t4560 = ct{2750};
t4564 = ct{2751};
t4565 = ct{2752};
t4566 = ct{2753};
t4567 = ct{2754};
t4568 = ct{2755};
t4569 = ct{2756};
t457 = ct{2757};
t4570 = ct{2758};
t4572 = ct{2759};
t4573 = ct{2760};
t4575 = ct{2761};
t4576 = ct{2762};
t4577 = ct{2763};
t4578 = ct{2764};
t458 = ct{2765};
t4580 = ct{2766};
t4581 = ct{2767};
t4582 = ct{2768};
t4584 = ct{2769};
t4586 = ct{2770};
t4587 = ct{2771};
t4588 = ct{2772};
t4589 = ct{2773};
t459 = ct{2774};
t4590 = ct{2775};
t4591 = ct{2776};
t4592 = ct{2777};
t4593 = ct{2778};
t4594 = ct{2779};
t4595 = ct{2780};
t4596 = ct{2781};
t4597 = ct{2782};
t4598 = ct{2783};
t4599 = ct{2784};
t46 = ct{2785};
t460 = ct{2786};
t4600 = ct{2787};
t4601 = ct{2788};
t4602 = ct{2789};
t4603 = ct{2790};
t4604 = ct{2791};
t4605 = ct{2792};
t4606 = ct{2793};
t4607 = ct{2794};
t4608 = ct{2795};
t4609 = ct{2796};
t461 = ct{2797};
t4610 = ct{2798};
t4612 = ct{2799};
t4613 = ct{2800};
t4614 = ct{2801};
t4615 = ct{2802};
t4616 = ct{2803};
t4617 = ct{2804};
t4618 = ct{2805};
t4619 = ct{2806};
t462 = ct{2807};
t4620 = ct{2808};
t4621 = ct{2809};
t4622 = ct{2810};
t4623 = ct{2811};
t4624 = ct{2812};
t4625 = ct{2813};
t4626 = ct{2814};
t4627 = ct{2815};
t4629 = ct{2816};
t463 = ct{2817};
t4631 = ct{2818};
t4632 = ct{2819};
t4633 = ct{2820};
t4634 = ct{2821};
t4635 = ct{2822};
t4636 = ct{2823};
t4637 = ct{2824};
t4638 = ct{2825};
t4639 = ct{2826};
t464 = ct{2827};
t4640 = ct{2828};
t4643 = ct{2829};
t4644 = ct{2830};
t4645 = ct{2831};
t4646 = ct{2832};
t4647 = ct{2833};
t4649 = ct{2834};
t465 = ct{2835};
t4650 = ct{2836};
t4652 = ct{2837};
t4653 = ct{2838};
t4654 = ct{2839};
t4655 = ct{2840};
t4656 = ct{2841};
t4657 = ct{2842};
t4659 = ct{2843};
t466 = ct{2844};
t4660 = ct{2845};
t4661 = ct{2846};
t4662 = ct{2847};
t4663 = ct{2848};
t4664 = ct{2849};
t4665 = ct{2850};
t4666 = ct{2851};
t4667 = ct{2852};
t4668 = ct{2853};
t4669 = ct{2854};
t4670 = ct{2855};
t4671 = ct{2856};
t4672 = ct{2857};
t4673 = ct{2858};
t4674 = ct{2859};
t4675 = ct{2860};
t4676 = ct{2861};
t4677 = ct{2862};
t4678 = ct{2863};
t4679 = ct{2864};
t468 = ct{2865};
t4680 = ct{2866};
t4681 = ct{2867};
t4682 = ct{2868};
t4683 = ct{2869};
t4684 = ct{2870};
t4685 = ct{2871};
t4686 = ct{2872};
t4687 = ct{2873};
t4689 = ct{2874};
t469 = ct{2875};
t4692 = ct{2876};
t4693 = ct{2877};
t4694 = ct{2878};
t4695 = ct{2879};
t4696 = ct{2880};
t4697 = ct{2881};
t4698 = ct{2882};
t4699 = ct{2883};
t47 = ct{2884};
t470 = ct{2885};
t4700 = ct{2886};
t4702 = ct{2887};
t4703 = ct{2888};
t4704 = ct{2889};
t4707 = ct{2890};
t4708 = ct{2891};
t4709 = ct{2892};
t471 = ct{2893};
t4710 = ct{2894};
t4711 = ct{2895};
t4712 = ct{2896};
t4713 = ct{2897};
t4714 = ct{2898};
t4715 = ct{2899};
t4716 = ct{2900};
t4717 = ct{2901};
t4718 = ct{2902};
t4719 = ct{2903};
t472 = ct{2904};
t4720 = ct{2905};
t4721 = ct{2906};
t4722 = ct{2907};
t4723 = ct{2908};
t4724 = ct{2909};
t4725 = ct{2910};
t4726 = ct{2911};
t4727 = ct{2912};
t4728 = ct{2913};
t4729 = ct{2914};
t4730 = ct{2915};
t4731 = ct{2916};
t4732 = ct{2917};
t4733 = ct{2918};
t4734 = ct{2919};
t4736 = ct{2920};
t4737 = ct{2921};
t4738 = ct{2922};
t4739 = ct{2923};
t4740 = ct{2924};
t4742 = ct{2925};
t4745 = ct{2926};
t4746 = ct{2927};
t4747 = ct{2928};
t4748 = ct{2929};
t475 = ct{2930};
t4750 = ct{2931};
t4751 = ct{2932};
t4753 = ct{2933};
t4754 = ct{2934};
t4755 = ct{2935};
t4756 = ct{2936};
t4757 = ct{2937};
t4762 = ct{2938};
t4763 = ct{2939};
t4765 = ct{2940};
t4768 = ct{2941};
t477 = ct{2942};
t4771 = ct{2943};
t4772 = ct{2944};
t4773 = ct{2945};
t4774 = ct{2946};
t4775 = ct{2947};
t4776 = ct{2948};
t4779 = ct{2949};
t4780 = ct{2950};
t4781 = ct{2951};
t4782 = ct{2952};
t4783 = ct{2953};
t4784 = ct{2954};
t4785 = ct{2955};
t4786 = ct{2956};
t4787 = ct{2957};
t4788 = ct{2958};
t4789 = ct{2959};
t479 = ct{2960};
t4790 = ct{2961};
t4791 = ct{2962};
t4792 = ct{2963};
t4793 = ct{2964};
t4794 = ct{2965};
t4795 = ct{2966};
t4797 = ct{2967};
t4799 = ct{2968};
t480 = ct{2969};
t4800 = ct{2970};
t4801 = ct{2971};
t4802 = ct{2972};
t4803 = ct{2973};
t4805 = ct{2974};
t4806 = ct{2975};
t4809 = ct{2976};
t481 = ct{2977};
t4810 = ct{2978};
t4811 = ct{2979};
t4812 = ct{2980};
t4813 = ct{2981};
t4814 = ct{2982};
t4818 = ct{2983};
t4819 = ct{2984};
t482 = ct{2985};
t4820 = ct{2986};
t4821 = ct{2987};
t4824 = ct{2988};
t4825 = ct{2989};
t4826 = ct{2990};
t4827 = ct{2991};
t4829 = ct{2992};
t483 = ct{2993};
t4831 = ct{2994};
t4833 = ct{2995};
t4834 = ct{2996};
t4835 = ct{2997};
t4837 = ct{2998};
t484 = ct{2999};
t4840 = ct{3000};
t4841 = ct{3001};
t4842 = ct{3002};
t4845 = ct{3003};
t4846 = ct{3004};
t4847 = ct{3005};
t4848 = ct{3006};
t485 = ct{3007};
t4851 = ct{3008};
t4853 = ct{3009};
t4856 = ct{3010};
t4857 = ct{3011};
t486 = ct{3012};
t4862 = ct{3013};
t4863 = ct{3014};
t4864 = ct{3015};
t4865 = ct{3016};
t4866 = ct{3017};
t4867 = ct{3018};
t4868 = ct{3019};
t4869 = ct{3020};
t4870 = ct{3021};
t4872 = ct{3022};
t4873 = ct{3023};
t4874 = ct{3024};
t4875 = ct{3025};
t4876 = ct{3026};
t4877 = ct{3027};
t488 = ct{3028};
t4880 = ct{3029};
t4884 = ct{3030};
t4888 = ct{3031};
t489 = ct{3032};
t4893 = ct{3033};
t4895 = ct{3034};
t4903 = ct{3035};
t4904 = ct{3036};
t4907 = ct{3037};
t4908 = ct{3038};
t491 = ct{3039};
t4911 = ct{3040};
t4913 = ct{3041};
t4914 = ct{3042};
t4919 = ct{3043};
t492 = ct{3044};
t4920 = ct{3045};
t4922 = ct{3046};
t4924 = ct{3047};
t4925 = ct{3048};
t4927 = ct{3049};
t4928 = ct{3050};
t4929 = ct{3051};
t493 = ct{3052};
t4931 = ct{3053};
t4933 = ct{3054};
t4934 = ct{3055};
t4935 = ct{3056};
t4936 = ct{3057};
t494 = ct{3058};
t4942 = ct{3059};
t4943 = ct{3060};
t4944 = ct{3061};
t4946 = ct{3062};
t4948 = ct{3063};
t4949 = ct{3064};
t4950 = ct{3065};
t4951 = ct{3066};
t4952 = ct{3067};
t4953 = ct{3068};
t4957 = ct{3069};
t496 = ct{3070};
t4963 = ct{3071};
t4964 = ct{3072};
t4969 = ct{3073};
t497 = ct{3074};
t4970 = ct{3075};
t4973 = ct{3076};
t4974 = ct{3077};
t4975 = ct{3078};
t4976 = ct{3079};
t4978 = ct{3080};
t4979 = ct{3081};
t498 = ct{3082};
t4981 = ct{3083};
t4982 = ct{3084};
t4983 = ct{3085};
t4987 = ct{3086};
t4988 = ct{3087};
t4989 = ct{3088};
t499 = ct{3089};
t4990 = ct{3090};
t4991 = ct{3091};
t4992 = ct{3092};
t4993 = ct{3093};
t4994 = ct{3094};
t4995 = ct{3095};
t4996 = ct{3096};
t5 = ct{3097};
t50 = ct{3098};
t500 = ct{3099};
t5000 = ct{3100};
t5001 = ct{3101};
t5002 = ct{3102};
t5003 = ct{3103};
t5005 = ct{3104};
t5006 = ct{3105};
t5007 = ct{3106};
t5008 = ct{3107};
t5009 = ct{3108};
t501 = ct{3109};
t5010 = ct{3110};
t5014 = ct{3111};
t5015 = ct{3112};
t5016 = ct{3113};
t5017 = ct{3114};
t5018 = ct{3115};
t5019 = ct{3116};
t502 = ct{3117};
t5020 = ct{3118};
t5021 = ct{3119};
t5022 = ct{3120};
t5023 = ct{3121};
t5024 = ct{3122};
t5026 = ct{3123};
t5027 = ct{3124};
t5029 = ct{3125};
t503 = ct{3126};
t5030 = ct{3127};
t5031 = ct{3128};
t5032 = ct{3129};
t5035 = ct{3130};
t5036 = ct{3131};
t5039 = ct{3132};
t504 = ct{3133};
t5041 = ct{3134};
t5045 = ct{3135};
t5048 = ct{3136};
t505 = ct{3137};
t5051 = ct{3138};
t5054 = ct{3139};
t5055 = ct{3140};
t5056 = ct{3141};
t5058 = ct{3142};
t5059 = ct{3143};
t506 = ct{3144};
t5061 = ct{3145};
t5063 = ct{3146};
t5064 = ct{3147};
t5065 = ct{3148};
t5066 = ct{3149};
t5067 = ct{3150};
t507 = ct{3151};
t5073 = ct{3152};
t5074 = ct{3153};
t5075 = ct{3154};
t5076 = ct{3155};
t5077 = ct{3156};
t5078 = ct{3157};
t508 = ct{3158};
t5080 = ct{3159};
t5081 = ct{3160};
t5083 = ct{3161};
t5084 = ct{3162};
t5085 = ct{3163};
t5088 = ct{3164};
t5089 = ct{3165};
t509 = ct{3166};
t5090 = ct{3167};
t5091 = ct{3168};
t5093 = ct{3169};
t5095 = ct{3170};
t5097 = ct{3171};
t5098 = ct{3172};
t5099 = ct{3173};
t510 = ct{3174};
t5100 = ct{3175};
t5101 = ct{3176};
t5102 = ct{3177};
t5107 = ct{3178};
t5109 = ct{3179};
t511 = ct{3180};
t5110 = ct{3181};
t5112 = ct{3182};
t5113 = ct{3183};
t5114 = ct{3184};
t5119 = ct{3185};
t512 = ct{3186};
t5120 = ct{3187};
t5121 = ct{3188};
t5123 = ct{3189};
t5125 = ct{3190};
t513 = ct{3191};
t5131 = ct{3192};
t5132 = ct{3193};
t5136 = ct{3194};
t5138 = ct{3195};
t5139 = ct{3196};
t514 = ct{3197};
t5140 = ct{3198};
t5143 = ct{3199};
t5146 = ct{3200};
t5147 = ct{3201};
t5148 = ct{3202};
t5150 = ct{3203};
t5151 = ct{3204};
t5152 = ct{3205};
t5153 = ct{3206};
t5154 = ct{3207};
t5157 = ct{3208};
t5158 = ct{3209};
t516 = ct{3210};
t5164 = ct{3211};
t5166 = ct{3212};
t517 = ct{3213};
t5171 = ct{3214};
t5172 = ct{3215};
t5174 = ct{3216};
t5175 = ct{3217};
t518 = ct{3218};
t5180 = ct{3219};
t5181 = ct{3220};
t5183 = ct{3221};
t5184 = ct{3222};
t5185 = ct{3223};
t5187 = ct{3224};
t5189 = ct{3225};
t5191 = ct{3226};
t5195 = ct{3227};
t5199 = ct{3228};
t520 = ct{3229};
t5200 = ct{3230};
t5201 = ct{3231};
t5202 = ct{3232};
t5203 = ct{3233};
t5204 = ct{3234};
t5205 = ct{3235};
t5206 = ct{3236};
t5207 = ct{3237};
t5209 = ct{3238};
t521 = ct{3239};
t5210 = ct{3240};
t5211 = ct{3241};
t5215 = ct{3242};
t5216 = ct{3243};
t5217 = ct{3244};
t5218 = ct{3245};
t5219 = ct{3246};
t522 = ct{3247};
t5222 = ct{3248};
t5223 = ct{3249};
t5224 = ct{3250};
t5227 = ct{3251};
t5229 = ct{3252};
t523 = ct{3253};
t5233 = ct{3254};
t5236 = ct{3255};
t5237 = ct{3256};
t5238 = ct{3257};
t5239 = ct{3258};
t524 = ct{3259};
t5240 = ct{3260};
t5242 = ct{3261};
t5244 = ct{3262};
t5247 = ct{3263};
t5248 = ct{3264};
t5249 = ct{3265};
t525 = ct{3266};
t5251 = ct{3267};
t5252 = ct{3268};
t5255 = ct{3269};
t5257 = ct{3270};
t5258 = ct{3271};
t526 = ct{3272};
t5261 = ct{3273};
t5262 = ct{3274};
t5265 = ct{3275};
t5268 = ct{3276};
t5269 = ct{3277};
t527 = ct{3278};
t5270 = ct{3279};
t5272 = ct{3280};
t5279 = ct{3281};
t528 = ct{3282};
t5280 = ct{3283};
t5285 = ct{3284};
t5288 = ct{3285};
t529 = ct{3286};
t5292 = ct{3287};
t5293 = ct{3288};
t5294 = ct{3289};
t5295 = ct{3290};
t5297 = ct{3291};
t53 = ct{3292};
t530 = ct{3293};
t5302 = ct{3294};
t5306 = ct{3295};
t531 = ct{3296};
t5318 = ct{3297};
t532 = ct{3298};
t5320 = ct{3299};
t5321 = ct{3300};
t5324 = ct{3301};
t5327 = ct{3302};
t533 = ct{3303};
t5331 = ct{3304};
t5332 = ct{3305};
t5339 = ct{3306};
t534 = ct{3307};
t5344 = ct{3308};
t5346 = ct{3309};
t5347 = ct{3310};
t5348 = ct{3311};
t5349 = ct{3312};
t535 = ct{3313};
t5351 = ct{3314};
t5355 = ct{3315};
t5356 = ct{3316};
t5358 = ct{3317};
t536 = ct{3318};
t5361 = ct{3319};
t5364 = ct{3320};
t5365 = ct{3321};
t5367 = ct{3322};
t5368 = ct{3323};
t537 = ct{3324};
t5372 = ct{3325};
t5373 = ct{3326};
t5375 = ct{3327};
t5378 = ct{3328};
t538 = ct{3329};
t5383 = ct{3330};
t5387 = ct{3331};
t5389 = ct{3332};
t539 = ct{3333};
t5390 = ct{3334};
t5391 = ct{3335};
t5392 = ct{3336};
t5393 = ct{3337};
t5394 = ct{3338};
t5395 = ct{3339};
t540 = ct{3340};
t5402 = ct{3341};
t5404 = ct{3342};
t5409 = ct{3343};
t5416 = ct{3344};
t5420 = ct{3345};
t543 = ct{3346};
t5433 = ct{3347};
t5435 = ct{3348};
t5436 = ct{3349};
t544 = ct{3350};
t5440 = ct{3351};
t5441 = ct{3352};
t5442 = ct{3353};
t5443 = ct{3354};
t5444 = ct{3355};
t5445 = ct{3356};
t5446 = ct{3357};
t5448 = ct{3358};
t545 = ct{3359};
t5450 = ct{3360};
t5451 = ct{3361};
t5453 = ct{3362};
t5454 = ct{3363};
t5457 = ct{3364};
t5459 = ct{3365};
t546 = ct{3366};
t5463 = ct{3367};
t5464 = ct{3368};
t5465 = ct{3369};
t5466 = ct{3370};
t547 = ct{3371};
t5473 = ct{3372};
t5475 = ct{3373};
t5479 = ct{3374};
t548 = ct{3375};
t5480 = ct{3376};
t5481 = ct{3377};
t5482 = ct{3378};
t5483 = ct{3379};
t5484 = ct{3380};
t5485 = ct{3381};
t5486 = ct{3382};
t5487 = ct{3383};
t5488 = ct{3384};
t5489 = ct{3385};
t549 = ct{3386};
t5490 = ct{3387};
t5491 = ct{3388};
t5492 = ct{3389};
t5493 = ct{3390};
t5494 = ct{3391};
t5496 = ct{3392};
t5498 = ct{3393};
t5499 = ct{3394};
t5501 = ct{3395};
t5507 = ct{3396};
t551 = ct{3397};
t5512 = ct{3398};
t5516 = ct{3399};
t5517 = ct{3400};
t5519 = ct{3401};
t552 = ct{3402};
t5521 = ct{3403};
t5522 = ct{3404};
t5526 = ct{3405};
t5527 = ct{3406};
t553 = ct{3407};
t5534 = ct{3408};
t554 = ct{3409};
t5540 = ct{3410};
t5546 = ct{3411};
t5549 = ct{3412};
t555 = ct{3413};
t5552 = ct{3414};
t5555 = ct{3415};
t5559 = ct{3416};
t556 = ct{3417};
t5561 = ct{3418};
t5562 = ct{3419};
t5563 = ct{3420};
t5565 = ct{3421};
t5566 = ct{3422};
t5569 = ct{3423};
t557 = ct{3424};
t5573 = ct{3425};
t5578 = ct{3426};
t558 = ct{3427};
t5580 = ct{3428};
t5581 = ct{3429};
t5583 = ct{3430};
t5584 = ct{3431};
t5589 = ct{3432};
t559 = ct{3433};
t5590 = ct{3434};
t5593 = ct{3435};
t5594 = ct{3436};
t5596 = ct{3437};
t5597 = ct{3438};
t560 = ct{3439};
t5600 = ct{3440};
t5603 = ct{3441};
t5604 = ct{3442};
t5606 = ct{3443};
t5607 = ct{3444};
t561 = ct{3445};
t5611 = ct{3446};
t5612 = ct{3447};
t5618 = ct{3448};
t562 = ct{3449};
t5629 = ct{3450};
t563 = ct{3451};
t5633 = ct{3452};
t5634 = ct{3453};
t5635 = ct{3454};
t564 = ct{3455};
t5656 = ct{3456};
t5660 = ct{3457};
t5667 = ct{3458};
t5668 = ct{3459};
t567 = ct{3460};
t5673 = ct{3461};
t5678 = ct{3462};
t568 = ct{3463};
t5688 = ct{3464};
t569 = ct{3465};
t57 = ct{3466};
t570 = ct{3467};
t571 = ct{3468};
t572 = ct{3469};
t573 = ct{3470};
t574 = ct{3471};
t5741 = ct{3472};
t5743 = ct{3473};
t576 = ct{3474};
t577 = ct{3475};
t5777 = ct{3476};
t5779 = ct{3477};
t578 = ct{3478};
t5780 = ct{3479};
t5782 = ct{3480};
t579 = ct{3481};
t58 = ct{3482};
t580 = ct{3483};
t581 = ct{3484};
t5818 = ct{3485};
t5819 = ct{3486};
t582 = ct{3487};
t5823 = ct{3488};
t5826 = ct{3489};
t583 = ct{3490};
t584 = ct{3491};
t586 = ct{3492};
t587 = ct{3493};
t5886 = ct{3494};
t5887 = ct{3495};
t589 = ct{3496};
t5894 = ct{3497};
t59 = ct{3498};
t590 = ct{3499};
t591 = ct{3500};
t592 = ct{3501};
t593 = ct{3502};
t594 = ct{3503};
t595 = ct{3504};
t596 = ct{3505};
t597 = ct{3506};
t6 = ct{3507};
t60 = ct{3508};
t600 = ct{3509};
t602 = ct{3510};
t603 = ct{3511};
t604 = ct{3512};
t605 = ct{3513};
t609 = ct{3514};
t610 = ct{3515};
t611 = ct{3516};
t612 = ct{3517};
t613 = ct{3518};
t614 = ct{3519};
t615 = ct{3520};
t616 = ct{3521};
t618 = ct{3522};
t619 = ct{3523};
t620 = ct{3524};
t621 = ct{3525};
t622 = ct{3526};
t623 = ct{3527};
t624 = ct{3528};
t625 = ct{3529};
t626 = ct{3530};
t627 = ct{3531};
t628 = ct{3532};
t629 = ct{3533};
t63 = ct{3534};
t630 = ct{3535};
t631 = ct{3536};
t632 = ct{3537};
t633 = ct{3538};
t634 = ct{3539};
t635 = ct{3540};
t636 = ct{3541};
t637 = ct{3542};
t638 = ct{3543};
t639 = ct{3544};
t640 = ct{3545};
t641 = ct{3546};
t642 = ct{3547};
t643 = ct{3548};
t645 = ct{3549};
t646 = ct{3550};
t647 = ct{3551};
t648 = ct{3552};
t649 = ct{3553};
t650 = ct{3554};
t653 = ct{3555};
t654 = ct{3556};
t655 = ct{3557};
t656 = ct{3558};
t657 = ct{3559};
t658 = ct{3560};
t660 = ct{3561};
t662 = ct{3562};
t663 = ct{3563};
t664 = ct{3564};
t665 = ct{3565};
t667 = ct{3566};
t668 = ct{3567};
t669 = ct{3568};
t673 = ct{3569};
t674 = ct{3570};
t675 = ct{3571};
t676 = ct{3572};
t679 = ct{3573};
t680 = ct{3574};
t681 = ct{3575};
t682 = ct{3576};
t683 = ct{3577};
t684 = ct{3578};
t685 = ct{3579};
t686 = ct{3580};
t687 = ct{3581};
t688 = ct{3582};
t689 = ct{3583};
t691 = ct{3584};
t692 = ct{3585};
t693 = ct{3586};
t694 = ct{3587};
t695 = ct{3588};
t696 = ct{3589};
t697 = ct{3590};
t698 = ct{3591};
t7 = ct{3592};
t700 = ct{3593};
t702 = ct{3594};
t703 = ct{3595};
t704 = ct{3596};
t705 = ct{3597};
t706 = ct{3598};
t708 = ct{3599};
t71 = ct{3600};
t710 = ct{3601};
t711 = ct{3602};
t712 = ct{3603};
t713 = ct{3604};
t7148 = ct{3605};
t715 = ct{3606};
t716 = ct{3607};
t72 = ct{3608};
t724 = ct{3609};
t728 = ct{3610};
t73 = ct{3611};
t731 = ct{3612};
t733 = ct{3613};
t734 = ct{3614};
t735 = ct{3615};
t736 = ct{3616};
t738 = ct{3617};
t739 = ct{3618};
t74 = ct{3619};
t740 = ct{3620};
t741 = ct{3621};
t742 = ct{3622};
t743 = ct{3623};
t744 = ct{3624};
t746 = ct{3625};
t747 = ct{3626};
t748 = ct{3627};
t749 = ct{3628};
t75 = ct{3629};
t750 = ct{3630};
t751 = ct{3631};
t752 = ct{3632};
t753 = ct{3633};
t754 = ct{3634};
t755 = ct{3635};
t756 = ct{3636};
t757 = ct{3637};
t758 = ct{3638};
t759 = ct{3639};
t76 = ct{3640};
t760 = ct{3641};
t762 = ct{3642};
t763 = ct{3643};
t764 = ct{3644};
t765 = ct{3645};
t766 = ct{3646};
t767 = ct{3647};
t768 = ct{3648};
t769 = ct{3649};
t77 = ct{3650};
t772 = ct{3651};
t773 = ct{3652};
t774 = ct{3653};
t775 = ct{3654};
t776 = ct{3655};
t777 = ct{3656};
t778 = ct{3657};
t779 = ct{3658};
t780 = ct{3659};
t781 = ct{3660};
t782 = ct{3661};
t784 = ct{3662};
t785 = ct{3663};
t786 = ct{3664};
t792 = ct{3665};
t794 = ct{3666};
t795 = ct{3667};
t796 = ct{3668};
t797 = ct{3669};
t798 = ct{3670};
t799 = ct{3671};
t8 = ct{3672};
t80 = ct{3673};
t801 = ct{3674};
t802 = ct{3675};
t804 = ct{3676};
t805 = ct{3677};
t806 = ct{3678};
t808 = ct{3679};
t81 = ct{3680};
t814 = ct{3681};
t815 = ct{3682};
t817 = ct{3683};
t82 = ct{3684};
t820 = ct{3685};
t822 = ct{3686};
t823 = ct{3687};
t824 = ct{3688};
t825 = ct{3689};
t826 = ct{3690};
t827 = ct{3691};
t829 = ct{3692};
t83 = ct{3693};
t830 = ct{3694};
t831 = ct{3695};
t832 = ct{3696};
t833 = ct{3697};
t834 = ct{3698};
t835 = ct{3699};
t836 = ct{3700};
t837 = ct{3701};
t838 = ct{3702};
t84 = ct{3703};
t840 = ct{3704};
t841 = ct{3705};
t842 = ct{3706};
t843 = ct{3707};
t844 = ct{3708};
t845 = ct{3709};
t846 = ct{3710};
t847 = ct{3711};
t852 = ct{3712};
t853 = ct{3713};
t856 = ct{3714};
t858 = ct{3715};
t859 = ct{3716};
t86 = ct{3717};
t861 = ct{3718};
t863 = ct{3719};
t865 = ct{3720};
t866 = ct{3721};
t867 = ct{3722};
t868 = ct{3723};
t869 = ct{3724};
t870 = ct{3725};
t874 = ct{3726};
t875 = ct{3727};
t876 = ct{3728};
t877 = ct{3729};
t878 = ct{3730};
t880 = ct{3731};
t881 = ct{3732};
t882 = ct{3733};
t884 = ct{3734};
t885 = ct{3735};
t888 = ct{3736};
t891 = ct{3737};
t895 = ct{3738};
t899 = ct{3739};
t9 = ct{3740};
t90 = ct{3741};
t900 = ct{3742};
t902 = ct{3743};
t903 = ct{3744};
t906 = ct{3745};
t909 = ct{3746};
t91 = ct{3747};
t910 = ct{3748};
t911 = ct{3749};
t914 = ct{3750};
t916 = ct{3751};
t917 = ct{3752};
t920 = ct{3753};
t921 = ct{3754};
t922 = ct{3755};
t923 = ct{3756};
t925 = ct{3757};
t926 = ct{3758};
t927 = ct{3759};
t928 = ct{3760};
t929 = ct{3761};
t930 = ct{3762};
t934 = ct{3763};
t935 = ct{3764};
t937 = ct{3765};
t940 = ct{3766};
t941 = ct{3767};
t942 = ct{3768};
t943 = ct{3769};
t944 = ct{3770};
t945 = ct{3771};
t946 = ct{3772};
t947 = ct{3773};
t949 = ct{3774};
t95 = ct{3775};
t950 = ct{3776};
t951 = ct{3777};
t952 = ct{3778};
t953 = ct{3779};
t954 = ct{3780};
t955 = ct{3781};
t957 = ct{3782};
t958 = ct{3783};
t961 = ct{3784};
t962 = ct{3785};
t963 = ct{3786};
t964 = ct{3787};
t965 = ct{3788};
t968 = ct{3789};
t97 = ct{3790};
t970 = ct{3791};
t971 = ct{3792};
t972 = ct{3793};
t973 = ct{3794};
t974 = ct{3795};
t975 = ct{3796};
t976 = ct{3797};
t977 = ct{3798};
t982 = ct{3799};
t983 = ct{3800};
t984 = ct{3801};
t986 = ct{3802};
t987 = ct{3803};
t988 = ct{3804};
t989 = ct{3805};
t99 = ct{3806};
t991 = ct{3807};
t993 = ct{3808};
t994 = ct{3809};
t995 = ct{3810};
t999 = ct{3811};
t3923 = t2.*t202.*1.396693317797299e-6;
t3924 = t6.*t200.*1.396693317797299e-6;
t3925 = t6.*t201.*1.396693317797299e-6;
t3928 = -t3867;
t3931 = t9.*t201.*(-1.170967356229242e-5);
t3932 = t2.*t9.*t200.*3.96815841743287e-6;
t3934 = t2.*t5.*t202.*1.984079208716435e-6;
t3935 = t2.*t5.*t202.*3.96815841743287e-6;
t3937 = t5.*t6.*t200.*1.984079208716435e-6;
t3938 = t5.*t6.*t200.*3.96815841743287e-6;
t3939 = t5.*t6.*t201.*1.984079208716435e-6;
t3942 = t9.*t202.*(-1.170967356229242e-5);
t3945 = t8.*t3826;
t3947 = t8.*t3827;
t3954 = t6.*t202.*5.761404326386517e-6;
t3960 = t9.*t199.*3.182236832187144e-6;
t3962 = t5.*t200.*3.182236832187144e-6;
t3963 = t5.*t200.*6.364473664374288e-6;
t3964 = t5.*t201.*3.182236832187144e-6;
t3968 = t9.*t202.*3.182236832187144e-6;
t3971 = -t3929;
t3972 = -t3930;
t3974 = t2.*t9.*t201.*(-3.96815841743287e-6);
t3983 = -t3946;
t3985 = -t3949;
t3986 = t2.*t200.*5.761404326386517e-6;
t3987 = t2.*t201.*5.761404326386517e-6;
t3988 = t6.*t199.*5.761404326386517e-6;
t3989 = -t3952;
t3994 = -t3966;
t3995 = -t3970;
t3996 = -t3980;
t3997 = -t3981;
t4000 = t202.*9.240635641966378e-6;
t4003 = -t3990;
t4008 = t199.*6.530670357331468e-6;
t4009 = t199.*9.240635641966378e-6;
t4012 = -t4005;
t4013 = -t4006;
t4034 = -t4016;
t4035 = -t4021;
t4037 = -t4023;
t4038 = -t4027;
t4049 = t2.*t5.*t200.*1.857585372652597e-13;
t4050 = t2.*t5.*t201.*1.857585372652597e-13;
t4055 = t2.*t9.*t200.*1.857585372652597e-13;
t4056 = t2.*t9.*t201.*1.857585372652597e-13;
t4057 = t2.*t5.*t202.*1.857585372652597e-13;
t4059 = t2.*t9.*t202.*1.857585372652597e-13;
t4060 = t5.*t6.*t202.*1.857585372652597e-13;
t4061 = t6.*t9.*t202.*1.857585372652597e-13;
t4066 = -t4036;
t4067 = t6.*t9.*t202.*7.662598700988556e-13;
t4079 = -t4062;
t4080 = -t4063;
t4081 = t2.*t5.*t202.*7.662598700988556e-13;
t4082 = t5.*t6.*t200.*7.662598700988556e-13;
t4083 = t5.*t6.*t201.*7.662598700988556e-13;
t4084 = t2.*t9.*t202.*7.662598700988556e-13;
t4085 = t6.*t9.*t200.*7.662598700988556e-13;
t4086 = t6.*t9.*t201.*7.662598700988556e-13;
t4087 = t5.*t6.*t202.*7.662598700988556e-13;
t4090 = t5.*t200.*1.228993465050726e-12;
t4091 = t5.*t201.*1.228993465050726e-12;
t4092 = t9.*t200.*1.228993465050726e-12;
t4093 = t9.*t201.*1.228993465050726e-12;
t4094 = t5.*t202.*1.228993465050726e-12;
t4095 = t9.*t202.*1.228993465050726e-12;
t4097 = t199.*2.11749498538388e-7;
t4098 = t202.*2.11749498538388e-7;
t4100 = -t4089;
t4106 = t628+t1293;
t4108 = -t4099;
t4109 = t2.*t200.*1.796566294495167e-6;
t4110 = t2.*t201.*1.796566294495167e-6;
t4111 = t6.*t199.*1.796566294495167e-6;
t4112 = t6.*t202.*1.796566294495167e-6;
t4115 = -t4103;
t4120 = t627+t1334;
t4126 = t196+t2445;
t4127 = t2.*t199.*7.410893064247368e-6;
t4128 = t2.*t202.*7.410893064247368e-6;
t4129 = t6.*t200.*7.410893064247368e-6;
t4130 = t6.*t201.*7.410893064247368e-6;
t4133 = -t4125;
t4134 = t200.*5.943113753937517e-6;
t4135 = t200.*1.188622750787503e-5;
t4136 = t201.*1.188622750787503e-5;
t4139 = t631+t1398;
t4141 = t4119.^2;
t4147 = t5.*t4119;
t4148 = t9.*t4119;
t4149 = t630+t1422;
t4151 = -t4142;
t4154 = t202+t2461;
t4161 = t201+t2459;
t4378 = t8.*t4254;
t4536 = t18.*t4254;
t4585 = t8.*t4505;
t4648 = t18.*t4505;
t4816 = t199.*t3321;
t4817 = t5.*t34.*t191.*t201.*7.651846806710377e-23;
t4822 = t7.*t34.*t191.*t199.*3.991434681284372e-24;
t4823 = t202.*t3321;
t4843 = t34.*t191.*t200.*1.678396953782234e-24;
t4844 = t34.*t191.*t201.*1.678396953782234e-24;
t4850 = t7.*t9.*t34.*t191.*t200.*1.8197034170822e-22;
t4854 = t5.*t9.*t34.*t191.*t199.*1.564233326885588e-22;
t4855 = -t4821;
t4858 = t9.*t34.*t191.*t202.*(-7.651846806710377e-23);
t4859 = t5.*t9.*t34.*t191.*t202.*1.564233326885588e-22;
t4881 = t5.*t9.*t34.*t191.*t201.*4.759540657477059e-22;
t4889 = t19.*t34.*t191.*t201.*1.564233326885588e-22;
t4890 = t24.*t34.*t191.*t201.*1.564233326885588e-22;
t4894 = -t4847;
t4896 = t19.*t34.*t191.*t199.*2.379770328738529e-22;
t4898 = t7.*t19.*t34.*t191.*t200.*5.659386953851025e-22;
t4901 = t8.*t9.*t34.*t191.*t199.*1.530369361342075e-22;
t4902 = t5.*t8.*t34.*t191.*t201.*1.530369361342075e-22;
t4905 = t19.*t34.*t191.*t202.*2.379770328738529e-22;
t4906 = -t4851;
t4926 = t18.*t4793;
t4932 = -t4874;
t4939 = -t4880;
t4947 = t5.*t7.*t9.*t34.*t191.*t200.*3.719939515191737e-22;
t4954 = t199.*t3382;
t4959 = t5.*t7.*t34.*t191.*t200.*9.890501569818525e-23;
t4960 = t9.*t34.*t191.*t201.*4.158952615208568e-23;
t4961 = t202.*t3382;
t4965 = t5.*t7.*t8.*t34.*t191.*t199.*1.8197034170822e-22;
t4966 = t44.*t4119;
t4967 = t45.*t4119;
t4971 = t47.*t4119;
t4984 = -t4904;
t5013 = t5.*t8.*t9.*t34.*t191.*t201.*2.379770328738529e-22;
t5028 = t5.*t34.*t191.*t199.*(-4.158952615208568e-23);
t5037 = t5.*t34.*t191.*t202.*(-4.158952615208568e-23);
t5047 = t8.*t24.*t34.*t191.*t199.*2.379770328738529e-22;
t5057 = t5.*t8.*t9.*t34.*t191.*t199.*3.128466653771177e-22;
t5068 = t7.*t34.*t191.*t200.*2.82396378095488e-22;
t5079 = t5.*t7.*t8.*t9.*t34.*t191.*t199.*2.829693476925513e-22;
t5086 = t57.*t4119;
t5087 = t58.*t4119;
t5092 = t60.*t4119;
t5094 = t5.*t8.*t34.*t191.*t199.*8.317905230417136e-23;
t5103 = t7.*t8.*t9.*t34.*t191.*t199.*9.890501569818525e-23;
t5104 = t8.*t9.*t34.*t191.*t201.*8.317905230417136e-23;
t5105 = -t5030;
t5115 = t63.*t4119;
t5117 = t8.*t19.*t34.*t191.*t199.*(-2.379770328738529e-22);
t5118 = -t5041;
t5124 = t7.*t8.*t19.*t34.*t191.*t199.*1.859969757595868e-22;
t5126 = -t5048;
t5128 = t34.*t191.*t199.*1.187475829122392e-22;
t5133 = -t5054;
t5134 = -t5059;
t5135 = t18.*t4847;
t5137 = t34.*t191.*t202.*1.187475829122392e-22;
t5141 = -t5067;
t5156 = -t5081;
t5159 = t5.*t34.*t191.*t200.*3.002769355787804e-29;
t5160 = t5.*t34.*t191.*t201.*3.002769355787804e-29;
t5161 = t71.*t4119;
t5162 = t72.*t4119;
t5167 = t74.*t4119;
t5173 = t9.*t34.*t191.*t202.*3.002769355787804e-29;
t5177 = t75.*t4119;
t5182 = t76.*t4119;
t5188 = t77.*t4119;
t5190 = t82.*t4119;
t5194 = t83.*t4119;
t5197 = -t5125;
t5198 = t84.*t4119;
t5213 = -t5138;
t5214 = t5.*t7.*t34.*t191.*t199.*7.140955373864693e-29;
t5220 = -t5152;
t5221 = -t5153;
t5225 = t8.*t9.*t34.*t191.*t199.*1.201107742315122e-28;
t5226 = t97.*t4119;
t5243 = t8.*t34.*t191.*t201.*5.632647031707275e-23;
t5274 = t111.*t4119;
t5275 = t112.*t4119;
t5276 = t9.*t34.*t191.*t200.*3.937746659416635e-29;
t5277 = t9.*t34.*t191.*t201.*3.937746659416635e-29;
t5278 = t5.*t34.*t191.*t202.*3.937746659416635e-29;
t5283 = t120.*t4119;
t5287 = t101.*t4119;
t5291 = t102.*t4119;
t5298 = -t5257;
t5300 = t110.*t4119;
t5303 = -t5268;
t5304 = t5.*t7.*t8.*t34.*t191.*t199.*3.570477686932346e-29;
t5308 = -t5272;
t5310 = t4.*t4119.*(-1.758766830582798e-8);
t5317 = t128.*t4119;
t5322 = t129.*t4119;
t5326 = -t5288;
t5329 = t7.*t8.*t34.*t191.*t199.*6.697564202296239e-23;
t5330 = -t5292;
t5334 = t124.*t4119;
t5336 = t5.*t8.*t34.*t191.*t199.*1.575098663766654e-28;
t5341 = t7.*t9.*t34.*t191.*t199.*9.364446561398189e-29;
t5359 = t139.*t4119;
t5360 = t140.*t4119;
t5363 = t142.*t4119;
t5374 = t7.*t8.*t9.*t34.*t191.*t199.*4.682223280699094e-29;
t5386 = -t5365;
t5388 = -t5367;
t5400 = t157.*t4119;
t5406 = t150.*t4119;
t5407 = t151.*t4119;
t5408 = t154.*t4119;
t5411 = t165.*t4119;
t5413 = t161.*t4119;
t5417 = t163.*t4119;
t5425 = t170.*t4119;
t5437 = t8.*t34.*t191.*t199.*2.783302668250669e-22;
t5438 = t177.*t4119;
t5460 = -t5444;
t5461 = -t5446;
t5462 = -t5448;
t5495 = t9.*t34.*t191.*t199.*7.82072115054759e-23;
t5500 = t5.*t34.*t191.*t199.*7.316193564301157e-22;
t5502 = t9.*t34.*t191.*t200.*7.316193564301157e-22;
t5503 = t5.*t34.*t191.*t202.*7.316193564301157e-22;
t5504 = t1480+t2469;
t5505 = t34.*t191.*t200.*1.715438754464886e-24;
t5506 = -t5496;
t5513 = t5.*t9.*t34.*t191.*t199.*1.598755564896737e-22;
t5514 = t9.*t34.*t191.*t202.*3.976517450785667e-22;
t5518 = t19.*t34.*t191.*t199.*2.432291264259161e-22;
t5520 = t5.*t34.*t191.*t199.*4.25073965847863e-23;
t5523 = t5.*t8.*t34.*t191.*t201.*1.564144230109518e-22;
t5524 = t9.*t34.*t191.*t199.*3.976517450785667e-22;
t5525 = t5.*t34.*t191.*t200.*3.976517450785667e-22;
t5528 = t7.*t34.*t191.*t199.*4.9251280219403e-24;
t5531 = t34.*t191.*t199.*5.773540880892919e-22;
t5533 = t34.*t191.*t202.*5.773540880892919e-22;
t5536 = -t5522;
